simulink model "controllo_cartesiano"  (R2020b)
(part 3 of 5)

dxc5*((l*cos(2*atan((2*l^2*sin(q2) + (3*l^4 + 4*cos(q2)*l^3*xc1 - 4*sin(q2)*l^3*xc5 - 2*cos(2*q2)*l^2*xc1^2 + 4*sin(2*q2)*l^2*xc1*xc5 + 2*cos(2*q2)*l^2*xc5^2 - 4*cos(q2)*l*xc1^3 + 4*sin(q2)*l*xc1^2*xc5 - 4*cos(q2)*l*xc1*xc5^2 + 4*sin(q2)*l*xc5^3 - xc1^4 - 2*xc1^2*xc5^2 - xc5^4)^(1/2) - 2*l*xc5)/(l^2 - 2*l*xc1 + xc1^2 + xc5^2 - 2*l^2*cos(q2) + 2*l*xc1*cos(q2) - 2*l*xc5*sin(q2))))*(((cos(q2) + 1)^2*(2*xc1 - 4*l*tan(q2/2)^2 + 2*xc1*tan(q2/2)^2)*(2*l + 2*l*tan(q2/2)^2 - ((2*xc5 - 2*l*sin(q2))*(l^2 + 2*cos(q2)*l*xc1 - 2*sin(q2)*l*xc5 + xc1^2 + xc5^2) + (2*xc5 - 2*l*sin(q2))*(- 3*l^2 + 2*cos(q2)*l*xc1 - 2*sin(q2)*l*xc5 + xc1^2 + xc5^2))/((cos(q2) + 1)*(-(l^2 + 2*cos(q2)*l*xc1 - 2*sin(q2)*l*xc5 + xc1^2 + xc5^2)*(- 3*l^2 + 2*cos(q2)*l*xc1 - 2*sin(q2)*l*xc5 + xc1^2 + xc5^2))^(1/2))))/(4*(l^2 - 2*l*xc1 + xc1^2 + xc5^2 - 2*l^2*cos(q2) + 2*l*xc1*cos(q2) - 2*l*xc5*sin(q2))^2) + (2*(xc1 + l*cos(q2))*(2*xc5 - 2*l*sin(q2)))/((-(l^2 + 2*cos(q2)*l*xc1 - 2*sin(q2)*l*xc5 + xc1^2 + xc5^2)*(- 3*l^2 + 2*cos(q2)*l*xc1 - 2*sin(q2)*l*xc5 + xc1^2 + xc5^2))^(1/2)*(l^2 - 2*l*xc1 + xc1^2 + xc5^2 - 2*l^2*cos(q2) + 2*l*xc1*cos(q2) - 2*l*xc5*sin(q2))) - (l*(tan(q2/2)^2 + 1)*(cos(q2) + 1)^2*(2*xc1 - 4*l*tan(q2/2)^2 + 2*xc1*tan(q2/2)^2))/(l^2 - 2*l*xc1 + xc1^2 + xc5^2 - 2*l^2*cos(q2) + 2*l*xc1*cos(q2) - 2*l*xc5*sin(q2))^2 - (2*(xc1 + l*cos(q2))*(2*xc5 - 2*l*sin(q2))*(- l^2 + 2*cos(q2)*l*xc1 - 2*sin(q2)*l*xc5 + xc1^2 + xc5^2))/((-(l^2 + 2*cos(q2)*l*xc1 - 2*sin(q2)*l*xc5 + xc1^2 + xc5^2)*(- 3*l^2 + 2*cos(q2)*l*xc1 - 2*sin(q2)*l*xc5 + xc1^2 + xc5^2))^(1/2)*(l^2 - 2*l*xc1 + xc1^2 + xc5^2 - 2*l^2*cos(q2) + 2*l*xc1*cos(q2) - 2*l*xc5*sin(q2))^2) + ((xc1 + l*cos(q2))*((2*xc5 - 2*l*sin(q2))*(l^2 + 2*cos(q2)*l*xc1 - 2*sin(q2)*l*xc5 + xc1^2 + xc5^2) + (2*xc5 - 2*l*sin(q2))*(- 3*l^2 + 2*cos(q2)*l*xc1 - 2*sin(q2)*l*xc5 + xc1^2 + xc5^2))*(- l^2 + 2*cos(q2)*l*xc1 - 2*sin(q2)*l*xc5 + xc1^2 + xc5^2))/((-(l^2 + 2*cos(q2)*l*xc1 - 2*sin(q2)*l*xc5 + xc1^2 + xc5^2)*(- 3*l^2 + 2*cos(q2)*l*xc1 - 2*sin(q2)*l*xc5 + xc1^2 + xc5^2))^(3/2)*(l^2 - 2*l*xc1 + xc1^2 + xc5^2 - 2*l^2*cos(q2) + 2*l*xc1*cos(q2) - 2*l*xc5*sin(q2))) - ((cos(q2) + 1)^2*(2*xc5 - 2*l*sin(q2))*(2*xc1 - 4*l*tan(q2/2)^2 + 2*xc1*tan(q2/2)^2)*(2*l*xc5 + (2*(-(l^2 + 2*cos(q2)*l*xc1 - 2*sin(q2)*l*xc5 + xc1^2 + xc5^2)*(- 3*l^2 + 2*cos(q2)*l*xc1 - 2*sin(q2)*l*xc5 + xc1^2 + xc5^2))^(1/2))/(cos(q2) + 1) - 4*l^2*tan(q2/2) + 2*l*xc5*tan(q2/2)^2))/(2*(l^2 - 2*l*xc1 + xc1^2 + xc5^2 - 2*l^2*cos(q2) + 2*l*xc1*cos(q2) - 2*l*xc5*sin(q2))^3) + (2*l*(cos(q2) + 1)^2*(2*xc5 - 2*l*sin(q2))*(2*xc1 - 4*l*tan(q2/2)^2 + 2*xc1*tan(q2/2)^2)*(xc5*tan(q2/2)^2 - 2*l*tan(q2/2) + xc5))/(l^2 - 2*l*xc1 + xc1^2 + xc5^2 - 2*l^2*cos(q2) + 2*l*xc1*cos(q2) - 2*l*xc5*sin(q2))^3))/(((cos(q2) + 1)^2*(2*l*xc5 - (2*(-(l^2 + 2*cos(q2)*l*xc1 - 2*sin(q2)*l*xc5 + xc1^2 + xc5^2)*(- 3*l^2 + 2*cos(q2)*l*xc1 - 2*sin(q2)*l*xc5 + xc1^2 + xc5^2))^(1/2))/(cos(q2) + 1) - 4*l^2*tan(q2/2) + 2*l*xc5*tan(q2/2)^2)^2)/(4*(l^2 - 2*l*xc1 + xc1^2 + xc5^2 - 2*l^2*cos(q2) + 2*l*xc1*cos(q2) - 2*l*xc5*sin(q2))^2) + 1) + (l*cos(2*atan((2*l^2*sin(q2) + (3*l^4 + 4*cos(q2)*l^3*xc1 - 4*sin(q2)*l^3*xc5 - 2*cos(2*q2)*l^2*xc1^2 + 4*sin(2*q2)*l^2*xc1*xc5 + 2*cos(2*q2)*l^2*xc5^2 - 4*cos(q2)*l*xc1^3 + 4*sin(q2)*l*xc1^2*xc5 - 4*cos(q2)*l*xc1*xc5^2 + 4*sin(q2)*l*xc5^3 - xc1^4 - 2*xc1^2*xc5^2 - xc5^4)^(1/2) - 2*l*xc5)/(l^2 - 2*l*xc1 + xc1^2 + xc5^2 - 2*l^2*cos(q2) + 2*l*xc1*cos(q2) - 2*l*xc5*sin(q2))))*(((cos(q2) + 1)^2*(2*xc5 - 2*l*sin(q2))*(2*l*xc5 - (2*(-(l^2 + 2*cos(q2)*l*xc1 - 2*sin(q2)*l*xc5 + xc1^2 + xc5^2)*(- 3*l^2 + 2*cos(q2)*l*xc1 - 2*sin(q2)*l*xc5 + xc1^2 + xc5^2))^(1/2))/(cos(q2) + 1) - 4*l^2*tan(q2/2) + 2*l*xc5*tan(q2/2)^2)^2)/(2*(l^2 - 2*l*xc1 + xc1^2 + xc5^2 - 2*l^2*cos(q2) + 2*l*xc1*cos(q2) - 2*l*xc5*sin(q2))^3) - ((cos(q2) + 1)^2*(2*l + 2*l*tan(q2/2)^2 + ((2*xc5 - 2*l*sin(q2))*(l^2 + 2*cos(q2)*l*xc1 - 2*sin(q2)*l*xc5 + xc1^2 + xc5^2) + (2*xc5 - 2*l*sin(q2))*(- 3*l^2 + 2*cos(q2)*l*xc1 - 2*sin(q2)*l*xc5 + xc1^2 + xc5^2))/((cos(q2) + 1)*(-(l^2 + 2*cos(q2)*l*xc1 - 2*sin(q2)*l*xc5 + xc1^2 + xc5^2)*(- 3*l^2 + 2*cos(q2)*l*xc1 - 2*sin(q2)*l*xc5 + xc1^2 + xc5^2))^(1/2)))*(2*l*xc5 - (2*(-(l^2 + 2*cos(q2)*l*xc1 - 2*sin(q2)*l*xc5 + xc1^2 + xc5^2)*(- 3*l^2 + 2*cos(q2)*l*xc1 - 2*sin(q2)*l*xc5 + xc1^2 + xc5^2))^(1/2))/(cos(q2) + 1) - 4*l^2*tan(q2/2) + 2*l*xc5*tan(q2/2)^2))/(2*(l^2 - 2*l*xc1 + xc1^2 + xc5^2 - 2*l^2*cos(q2) + 2*l*xc1*cos(q2) - 2*l*xc5*sin(q2))^2))*(((cos(q2) + 1)^2*(2*xc1 - 4*l*tan(q2/2)^2 + 2*xc1*tan(q2/2)^2)*(2*l*xc5 + (2*(-(l^2 + 2*cos(q2)*l*xc1 - 2*sin(q2)*l*xc5 + xc1^2 + xc5^2)*(- 3*l^2 + 2*cos(q2)*l*xc1 - 2*sin(q2)*l*xc5 + xc1^2 + xc5^2))^(1/2))/(cos(q2) + 1) - 4*l^2*tan(q2/2) + 2*l*xc5*tan(q2/2)^2))/(4*(l^2 - 2*l*xc1 + xc1^2 + xc5^2 - 2*l^2*cos(q2) + 2*l*xc1*cos(q2) - 2*l*xc5*sin(q2))^2) + (2*(xc1 + l*cos(q2))*(- l^2 + 2*cos(q2)*l*xc1 - 2*sin(q2)*l*xc5 + xc1^2 + xc5^2))/((-(l^2 + 2*cos(q2)*l*xc1 - 2*sin(q2)*l*xc5 + xc1^2 + xc5^2)*(- 3*l^2 + 2*cos(q2)*l*xc1 - 2*sin(q2)*l*xc5 + xc1^2 + xc5^2))^(1/2)*(l^2 - 2*l*xc1 + xc1^2 + xc5^2 - 2*l^2*cos(q2) + 2*l*xc1*cos(q2) - 2*l*xc5*sin(q2))) - (l*(cos(q2) + 1)^2*(2*xc1 - 4*l*tan(q2/2)^2 + 2*xc1*tan(q2/2)^2)*(xc5*tan(q2/2)^2 - 2*l*tan(q2/2) + xc5))/(l^2 - 2*l*xc1 + xc1^2 + xc5^2 - 2*l^2*cos(q2) + 2*l*xc1*cos(q2) - 2*l*xc5*sin(q2))^2))/(((cos(q2) + 1)^2*(2*l*xc5 - (2*(-(l^2 + 2*cos(q2)*l*xc1 - 2*sin(q2)*l*xc5 + xc1^2 + xc5^2)*(- 3*l^2 + 2*cos(q2)*l*xc1 - 2*sin(q2)*l*xc5 + xc1^2 + xc5^2))^(1/2))/(cos(q2) + 1) - 4*l^2*tan(q2/2) + 2*l*xc5*tan(q2/2)^2)^2)/(4*(l^2 - 2*l*xc1 + xc1^2 + xc5^2 - 2*l^2*cos(q2) + 2*l*xc1*cos(q2) - 2*l*xc5*sin(q2))^2) + 1)^2 + (2*l*sin(2*atan((2*l^2*sin(q2) + (3*l^4 + 4*cos(q2)*l^3*xc1 - 4*sin(q2)*l^3*xc5 - 2*cos(2*q2)*l^2*xc1^2 + 4*sin(2*q2)*l^2*xc1*xc5 + 2*cos(2*q2)*l^2*xc5^2 - 4*cos(q2)*l*xc1^3 + 4*sin(q2)*l*xc1^2*xc5 - 4*cos(q2)*l*xc1*xc5^2 + 4*sin(q2)*l*xc5^3 - xc1^4 - 2*xc1^2*xc5^2 - xc5^4)^(1/2) - 2*l*xc5)/(l^2 - 2*l*xc1 + xc1^2 + xc5^2 - 2*l^2*cos(q2) + 2*l*xc1*cos(q2) - 2*l*xc5*sin(q2))))*((2*l + (4*sin(q2)*l^3 - 4*sin(2*q2)*l^2*xc1 - 4*cos(2*q2)*l^2*xc5 - 4*sin(q2)*l*xc1^2 + 8*cos(q2)*l*xc1*xc5 - 12*sin(q2)*l*xc5^2 + 4*xc1^2*xc5 + 4*xc5^3)/(2*(3*l^4 + 4*cos(q2)*l^3*xc1 - 4*sin(q2)*l^3*xc5 - 2*cos(2*q2)*l^2*xc1^2 + 4*sin(2*q2)*l^2*xc1*xc5 + 2*cos(2*q2)*l^2*xc5^2 - 4*cos(q2)*l*xc1^3 + 4*sin(q2)*l*xc1^2*xc5 - 4*cos(q2)*l*xc1*xc5^2 + 4*sin(q2)*l*xc5^3 - xc1^4 - 2*xc1^2*xc5^2 - xc5^4)^(1/2)))/(l^2 - 2*l*xc1 + xc1^2 + xc5^2 - 2*l^2*cos(q2) + 2*l*xc1*cos(q2) - 2*l*xc5*sin(q2)) + ((2*xc5 - 2*l*sin(q2))*(2*l^2*sin(q2) + (3*l^4 + 4*cos(q2)*l^3*xc1 - 4*sin(q2)*l^3*xc5 - 2*cos(2*q2)*l^2*xc1^2 + 4*sin(2*q2)*l^2*xc1*xc5 + 2*cos(2*q2)*l^2*xc5^2 - 4*cos(q2)*l*xc1^3 + 4*sin(q2)*l*xc1^2*xc5 - 4*cos(q2)*l*xc1*xc5^2 + 4*sin(q2)*l*xc5^3 - xc1^4 - 2*xc1^2*xc5^2 - xc5^4)^(1/2) - 2*l*xc5))/(l^2 - 2*l*xc1 + xc1^2 + xc5^2 - 2*l^2*cos(q2) + 2*l*xc1*cos(q2) - 2*l*xc5*sin(q2))^2)*(((cos(q2) + 1)^2*(2*xc1 - 4*l*tan(q2/2)^2 + 2*xc1*tan(q2/2)^2)*(2*l*xc5 + (2*(-(l^2 + 2*cos(q2)*l*xc1 - 2*sin(q2)*l*xc5 + xc1^2 + xc5^2)*(- 3*l^2 + 2*cos(q2)*l*xc1 - 2*sin(q2)*l*xc5 + xc1^2 + xc5^2))^(1/2))/(cos(q2) + 1) - 4*l^2*tan(q2/2) + 2*l*xc5*tan(q2/2)^2))/(4*(l^2 - 2*l*xc1 + xc1^2 + xc5^2 - 2*l^2*cos(q2) + 2*l*xc1*cos(q2) - 2*l*xc5*sin(q2))^2) + (2*(xc1 + l*cos(q2))*(- l^2 + 2*cos(q2)*l*xc1 - 2*sin(q2)*l*xc5 + xc1^2 + xc5^2))/((-(l^2 + 2*cos(q2)*l*xc1 - 2*sin(q2)*l*xc5 + xc1^2 + xc5^2)*(- 3*l^2 + 2*cos(q2)*l*xc1 - 2*sin(q2)*l*xc5 + xc1^2 + xc5^2))^(1/2)*(l^2 - 2*l*xc1 + xc1^2 + xc5^2 - 2*l^2*cos(q2) + 2*l*xc1*cos(q2) - 2*l*xc5*sin(q2))) - (l*(cos(q2) + 1)^2*(2*xc1 - 4*l*tan(q2/2)^2 + 2*xc1*tan(q2/2)^2)*(xc5*tan(q2/2)^2 - 2*l*tan(q2/2) + xc5))/(l^2 - 2*l*xc1 + xc1^2 + xc5^2 - 2*l^2*cos(q2) + 2*l*xc1*cos(q2) - 2*l*xc5*sin(q2))^2))/(((2*l^2*sin(q2) + (3*l^4 + 4*cos(q2)*l^3*xc1 - 4*sin(q2)*l^3*xc5 - 2*cos(2*q2)*l^2*xc1^2 + 4*sin(2*q2)*l^2*xc1*xc5 + 2*cos(2*q2)*l^2*xc5^2 - 4*cos(q2)*l*xc1^3 + 4*sin(q2)*l*xc1^2*xc5 - 4*cos(q2)*l*xc1*xc5^2 + 4*sin(q2)*l*xc5^3 - xc1^4 - 2*xc1^2*xc5^2 - xc5^4)^(1/2) - 2*l*xc5)^2/(l^2 - 2*l*xc1 + xc1^2 + xc5^2 - 2*l^2*cos(q2) + 2*l*xc1*cos(q2) - 2*l*xc5*sin(q2))^2 + 1)*(((cos(q2) + 1)^2*(2*l*xc5 - (2*(-(l^2 + 2*cos(q2)*l*xc1 - 2*sin(q2)*l*xc5 + xc1^2 + xc5^2)*(- 3*l^2 + 2*cos(q2)*l*xc1 - 2*sin(q2)*l*xc5 + xc1^2 + xc5^2))^(1/2))/(cos(q2) + 1) - 4*l^2*tan(q2/2) + 2*l*xc5*tan(q2/2)^2)^2)/(4*(l^2 - 2*l*xc1 + xc1^2 + xc5^2 - 2*l^2*cos(q2) + 2*l*xc1*cos(q2) - 2*l*xc5*sin(q2))^2) + 1))) + dq2*((l*cos(2*atan((2*l^2*sin(q2) + (3*l^4 + 4*cos(q2)*l^3*xc1 - 4*sin(q2)*l^3*xc5 - 2*cos(2*q2)*l^2*xc1^2 + 4*sin(2*q2)*l^2*xc1*xc5 + 2*cos(2*q2)*l^2*xc5^2 - 4*cos(q2)*l*xc1^3 + 4*sin(q2)*l*xc1^2*xc5 - 4*cos(q2)*l*xc1*xc5^2 + 4*sin(q2)*l*xc5^3 - xc1^4 - 2*xc1^2*xc5^2 - xc5^4)^(1/2) - 2*l*xc5)/(l^2 - 2*l*xc1 + xc1^2 + xc5^2 - 2*l^2*cos(q2) + 2*l*xc1*cos(q2) - 2*l*xc5*sin(q2))))*(((cos(q2) + 1)^2*(2*xc1 - 4*l*tan(q2/2)^2 + 2*xc1*tan(q2/2)^2)*((2*sin(q2)*(-(l^2 + 2*cos(q2)*l*xc1 - 2*sin(q2)*l*xc5 + xc1^2 + xc5^2)*(- 3*l^2 + 2*cos(q2)*l*xc1 - 2*sin(q2)*l*xc5 + xc1^2 + xc5^2))^(1/2))/(cos(q2) + 1)^2 - 4*l^2*(tan(q2/2)^2/2 + 1/2) + ((2*l*xc5*cos(q2) + 2*l*xc1*sin(q2))*(l^2 + 2*cos(q2)*l*xc1 - 2*sin(q2)*l*xc5 + xc1^2 + xc5^2) + (2*l*xc5*cos(q2) + 2*l*xc1*sin(q2))*(- 3*l^2 + 2*cos(q2)*l*xc1 - 2*sin(q2)*l*xc5 + xc1^2 + xc5^2))/((cos(q2) + 1)*(-(l^2 + 2*cos(q2)*l*xc1 - 2*sin(q2)*l*xc5 + xc1^2 + xc5^2)*(- 3*l^2 + 2*cos(q2)*l*xc1 - 2*sin(q2)*l*xc5 + xc1^2 + xc5^2))^(1/2)) + 4*l*xc5*tan(q2/2)*(tan(q2/2)^2/2 + 1/2)))/(4*(l^2 - 2*l*xc1 + xc1^2 + xc5^2 - 2*l^2*cos(q2) + 2*l*xc1*cos(q2) - 2*l*xc5*sin(q2))^2) - ((cos(q2) + 1)^2*(8*l*tan(q2/2)*(tan(q2/2)^2/2 + 1/2) - 4*xc1*tan(q2/2)*(tan(q2/2)^2/2 + 1/2))*(2*l*xc5 + (2*(-(l^2 + 2*cos(q2)*l*xc1 - 2*sin(q2)*l*xc5 + xc1^2 + xc5^2)*(- 3*l^2 + 2*cos(q2)*l*xc1 - 2*sin(q2)*l*xc5 + xc1^2 + xc5^2))^(1/2))/(cos(q2) + 1) - 4*l^2*tan(q2/2) + 2*l*xc5*tan(q2/2)^2))/(4*(l^2 - 2*l*xc1 + xc1^2 + xc5^2 - 2*l^2*cos(q2) + 2*l*xc1*cos(q2) - 2*l*xc5*sin(q2))^2) - (2*(xc1 + l*cos(q2))*(2*l*xc5*cos(q2) + 2*l*xc1*sin(q2)))/((-(l^2 + 2*cos(q2)*l*xc1 - 2*sin(q2)*l*xc5 + xc1^2 + xc5^2)*(- 3*l^2 + 2*cos(q2)*l*xc1 - 2*sin(q2)*l*xc5 + xc1^2 + xc5^2))^(1/2)*(l^2 - 2*l*xc1 + xc1^2 + xc5^2 - 2*l^2*cos(q2) + 2*l*xc1*cos(q2) - 2*l*xc5*sin(q2))) + (2*(xc1 + l*cos(q2))*(2*l*xc5*cos(q2) - 2*l^2*sin(q2) + 2*l*xc1*sin(q2))*(- l^2 + 2*cos(q2)*l*xc1 - 2*sin(q2)*l*xc5 + xc1^2 + xc5^2))/((-(l^2 + 2*cos(q2)*l*xc1 - 2*sin(q2)*l*xc5 + xc1^2 + xc5^2)*(- 3*l^2 + 2*cos(q2)*l*xc1 - 2*sin(q2)*l*xc5 + xc1^2 + xc5^2))^(1/2)*(l^2 - 2*l*xc1 + xc1^2 + xc5^2 - 2*l^2*cos(q2) + 2*l*xc1*cos(q2) - 2*l*xc5*sin(q2))^2) - (2*l*sin(q2)*(- l^2 + 2*cos(q2)*l*xc1 - 2*sin(q2)*l*xc5 + xc1^2 + xc5^2))/((-(l^2 + 2*cos(q2)*l*xc1 - 2*sin(q2)*l*xc5 + xc1^2 + xc5^2)*(- 3*l^2 + 2*cos(q2)*l*xc1 - 2*sin(q2)*l*xc5 + xc1^2 + xc5^2))^(1/2)*(l^2 - 2*l*xc1 + xc1^2 + xc5^2 - 2*l^2*cos(q2) + 2*l*xc1*cos(q2) - 2*l*xc5*sin(q2))) + (l*(2*l*(tan(q2/2)^2/2 + 1/2) - 2*xc5*tan(q2/2)*(tan(q2/2)^2/2 + 1/2))*(cos(q2) + 1)^2*(2*xc1 - 4*l*tan(q2/2)^2 + 2*xc1*tan(q2/2)^2))/(l^2 - 2*l*xc1 + xc1^2 + xc5^2 - 2*l^2*cos(q2) + 2*l*xc1*cos(q2) - 2*l*xc5*sin(q2))^2 - ((xc1 + l*cos(q2))*((2*l*xc5*cos(q2) + 2*l*xc1*sin(q2))*(l^2 + 2*cos(q2)*l*xc1 - 2*sin(q2)*l*xc5 + xc1^2 + xc5^2) + (2*l*xc5*cos(q2) + 2*l*xc1*sin(q2))*(- 3*l^2 + 2*cos(q2)*l*xc1 - 2*sin(q2)*l*xc5 + xc1^2 + xc5^2))*(- l^2 + 2*cos(q2)*l*xc1 - 2*sin(q2)*l*xc5 + xc1^2 + xc5^2))/((-(l^2 + 2*cos(q2)*l*xc1 - 2*sin(q2)*l*xc5 + xc1^2 + xc5^2)*(- 3*l^2 + 2*cos(q2)*l*xc1 - 2*sin(q2)*l*xc5 + xc1^2 + xc5^2))^(3/2)*(l^2 - 2*l*xc1 + xc1^2 + xc5^2 - 2*l^2*cos(q2) + 2*l*xc1*cos(q2) - 2*l*xc5*sin(q2))) - (sin(q2)*(cos(q2) + 1)*(2*xc1 - 4*l*tan(q2/2)^2 + 2*xc1*tan(q2/2)^2)*(2*l*xc5 + (2*(-(l^2 + 2*cos(q2)*l*xc1 - 2*sin(q2)*l*xc5 + xc1^2 + xc5^2)*(- 3*l^2 + 2*cos(q2)*l*xc1 - 2*sin(q2)*l*xc5 + xc1^2 + xc5^2))^(1/2))/(cos(q2) + 1) - 4*l^2*tan(q2/2) + 2*l*xc5*tan(q2/2)^2))/(2*(l^2 - 2*l*xc1 + xc1^2 + xc5^2 - 2*l^2*cos(q2) + 2*l*xc1*cos(q2) - 2*l*xc5*sin(q2))^2) + ((cos(q2) + 1)^2*(2*xc1 - 4*l*tan(q2/2)^2 + 2*xc1*tan(q2/2)^2)*(2*l*xc5*cos(q2) - 2*l^2*sin(q2) + 2*l*xc1*sin(q2))*(2*l*xc5 + (2*(-(l^2 + 2*cos(q2)*l*xc1 - 2*sin(q2)*l*xc5 + xc1^2 + xc5^2)*(- 3*l^2 + 2*cos(q2)*l*xc1 - 2*sin(q2)*l*xc5 + xc1^2 + xc5^2))^(1/2))/(cos(q2) + 1) - 4*l^2*tan(q2/2) + 2*l*xc5*tan(q2/2)^2))/(2*(l^2 - 2*l*xc1 + xc1^2 + xc5^2 - 2*l^2*cos(q2) + 2*l*xc1*cos(q2) - 2*l*xc5*sin(q2))^3) + (l*(cos(q2) + 1)^2*(8*l*tan(q2/2)*(tan(q2/2)^2/2 + 1/2) - 4*xc1*tan(q2/2)*(tan(q2/2)^2/2 + 1/2))*(xc5*tan(q2/2)^2 - 2*l*tan(q2/2) + xc5))/(l^2 - 2*l*xc1 + xc1^2 + xc5^2 - 2*l^2*cos(q2) + 2*l*xc1*cos(q2) - 2*l*xc5*sin(q2))^2 + (2*l*sin(q2)*(cos(q2) + 1)*(2*xc1 - 4*l*tan(q2/2)^2 + 2*xc1*tan(q2/2)^2)*(xc5*tan(q2/2)^2 - 2*l*tan(q2/2) + xc5))/(l^2 - 2*l*xc1 + xc1^2 + xc5^2 - 2*l^2*cos(q2) + 2*l*xc1*cos(q2) - 2*l*xc5*sin(q2))^2 - (2*l*(cos(q2) + 1)^2*(2*xc1 - 4*l*tan(q2/2)^2 + 2*xc1*tan(q2/2)^2)*(xc5*tan(q2/2)^2 - 2*l*tan(q2/2) + xc5)*(2*l*xc5*cos(q2) - 2*l^2*sin(q2) + 2*l*xc1*sin(q2)))/(l^2 - 2*l*xc1 + xc1^2 + xc5^2 - 2*l^2*cos(q2) + 2*l*xc1*cos(q2) - 2*l*xc5*sin(q2))^3))/(((cos(q2) + 1)^2*(2*l*xc5 - (2*(-(l^2 + 2*cos(q2)*l*xc1 - 2*sin(q2)*l*xc5 + xc1^2 + xc5^2)*(- 3*l^2 + 2*cos(q2)*l*xc1 - 2*sin(q2)*l*xc5 + xc1^2 + xc5^2))^(1/2))/(cos(q2) + 1) - 4*l^2*tan(q2/2) + 2*l*xc5*tan(q2/2)^2)^2)/(4*(l^2 - 2*l*xc1 + xc1^2 + xc5^2 - 2*l^2*cos(q2) + 2*l*xc1*cos(q2) - 2*l*xc5*sin(q2))^2) + 1) + (l*cos(2*atan((2*l^2*sin(q2) + (3*l^4 + 4*cos(q2)*l^3*xc1 - 4*sin(q2)*l^3*xc5 - 2*cos(2*q2)*l^2*xc1^2 + 4*sin(2*q2)*l^2*xc1*xc5 + 2*cos(2*q2)*l^2*xc5^2 - 4*cos(q2)*l*xc1^3 + 4*sin(q2)*l*xc1^2*xc5 - 4*cos(q2)*l*xc1*xc5^2 + 4*sin(q2)*l*xc5^3 - xc1^4 - 2*xc1^2*xc5^2 - xc5^4)^(1/2) - 2*l*xc5)/(l^2 - 2*l*xc1 + xc1^2 + xc5^2 - 2*l^2*cos(q2) + 2*l*xc1*cos(q2) - 2*l*xc5*sin(q2))))*(((cos(q2) + 1)^2*(4*l^2*(tan(q2/2)^2/2 + 1/2) + (2*sin(q2)*(-(l^2 + 2*cos(q2)*l*xc1 - 2*sin(q2)*l*xc5 + xc1^2 + xc5^2)*(- 3*l^2 + 2*cos(q2)*l*xc1 - 2*sin(q2)*l*xc5 + xc1^2 + xc5^2))^(1/2))/(cos(q2) + 1)^2 + ((2*l*xc5*cos(q2) + 2*l*xc1*sin(q2))*(l^2 + 2*cos(q2)*l*xc1 - 2*sin(q2)*l*xc5 + xc1^2 + xc5^2) + (2*l*xc5*cos(q2) + 2*l*xc1*sin(q2))*(- 3*l^2 + 2*cos(q2)*l*xc1 - 2*sin(q2)*l*xc5 + xc1^2 + xc5^2))/((cos(q2) + 1)*(-(l^2 + 2*cos(q2)*l*xc1 - 2*sin(q2)*l*xc5 + xc1^2 + xc5^2)*(- 3*l^2 + 2*cos(q2)*l*xc1 - 2*sin(q2)*l*xc5 + xc1^2 + xc5^2))^(1/2)) - 4*l*xc5*tan(q2/2)*(tan(q2/2)^2/2 + 1/2))*(2*l*xc5 - (2*(-(l^2 + 2*cos(q2)*l*xc1 - 2*sin(q2)*l*xc5 + xc1^2 + xc5^2)*(- 3*l^2 + 2*cos(q2)*l*xc1 - 2*sin(q2)*l*xc5 + xc1^2 + xc5^2))^(1/2))/(cos(q2) + 1) - 4*l^2*tan(q2/2) + 2*l*xc5*tan(q2/2)^2))/(2*(l^2 - 2*l*xc1 + xc1^2 + xc5^2 - 2*l^2*cos(q2) + 2*l*xc1*cos(q2) - 2*l*xc5*sin(q2))^2) - ((cos(q2) + 1)^2*(2*l*xc5*cos(q2) - 2*l^2*sin(q2) + 2*l*xc1*sin(q2))*(2*l*xc5 - (2*(-(l^2 + 2*cos(q2)*l*xc1 - 2*sin(q2)*l*xc5 + xc1^2 + xc5^2)*(- 3*l^2 + 2*cos(q2)*l*xc1 - 2*sin(q2)*l*xc5 + xc1^2 + xc5^2))^(1/2))/(cos(q2) + 1) - 4*l^2*tan(q2/2) + 2*l*xc5*tan(q2/2)^2)^2)/(2*(l^2 - 2*l*xc1 + xc1^2 + xc5^2 - 2*l^2*cos(q2) + 2*l*xc1*cos(q2) - 2*l*xc5*sin(q2))^3) + (sin(q2)*(cos(q2) + 1)*(2*l*xc5 - (2*(-(l^2 + 2*cos(q2)*l*xc1 - 2*sin(q2)*l*xc5 + xc1^2 + xc5^2)*(- 3*l^2 + 2*cos(q2)*l*xc1 - 2*sin(q2)*l*xc5 + xc1^2 + xc5^2))^(1/2))/(cos(q2) + 1) - 4*l^2*tan(q2/2) + 2*l*xc5*tan(q2/2)^2)^2)/(2*(l^2 - 2*l*xc1 + xc1^2 + xc5^2 - 2*l^2*cos(q2) + 2*l*xc1*cos(q2) - 2*l*xc5*sin(q2))^2))*(((cos(q2) + 1)^2*(2*xc1 - 4*l*tan(q2/2)^2 + 2*xc1*tan(q2/2)^2)*(2*l*xc5 + (2*(-(l^2 + 2*cos(q2)*l*xc1 - 2*sin(q2)*l*xc5 + xc1^2 + xc5^2)*(- 3*l^2 + 2*cos(q2)*l*xc1 - 2*sin(q2)*l*xc5 + xc1^2 + xc5^2))^(1/2))/(cos(q2) + 1) - 4*l^2*tan(q2/2) + 2*l*xc5*tan(q2/2)^2))/(4*(l^2 - 2*l*xc1 + xc1^2 + xc5^2 - 2*l^2*cos(q2) + 2*l*xc1*cos(q2) - 2*l*xc5*sin(q2))^2) + (2*(xc1 + l*cos(q2))*(- l^2 + 2*cos(q2)*l*xc1 - 2*sin(q2)*l*xc5 + xc1^2 + xc5^2))/((-(l^2 + 2*cos(q2)*l*xc1 - 2*sin(q2)*l*xc5 + xc1^2 + xc5^2)*(- 3*l^2 + 2*cos(q2)*l*xc1 - 2*sin(q2)*l*xc5 + xc1^2 + xc5^2))^(1/2)*(l^2 - 2*l*xc1 + xc1^2 + xc5^2 - 2*l^2*cos(q2) + 2*l*xc1*cos(q2) - 2*l*xc5*sin(q2))) - (l*(cos(q2) + 1)^2*(2*xc1 - 4*l*tan(q2/2)^2 + 2*xc1*tan(q2/2)^2)*(xc5*tan(q2/2)^2 - 2*l*tan(q2/2) + xc5))/(l^2 - 2*l*xc1 + xc1^2 + xc5^2 - 2*l^2*cos(q2) + 2*l*xc1*cos(q2) - 2*l*xc5*sin(q2))^2))/(((cos(q2) + 1)^2*(2*l*xc5 - (2*(-(l^2 + 2*cos(q2)*l*xc1 - 2*sin(q2)*l*xc5 + xc1^2 + xc5^2)*(- 3*l^2 + 2*cos(q2)*l*xc1 - 2*sin(q2)*l*xc5 + xc1^2 + xc5^2))^(1/2))/(cos(q2) + 1) - 4*l^2*tan(q2/2) + 2*l*xc5*tan(q2/2)^2)^2)/(4*(l^2 - 2*l*xc1 + xc1^2 + xc5^2 - 2*l^2*cos(q2) + 2*l*xc1*cos(q2) - 2*l*xc5*sin(q2))^2) + 1)^2 - (2*l*sin(2*atan((2*l^2*sin(q2) + (3*l^4 + 4*cos(q2)*l^3*xc1 - 4*sin(q2)*l^3*xc5 - 2*cos(2*q2)*l^2*xc1^2 + 4*sin(2*q2)*l^2*xc1*xc5 + 2*cos(2*q2)*l^2*xc5^2 - 4*cos(q2)*l*xc1^3 + 4*sin(q2)*l*xc1^2*xc5 - 4*cos(q2)*l*xc1*xc5^2 + 4*sin(q2)*l*xc5^3 - xc1^4 - 2*xc1^2*xc5^2 - xc5^4)^(1/2) - 2*l*xc5)/(l^2 - 2*l*xc1 + xc1^2 + xc5^2 - 2*l^2*cos(q2) + 2*l*xc1*cos(q2) - 2*l*xc5*sin(q2))))*(((- 4*sin(q2)*l^3*xc1 - 4*cos(q2)*l^3*xc5 + 4*sin(2*q2)*l^2*xc1^2 + 8*cos(2*q2)*l^2*xc1*xc5 - 4*sin(2*q2)*l^2*xc5^2 + 4*sin(q2)*l*xc1^3 + 4*cos(q2)*l*xc1^2*xc5 + 4*sin(q2)*l*xc1*xc5^2 + 4*cos(q2)*l*xc5^3)/(2*(3*l^4 + 4*cos(q2)*l^3*xc1 - 4*sin(q2)*l^3*xc5 - 2*cos(2*q2)*l^2*xc1^2 + 4*sin(2*q2)*l^2*xc1*xc5 + 2*cos(2*q2)*l^2*xc5^2 - 4*cos(q2)*l*xc1^3 + 4*sin(q2)*l*xc1^2*xc5 - 4*cos(q2)*l*xc1*xc5^2 + 4*sin(q2)*l*xc5^3 - xc1^4 - 2*xc1^2*xc5^2 - xc5^4)^(1/2)) + 2*l^2*cos(q2))/(l^2 - 2*l*xc1 + xc1^2 + xc5^2 - 2*l^2*cos(q2) + 2*l*xc1*cos(q2) - 2*l*xc5*sin(q2)) + ((2*l*xc5*cos(q2) - 2*l^2*sin(q2) + 2*l*xc1*sin(q2))*(2*l^2*sin(q2) + (3*l^4 + 4*cos(q2)*l^3*xc1 - 4*sin(q2)*l^3*xc5 - 2*cos(2*q2)*l^2*xc1^2 + 4*sin(2*q2)*l^2*xc1*xc5 + 2*cos(2*q2)*l^2*xc5^2 - 4*cos(q2)*l*xc1^3 + 4*sin(q2)*l*xc1^2*xc5 - 4*cos(q2)*l*xc1*xc5^2 + 4*sin(q2)*l*xc5^3 - xc1^4 - 2*xc1^2*xc5^2 - xc5^4)^(1/2) - 2*l*xc5))/(l^2 - 2*l*xc1 + xc1^2 + xc5^2 - 2*l^2*cos(q2) + 2*l*xc1*cos(q2) - 2*l*xc5*sin(q2))^2)*(((cos(q2) + 1)^2*(2*xc1 - 4*l*tan(q2/2)^2 + 2*xc1*tan(q2/2)^2)*(2*l*xc5 + (2*(-(l^2 + 2*cos(q2)*l*xc1 - 2*sin(q2)*l*xc5 + xc1^2 + xc5^2)*(- 3*l^2 + 2*cos(q2)*l*xc1 - 2*sin(q2)*l*xc5 + xc1^2 + xc5^2))^(1/2))/(cos(q2) + 1) - 4*l^2*tan(q2/2) + 2*l*xc5*tan(q2/2)^2))/(4*(l^2 - 2*l*xc1 + xc1^2 + xc5^2 - 2*l^2*cos(q2) + 2*l*xc1*cos(q2) - 2*l*xc5*sin(q2))^2) + (2*(xc1 + l*cos(q2))*(- l^2 + 2*cos(q2)*l*xc1 - 2*sin(q2)*l*xc5 + xc1^2 + xc5^2))/((-(l^2 + 2*cos(q2)*l*xc1 - 2*sin(q2)*l*xc5 + xc1^2 + xc5^2)*(- 3*l^2 + 2*cos(q2)*l*xc1 - 2*sin(q2)*l*xc5 + xc1^2 + xc5^2))^(1/2)*(l^2 - 2*l*xc1 + xc1^2 + xc5^2 - 2*l^2*cos(q2) + 2*l*xc1*cos(q2) - 2*l*xc5*sin(q2))) - (l*(cos(q2) + 1)^2*(2*xc1 - 4*l*tan(q2/2)^2 + 2*xc1*tan(q2/2)^2)*(xc5*tan(q2/2)^2 - 2*l*tan(q2/2) + xc5))/(l^2 - 2*l*xc1 + xc1^2 + xc5^2 - 2*l^2*cos(q2) + 2*l*xc1*cos(q2) - 2*l*xc5*sin(q2))^2))/(((2*l^2*sin(q2) + (3*l^4 + 4*cos(q2)*l^3*xc1 - 4*sin(q2)*l^3*xc5 - 2*cos(2*q2)*l^2*xc1^2 + 4*sin(2*q2)*l^2*xc1*xc5 + 2*cos(2*q2)*l^2*xc5^2 - 4*cos(q2)*l*xc1^3 + 4*sin(q2)*l*xc1^2*xc5 - 4*cos(q2)*l*xc1*xc5^2 + 4*sin(q2)*l*xc5^3 - xc1^4 - 2*xc1^2*xc5^2 - xc5^4)^(1/2) - 2*l*xc5)^2/(l^2 - 2*l*xc1 + xc1^2 + xc5^2 - 2*l^2*cos(q2) + 2*l*xc1*cos(q2) - 2*l*xc5*sin(q2))^2 + 1)*(((cos(q2) + 1)^2*(2*l*xc5 - (2*(-(l^2 + 2*cos(q2)*l*xc1 - 2*sin(q2)*l*xc5 + xc1^2 + xc5^2)*(- 3*l^2 + 2*cos(q2)*l*xc1 - 2*sin(q2)*l*xc5 + xc1^2 + xc5^2))^(1/2))/(cos(q2) + 1) - 4*l^2*tan(q2/2) + 2*l*xc5*tan(q2/2)^2)^2)/(4*(l^2 - 2*l*xc1 + xc1^2 + xc5^2 - 2*l^2*cos(q2) + 2*l*xc1*cos(q2) - 2*l*xc5*sin(q2))^2) + 1))) + dxc1*((l*cos(2*atan((2*l^2*sin(q2) + (3*l^4 + 4*cos(q2)*l^3*xc1 - 4*sin(q2)*l^3*xc5 - 2*cos(2*q2)*l^2*xc1^2 + 4*sin(2*q2)*l^2*xc1*xc5 + 2*cos(2*q2)*l^2*xc5^2 - 4*cos(q2)*l*xc1^3 + 4*sin(q2)*l*xc1^2*xc5 - 4*cos(q2)*l*xc1*xc5^2 + 4*sin(q2)*l*xc5^3 - xc1^4 - 2*xc1^2*xc5^2 - xc5^4)^(1/2) - 2*l*xc5)/(l^2 - 2*l*xc1 + xc1^2 + xc5^2 - 2*l^2*cos(q2) + 2*l*xc1*cos(q2) - 2*l*xc5*sin(q2))))*((2*(- l^2 + 2*cos(q2)*l*xc1 - 2*sin(q2)*l*xc5 + xc1^2 + xc5^2))/((-(l^2 + 2*cos(q2)*l*xc1 - 2*sin(q2)*l*xc5 + xc1^2 + xc5^2)*(- 3*l^2 + 2*cos(q2)*l*xc1 - 2*sin(q2)*l*xc5 + xc1^2 + xc5^2))^(1/2)*(l^2 - 2*l*xc1 + xc1^2 + xc5^2 - 2*l^2*cos(q2) + 2*l*xc1*cos(q2) - 2*l*xc5*sin(q2))) + ((cos(q2) + 1)^2*(2*tan(q2/2)^2 + 2)*(2*l*xc5 + (2*(-(l^2 + 2*cos(q2)*l*xc1 - 2*sin(q2)*l*xc5 + xc1^2 + xc5^2)*(- 3*l^2 + 2*cos(q2)*l*xc1 - 2*sin(q2)*l*xc5 + xc1^2 + xc5^2))^(1/2))/(cos(q2) + 1) - 4*l^2*tan(q2/2) + 2*l*xc5*tan(q2/2)^2))/(4*(l^2 - 2*l*xc1 + xc1^2 + xc5^2 - 2*l^2*cos(q2) + 2*l*xc1*cos(q2) - 2*l*xc5*sin(q2))^2) + (2*(xc1 + l*cos(q2))*(2*xc1 + 2*l*cos(q2)))/((-(l^2 + 2*cos(q2)*l*xc1 - 2*sin(q2)*l*xc5 + xc1^2 + xc5^2)*(- 3*l^2 + 2*cos(q2)*l*xc1 - 2*sin(q2)*l*xc5 + xc1^2 + xc5^2))^(1/2)*(l^2 - 2*l*xc1 + xc1^2 + xc5^2 - 2*l^2*cos(q2) + 2*l*xc1*cos(q2) - 2*l*xc5*sin(q2))) - (2*(xc1 + l*cos(q2))*(2*xc1 - 2*l + 2*l*cos(q2))*(- l^2 + 2*cos(q2)*l*xc1 - 2*sin(q2)*l*xc5 + xc1^2 + xc5^2))/((-(l^2 + 2*cos(q2)*l*xc1 - 2*sin(q2)*l*xc5 + xc1^2 + xc5^2)*(- 3*l^2 + 2*cos(q2)*l*xc1 - 2*sin(q2)*l*xc5 + xc1^2 + xc5^2))^(1/2)*(l^2 - 2*l*xc1 + xc1^2 + xc5^2 - 2*l^2*cos(q2) + 2*l*xc1*cos(q2) - 2*l*xc5*sin(q2))^2) - ((cos(q2) + 1)*((2*xc1 + 2*l*cos(q2))*(l^2 + 2*cos(q2)*l*xc1 - 2*sin(q2)*l*xc5 + xc1^2 + xc5^2) + (2*xc1 + 2*l*cos(q2))*(- 3*l^2 + 2*cos(q2)*l*xc1 - 2*sin(q2)*l*xc5 + xc1^2 + xc5^2))*(2*xc1 - 4*l*tan(q2/2)^2 + 2*xc1*tan(q2/2)^2))/(4*(-(l^2 + 2*cos(q2)*l*xc1 - 2*sin(q2)*l*xc5 + xc1^2 + xc5^2)*(- 3*l^2 + 2*cos(q2)*l*xc1 - 2*sin(q2)*l*xc5 + xc1^2 + xc5^2))^(1/2)*(l^2 - 2*l*xc1 + xc1^2 + xc5^2 - 2*l^2*cos(q2) + 2*l*xc1*cos(q2) - 2*l*xc5*sin(q2))^2) - ((cos(q2) + 1)^2*(2*xc1 - 4*l*tan(q2/2)^2 + 2*xc1*tan(q2/2)^2)*(2*xc1 - 2*l + 2*l*cos(q2))*(2*l*xc5 + (2*(-(l^2 + 2*cos(q2)*l*xc1 - 2*sin(q2)*l*xc5 + xc1^2 + xc5^2)*(- 3*l^2 + 2*cos(q2)*l*xc1 - 2*sin(q2)*l*xc5 + xc1^2 + xc5^2))^(1/2))/(cos(q2) + 1) - 4*l^2*tan(q2/2) + 2*l*xc5*tan(q2/2)^2))/(2*(l^2 - 2*l*xc1 + xc1^2 + xc5^2 - 2*l^2*cos(q2) + 2*l*xc1*cos(q2) - 2*l*xc5*sin(q2))^3) + (((2*xc1 + 2*l*cos(q2))*(l^2 + 2*cos(q2)*l*xc1 - 2*sin(q2)*l*xc5 + xc1^2 + xc5^2) + (2*xc1 + 2*l*cos(q2))*(- 3*l^2 + 2*cos(q2)*l*xc1 - 2*sin(q2)*l*xc5 + xc1^2 + xc5^2))*(xc1 + l*cos(q2))*(- l^2 + 2*cos(q2)*l*xc1 - 2*sin(q2)*l*xc5 + xc1^2 + xc5^2))/((-(l^2 + 2*cos(q2)*l*xc1 - 2*sin(q2)*l*xc5 + xc1^2 + xc5^2)*(- 3*l^2 + 2*cos(q2)*l*xc1 - 2*sin(q2)*l*xc5 + xc1^2 + xc5^2))^(3/2)*(l^2 - 2*l*xc1 + xc1^2 + xc5^2 - 2*l^2*cos(q2) + 2*l*xc1*cos(q2) - 2*l*xc5*sin(q2))) - (l*(cos(q2) + 1)^2*(2*tan(q2/2)^2 + 2)*(xc5*tan(q2/2)^2 - 2*l*tan(q2/2) + xc5))/(l^2 - 2*l*xc1 + xc1^2 + xc5^2 - 2*l^2*cos(q2) + 2*l*xc1*cos(q2) - 2*l*xc5*sin(q2))^2 + (2*l*(cos(q2) + 1)^2*(2*xc1 - 4*l*tan(q2/2)^2 + 2*xc1*tan(q2/2)^2)*(xc5*tan(q2/2)^2 - 2*l*tan(q2/2) + xc5)*(2*xc1 - 2*l + 2*l*cos(q2)))/(l^2 - 2*l*xc1 + xc1^2 + xc5^2 - 2*l^2*cos(q2) + 2*l*xc1*cos(q2) - 2*l*xc5*sin(q2))^3))/(((cos(q2) + 1)^2*(2*l*xc5 - (2*(-(l^2 + 2*cos(q2)*l*xc1 - 2*sin(q2)*l*xc5 + xc1^2 + xc5^2)*(- 3*l^2 + 2*cos(q2)*l*xc1 - 2*sin(q2)*l*xc5 + xc1^2 + xc5^2))^(1/2))/(cos(q2) + 1) - 4*l^2*tan(q2/2) + 2*l*xc5*tan(q2/2)^2)^2)/(4*(l^2 - 2*l*xc1 + xc1^2 + xc5^2 - 2*l^2*cos(q2) + 2*l*xc1*cos(q2) - 2*l*xc5*sin(q2))^2) + 1) + (l*cos(2*atan((2*l^2*sin(q2) + (3*l^4 + 4*cos(q2)*l^3*xc1 - 4*sin(q2)*l^3*xc5 - 2*cos(2*q2)*l^2*xc1^2 + 4*sin(2*q2)*l^2*xc1*xc5 + 2*cos(2*q2)*l^2*xc5^2 - 4*cos(q2)*l*xc1^3 + 4*sin(q2)*l*xc1^2*xc5 - 4*cos(q2)*l*xc1*xc5^2 + 4*sin(q2)*l*xc5^3 - xc1^4 - 2*xc1^2*xc5^2 - xc5^4)^(1/2) - 2*l*xc5)/(l^2 - 2*l*xc1 + xc1^2 + xc5^2 - 2*l^2*cos(q2) + 2*l*xc1*cos(q2) - 2*l*xc5*sin(q2))))*(((cos(q2) + 1)^2*(2*xc1 - 2*l + 2*l*cos(q2))*(2*l*xc5 - (2*(-(l^2 + 2*cos(q2)*l*xc1 - 2*sin(q2)*l*xc5 + xc1^2 + xc5^2)*(- 3*l^2 + 2*cos(q2)*l*xc1 - 2*sin(q2)*l*xc5 + xc1^2 + xc5^2))^(1/2))/(cos(q2) + 1) - 4*l^2*tan(q2/2) + 2*l*xc5*tan(q2/2)^2)^2)/(2*(l^2 - 2*l*xc1 + xc1^2 + xc5^2 - 2*l^2*cos(q2) + 2*l*xc1*cos(q2) - 2*l*xc5*sin(q2))^3) - ((cos(q2) + 1)*((2*xc1 + 2*l*cos(q2))*(l^2 + 2*cos(q2)*l*xc1 - 2*sin(q2)*l*xc5 + xc1^2 + xc5^2) + (2*xc1 + 2*l*cos(q2))*(- 3*l^2 + 2*cos(q2)*l*xc1 - 2*sin(q2)*l*xc5 + xc1^2 + xc5^2))*(2*l*xc5 - (2*(-(l^2 + 2*cos(q2)*l*xc1 - 2*sin(q2)*l*xc5 + xc1^2 + xc5^2)*(- 3*l^2 + 2*cos(q2)*l*xc1 - 2*sin(q2)*l*xc5 + xc1^2 + xc5^2))^(1/2))/(cos(q2) + 1) - 4*l^2*tan(q2/2) + 2*l*xc5*tan(q2/2)^2))/(2*(-(l^2 + 2*cos(q2)*l*xc1 - 2*sin(q2)*l*xc5 + xc1^2 + xc5^2)*(- 3*l^2 + 2*cos(q2)*l*xc1 - 2*sin(q2)*l*xc5 + xc1^2 + xc5^2))^(1/2)*(l^2 - 2*l*xc1 + xc1^2 + xc5^2 - 2*l^2*cos(q2) + 2*l*xc1*cos(q2) - 2*l*xc5*sin(q2))^2))*(((cos(q2) + 1)^2*(2*xc1 - 4*l*tan(q2/2)^2 + 2*xc1*tan(q2/2)^2)*(2*l*xc5 + (2*(-(l^2 + 2*cos(q2)*l*xc1 - 2*sin(q2)*l*xc5 + xc1^2 + xc5^2)*(- 3*l^2 + 2*cos(q2)*l*xc1 - 2*sin(q2)*l*xc5 + xc1^2 + xc5^2))^(1/2))/(cos(q2) + 1) - 4*l^2*tan(q2/2) + 2*l*xc5*tan(q2/2)^2))/(4*(l^2 - 2*l*xc1 + xc1^2 + xc5^2 - 2*l^2*cos(q2) + 2*l*xc1*cos(q2) - 2*l*xc5*sin(q2))^2) + (2*(xc1 + l*cos(q2))*(- l^2 + 2*cos(q2)*l*xc1 - 2*sin(q2)*l*xc5 + xc1^2 + xc5^2))/((-(l^2 + 2*cos(q2)*l*xc1 - 2*sin(q2)*l*xc5 + xc1^2 + xc5^2)*(- 3*l^2 + 2*cos(q2)*l*xc1 - 2*sin(q2)*l*xc5 + xc1^2 + xc5^2))^(1/2)*(l^2 - 2*l*xc1 + xc1^2 + xc5^2 - 2*l^2*cos(q2) + 2*l*xc1*cos(q2) - 2*l*xc5*sin(q2))) - (l*(cos(q2) + 1)^2*(2*xc1 - 4*l*tan(q2/2)^2 + 2*xc1*tan(q2/2)^2)*(xc5*tan(q2/2)^2 - 2*l*tan(q2/2) + xc5))/(l^2 - 2*l*xc1 + xc1^2 + xc5^2 - 2*l^2*cos(q2) + 2*l*xc1*cos(q2) - 2*l*xc5*sin(q2))^2))/(((cos(q2) + 1)^2*(2*l*xc5 - (2*(-(l^2 + 2*cos(q2)*l*xc1 - 2*sin(q2)*l*xc5 + xc1^2 + xc5^2)*(- 3*l^2 + 2*cos(q2)*l*xc1 - 2*sin(q2)*l*xc5 + xc1^2 + xc5^2))^(1/2))/(cos(q2) + 1) - 4*l^2*tan(q2/2) + 2*l*xc5*tan(q2/2)^2)^2)/(4*(l^2 - 2*l*xc1 + xc1^2 + xc5^2 - 2*l^2*cos(q2) + 2*l*xc1*cos(q2) - 2*l*xc5*sin(q2))^2) + 1)^2 + (2*l*sin(2*atan((2*l^2*sin(q2) + (3*l^4 + 4*cos(q2)*l^3*xc1 - 4*sin(q2)*l^3*xc5 - 2*cos(2*q2)*l^2*xc1^2 + 4*sin(2*q2)*l^2*xc1*xc5 + 2*cos(2*q2)*l^2*xc5^2 - 4*cos(q2)*l*xc1^3 + 4*sin(q2)*l*xc1^2*xc5 - 4*cos(q2)*l*xc1*xc5^2 + 4*sin(q2)*l*xc5^3 - xc1^4 - 2*xc1^2*xc5^2 - xc5^4)^(1/2) - 2*l*xc5)/(l^2 - 2*l*xc1 + xc1^2 + xc5^2 - 2*l^2*cos(q2) + 2*l*xc1*cos(q2) - 2*l*xc5*sin(q2))))*(((2*xc1 - 2*l + 2*l*cos(q2))*(2*l^2*sin(q2) + (3*l^4 + 4*cos(q2)*l^3*xc1 - 4*sin(q2)*l^3*xc5 - 2*cos(2*q2)*l^2*xc1^2 + 4*sin(2*q2)*l^2*xc1*xc5 + 2*cos(2*q2)*l^2*xc5^2 - 4*cos(q2)*l*xc1^3 + 4*sin(q2)*l*xc1^2*xc5 - 4*cos(q2)*l*xc1*xc5^2 + 4*sin(q2)*l*xc5^3 - xc1^4 - 2*xc1^2*xc5^2 - xc5^4)^(1/2) - 2*l*xc5))/(l^2 - 2*l*xc1 + xc1^2 + xc5^2 - 2*l^2*cos(q2) + 2*l*xc1*cos(q2) - 2*l*xc5*sin(q2))^2 + (- 4*cos(q2)*l^3 + 4*cos(2*q2)*l^2*xc1 - 4*sin(2*q2)*l^2*xc5 + 12*cos(q2)*l*xc1^2 - 8*sin(q2)*l*xc1*xc5 + 4*cos(q2)*l*xc5^2 + 4*xc1^3 + 4*xc1*xc5^2)/(2*(l^2 - 2*l*xc1 + xc1^2 + xc5^2 - 2*l^2*cos(q2) + 2*l*xc1*cos(q2) - 2*l*xc5*sin(q2))*(3*l^4 + 4*cos(q2)*l^3*xc1 - 4*sin(q2)*l^3*xc5 - 2*cos(2*q2)*l^2*xc1^2 + 4*sin(2*q2)*l^2*xc1*xc5 + 2*cos(2*q2)*l^2*xc5^2 - 4*cos(q2)*l*xc1^3 + 4*sin(q2)*l*xc1^2*xc5 - 4*cos(q2)*l*xc1*xc5^2 + 4*sin(q2)*l*xc5^3 - xc1^4 - 2*xc1^2*xc5^2 - xc5^4)^(1/2)))*(((cos(q2) + 1)^2*(2*xc1 - 4*l*tan(q2/2)^2 + 2*xc1*tan(q2/2)^2)*(2*l*xc5 + (2*(-(l^2 + 2*cos(q2)*l*xc1 - 2*sin(q2)*l*xc5 + xc1^2 + xc5^2)*(- 3*l^2 + 2*cos(q2)*l*xc1 - 2*sin(q2)*l*xc5 + xc1^2 + xc5^2))^(1/2))/(cos(q2) + 1) - 4*l^2*tan(q2/2) + 2*l*xc5*tan(q2/2)^2))/(4*(l^2 - 2*l*xc1 + xc1^2 + xc5^2 - 2*l^2*cos(q2) + 2*l*xc1*cos(q2) - 2*l*xc5*sin(q2))^2) + (2*(xc1 + l*cos(q2))*(- l^2 + 2*cos(q2)*l*xc1 - 2*sin(q2)*l*xc5 + xc1^2 + xc5^2))/((-(l^2 + 2*cos(q2)*l*xc1 - 2*sin(q2)*l*xc5 + xc1^2 + xc5^2)*(- 3*l^2 + 2*cos(q2)*l*xc1 - 2*sin(q2)*l*xc5 + xc1^2 + xc5^2))^(1/2)*(l^2 - 2*l*xc1 + xc1^2 + xc5^2 - 2*l^2*cos(q2) + 2*l*xc1*cos(q2) - 2*l*xc5*sin(q2))) - (l*(cos(q2) + 1)^2*(2*xc1 - 4*l*tan(q2/2)^2 + 2*xc1*tan(q2/2)^2)*(xc5*tan(q2/2)^2 - 2*l*tan(q2/2) + xc5))/(l^2 - 2*l*xc1 + xc1^2 + xc5^2 - 2*l^2*cos(q2) + 2*l*xc1*cos(q2) - 2*l*xc5*sin(q2))^2))/(((2*l^2*sin(q2) + (3*l^4 + 4*cos(q2)*l^3*xc1 - 4*sin(q2)*l^3*xc5 - 2*cos(2*q2)*l^2*xc1^2 + 4*sin(2*q2)*l^2*xc1*xc5 + 2*cos(2*q2)*l^2*xc5^2 - 4*cos(q2)*l*xc1^3 + 4*sin(q2)*l*xc1^2*xc5 - 4*cos(q2)*l*xc1*xc5^2 + 4*sin(q2)*l*xc5^3 - xc1^4 - 2*xc1^2*xc5^2 - xc5^4)^(1/2) - 2*l*xc5)^2/(l^2 - 2*l*xc1 + xc1^2 + xc5^2 - 2*l^2*cos(q2) + 2*l*xc1*cos(q2) - 2*l*xc5*sin(q2))^2 + 1)*(((cos(q2) + 1)^2*(2*l*xc5 - (2*(-(l^2 + 2*cos(q2)*l*xc1 - 2*sin(q2)*l*xc5 + xc1^2 + xc5^2)*(- 3*l^2 + 2*cos(q2)*l*xc1 - 2*sin(q2)*l*xc5 + xc1^2 + xc5^2))^(1/2))/(cos(q2) + 1) - 4*l^2*tan(q2/2) + 2*l*xc5*tan(q2/2)^2)^2)/(4*(l^2 - 2*l*xc1 + xc1^2 + xc5^2 - 2*l^2*cos(q2) + 2*l*xc1*cos(q2) - 2*l*xc5*sin(q2))^2) + 1))), dxc5*((l*cos(2*atan((2*l^2*sin(q2) + (3*l^4 + 4*cos(q2)*l^3*xc1 - 4*sin(q2)*l^3*xc5 - 2*cos(2*q2)*l^2*xc1^2 + 4*sin(2*q2)*l^2*xc1*xc5 + 2*cos(2*q2)*l^2*xc5^2 - 4*cos(q2)*l*xc1^3 + 4*sin(q2)*l*xc1^2*xc5 - 4*cos(q2)*l*xc1*xc5^2 + 4*sin(q2)*l*xc5^3 - xc1^4 - 2*xc1^2*xc5^2 - xc5^4)^(1/2) - 2*l*xc5)/(l^2 - 2*l*xc1 + xc1^2 + xc5^2 - 2*l^2*cos(q2) + 2*l*xc1*cos(q2) - 2*l*xc5*sin(q2))))*(((cos(q2) + 1)*((4*((1 - 2*cos(q2)^2)*l^2 + 2*cos(q2)*l*xc1 - 6*sin(q2)*l*xc5 + xc1^2 + 3*xc5^2))/((cos(q2) + 1)*(-(l^2 + 2*cos(q2)*l*xc1 - 2*sin(q2)*l*xc5 + xc1^2 + xc5^2)*(- 3*l^2 + 2*cos(q2)*l*xc1 - 2*sin(q2)*l*xc5 + xc1^2 + xc5^2))^(1/2)) + (2*((2*xc5 - 2*l*sin(q2))*(l^2 + 2*cos(q2)*l*xc1 - 2*sin(q2)*l*xc5 + xc1^2 + xc5^2) + (2*xc5 - 2*l*sin(q2))*(- 3*l^2 + 2*cos(q2)*l*xc1 - 2*sin(q2)*l*xc5 + xc1^2 + xc5^2))*(sin(q2)*l^3 - 2*cos(q2)*sin(q2)*l^2*xc1 + (1 - 2*cos(q2)^2)*l^2*xc5 - sin(q2)*l*xc1^2 + 2*cos(q2)*l*xc1*xc5 - 3*sin(q2)*l*xc5^2 + xc1^2*xc5 + xc5^3))/((cos(q2) + 1)*(-(l^2 + 2*cos(q2)*l*xc1 - 2*sin(q2)*l*xc5 + xc1^2 + xc5^2)*(- 3*l^2 + 2*cos(q2)*l*xc1 - 2*sin(q2)*l*xc5 + xc1^2 + xc5^2))^(3/2))))/(2*(l^2 - 2*l*xc1 + xc1^2 + xc5^2 - 2*l^2*cos(q2) + 2*l*xc1*cos(q2) - 2*l*xc5*sin(q2))) - (4*l*(2*xc5 - 2*l*sin(q2)))/(l^2 - 2*l*xc1 + xc1^2 + xc5^2 - 2*l^2*cos(q2) + 2*l*xc1*cos(q2) - 2*l*xc5*sin(q2))^2 + ((cos(q2) + 1)^2*(2*tan(q2/2)^2 + 2)*(2*l*xc5 + (2*(-(l^2 + 2*cos(q2)*l*xc1 - 2*sin(q2)*l*xc5 + xc1^2 + xc5^2)*(- 3*l^2 + 2*cos(q2)*l*xc1 - 2*sin(q2)*l*xc5 + xc1^2 + xc5^2))^(1/2))/(cos(q2) + 1) - 4*l^2*tan(q2/2) + 2*l*xc5*tan(q2/2)^2))/(4*(l^2 - 2*l*xc1 + xc1^2 + xc5^2 - 2*l^2*cos(q2) + 2*l*xc1*cos(q2) - 2*l*xc5*sin(q2))^2) + ((cos(q2) + 1)*(2*xc5 - 2*l*sin(q2))*(2*l + 2*l*tan(q2/2)^2 - (4*(sin(q2)*l^3 - 2*cos(q2)*sin(q2)*l^2*xc1 + (1 - 2*cos(q2)^2)*l^2*xc5 - sin(q2)*l*xc1^2 + 2*cos(q2)*l*xc1*xc5 - 3*sin(q2)*l*xc5^2 + xc1^2*xc5 + xc5^3))/((cos(q2) + 1)*(-(l^2 + 2*cos(q2)*l*xc1 - 2*sin(q2)*l*xc5 + xc1^2 + xc5^2)*(- 3*l^2 + 2*cos(q2)*l*xc1 - 2*sin(q2)*l*xc5 + xc1^2 + xc5^2))^(1/2))))/(2*(l^2 - 2*l*xc1 + xc1^2 + xc5^2 - 2*l^2*cos(q2) + 2*l*xc1*cos(q2) - 2*l*xc5*sin(q2))^2) + ((cos(q2) + 1)^2*(2*l + 2*l*tan(q2/2)^2 - ((2*xc5 - 2*l*sin(q2))*(l^2 + 2*cos(q2)*l*xc1 - 2*sin(q2)*l*xc5 + xc1^2 + xc5^2) + (2*xc5 - 2*l*sin(q2))*(- 3*l^2 + 2*cos(q2)*l*xc1 - 2*sin(q2)*l*xc5 + xc1^2 + xc5^2))/((cos(q2) + 1)*(-(l^2 + 2*cos(q2)*l*xc1 - 2*sin(q2)*l*xc5 + xc1^2 + xc5^2)*(- 3*l^2 + 2*cos(q2)*l*xc1 - 2*sin(q2)*l*xc5 + xc1^2 + xc5^2))^(1/2)))*(2*xc5*tan(q2/2)^2 - 4*l*tan(q2/2) + 2*xc5))/(4*(l^2 - 2*l*xc1 + xc1^2 + xc5^2 - 2*l^2*cos(q2) + 2*l*xc1*cos(q2) - 2*l*xc5*sin(q2))^2) - ((cos(q2) + 1)^2*(2*xc5 - 2*l*sin(q2))*(2*xc5*tan(q2/2)^2 - 4*l*tan(q2/2) + 2*xc5)*(2*l*xc5 + (2*(-(l^2 + 2*cos(q2)*l*xc1 - 2*sin(q2)*l*xc5 + xc1^2 + xc5^2)*(- 3*l^2 + 2*cos(q2)*l*xc1 - 2*sin(q2)*l*xc5 + xc1^2 + xc5^2))^(1/2))/(cos(q2) + 1) - 4*l^2*tan(q2/2) + 2*l*xc5*tan(q2/2)^2))/(2*(l^2 - 2*l*xc1 + xc1^2 + xc5^2 - 2*l^2*cos(q2) + 2*l*xc1*cos(q2) - 2*l*xc5*sin(q2))^3) - (l*(cos(q2) + 1)^2*(2*tan(q2/2)^2 + 2)*(xc5*tan(q2/2)^2 - 2*l*tan(q2/2) + xc5))/(l^2 - 2*l*xc1 + xc1^2 + xc5^2 - 2*l^2*cos(q2) + 2*l*xc1*cos(q2) - 2*l*xc5*sin(q2))^2 - (l*(tan(q2/2)^2 + 1)*(cos(q2) + 1)^2*(2*xc5*tan(q2/2)^2 - 4*l*tan(q2/2) + 2*xc5))/(l^2 - 2*l*xc1 + xc1^2 + xc5^2 - 2*l^2*cos(q2) + 2*l*xc1*cos(q2) - 2*l*xc5*sin(q2))^2 + (2*l*(cos(q2) + 1)^2*(2*xc5 - 2*l*sin(q2))*(xc5*tan(q2/2)^2 - 2*l*tan(q2/2) + xc5)*(2*xc5*tan(q2/2)^2 - 4*l*tan(q2/2) + 2*xc5))/(l^2 - 2*l*xc1 + xc1^2 + xc5^2 - 2*l^2*cos(q2) + 2*l*xc1*cos(q2) - 2*l*xc5*sin(q2))^3))/(((cos(q2) + 1)^2*(2*l*xc5 - (2*(-(l^2 + 2*cos(q2)*l*xc1 - 2*sin(q2)*l*xc5 + xc1^2 + xc5^2)*(- 3*l^2 + 2*cos(q2)*l*xc1 - 2*sin(q2)*l*xc5 + xc1^2 + xc5^2))^(1/2))/(cos(q2) + 1) - 4*l^2*tan(q2/2) + 2*l*xc5*tan(q2/2)^2)^2)/(4*(l^2 - 2*l*xc1 + xc1^2 + xc5^2 - 2*l^2*cos(q2) + 2*l*xc1*cos(q2) - 2*l*xc5*sin(q2))^2) + 1) + (l*cos(2*atan((2*l^2*sin(q2) + (3*l^4 + 4*cos(q2)*l^3*xc1 - 4*sin(q2)*l^3*xc5 - 2*cos(2*q2)*l^2*xc1^2 + 4*sin(2*q2)*l^2*xc1*xc5 + 2*cos(2*q2)*l^2*xc5^2 - 4*cos(q2)*l*xc1^3 + 4*sin(q2)*l*xc1^2*xc5 - 4*cos(q2)*l*xc1*xc5^2 + 4*sin(q2)*l*xc5^3 - xc1^4 - 2*xc1^2*xc5^2 - xc5^4)^(1/2) - 2*l*xc5)/(l^2 - 2*l*xc1 + xc1^2 + xc5^2 - 2*l^2*cos(q2) + 2*l*xc1*cos(q2) - 2*l*xc5*sin(q2))))*(((cos(q2) + 1)^2*(2*xc5 - 2*l*sin(q2))*(2*l*xc5 - (2*(-(l^2 + 2*cos(q2)*l*xc1 - 2*sin(q2)*l*xc5 + xc1^2 + xc5^2)*(- 3*l^2 + 2*cos(q2)*l*xc1 - 2*sin(q2)*l*xc5 + xc1^2 + xc5^2))^(1/2))/(cos(q2) + 1) - 4*l^2*tan(q2/2) + 2*l*xc5*tan(q2/2)^2)^2)/(2*(l^2 - 2*l*xc1 + xc1^2 + xc5^2 - 2*l^2*cos(q2) + 2*l*xc1*cos(q2) - 2*l*xc5*sin(q2))^3) - ((cos(q2) + 1)^2*(2*l + 2*l*tan(q2/2)^2 + ((2*xc5 - 2*l*sin(q2))*(l^2 + 2*cos(q2)*l*xc1 - 2*sin(q2)*l*xc5 + xc1^2 + xc5^2) + (2*xc5 - 2*l*sin(q2))*(- 3*l^2 + 2*cos(q2)*l*xc1 - 2*sin(q2)*l*xc5 + xc1^2 + xc5^2))/((cos(q2) + 1)*(-(l^2 + 2*cos(q2)*l*xc1 - 2*sin(q2)*l*xc5 + xc1^2 + xc5^2)*(- 3*l^2 + 2*cos(q2)*l*xc1 - 2*sin(q2)*l*xc5 + xc1^2 + xc5^2))^(1/2)))*(2*l*xc5 - (2*(-(l^2 + 2*cos(q2)*l*xc1 - 2*sin(q2)*l*xc5 + xc1^2 + xc5^2)*(- 3*l^2 + 2*cos(q2)*l*xc1 - 2*sin(q2)*l*xc5 + xc1^2 + xc5^2))^(1/2))/(cos(q2) + 1) - 4*l^2*tan(q2/2) + 2*l*xc5*tan(q2/2)^2))/(2*(l^2 - 2*l*xc1 + xc1^2 + xc5^2 - 2*l^2*cos(q2) + 2*l*xc1*cos(q2) - 2*l*xc5*sin(q2))^2))*((4*l)/(l^2 - 2*l*xc1 + xc1^2 + xc5^2 - 2*l^2*cos(q2) + 2*l*xc1*cos(q2) - 2*l*xc5*sin(q2)) - ((cos(q2) + 1)*(2*l + 2*l*tan(q2/2)^2 - (4*(sin(q2)*l^3 - 2*cos(q2)*sin(q2)*l^2*xc1 + (1 - 2*cos(q2)^2)*l^2*xc5 - sin(q2)*l*xc1^2 + 2*cos(q2)*l*xc1*xc5 - 3*sin(q2)*l*xc5^2 + xc1^2*xc5 + xc5^3))/((cos(q2) + 1)*(-(l^2 + 2*cos(q2)*l*xc1 - 2*sin(q2)*l*xc5 + xc1^2 + xc5^2)*(- 3*l^2 + 2*cos(q2)*l*xc1 - 2*sin(q2)*l*xc5 + xc1^2 + xc5^2))^(1/2))))/(2*(l^2 - 2*l*xc1 + xc1^2 + xc5^2 - 2*l^2*cos(q2) + 2*l*xc1*cos(q2) - 2*l*xc5*sin(q2))) + ((cos(q2) + 1)^2*(2*xc5*tan(q2/2)^2 - 4*l*tan(q2/2) + 2*xc5)*(2*l*xc5 + (2*(-(l^2 + 2*cos(q2)*l*xc1 - 2*sin(q2)*l*xc5 + xc1^2 + xc5^2)*(- 3*l^2 + 2*cos(q2)*l*xc1 - 2*sin(q2)*l*xc5 + xc1^2 + xc5^2))^(1/2))/(cos(q2) + 1) - 4*l^2*tan(q2/2) + 2*l*xc5*tan(q2/2)^2))/(4*(l^2 - 2*l*xc1 + xc1^2 + xc5^2 - 2*l^2*cos(q2) + 2*l*xc1*cos(q2) - 2*l*xc5*sin(q2))^2) - (l*(cos(q2) + 1)^2*(xc5*tan(q2/2)^2 - 2*l*tan(q2/2) + xc5)*(2*xc5*tan(q2/2)^2 - 4*l*tan(q2/2) + 2*xc5))/(l^2 - 2*l*xc1 + xc1^2 + xc5^2 - 2*l^2*cos(q2) + 2*l*xc1*cos(q2) - 2*l*xc5*sin(q2))^2))/(((cos(q2) + 1)^2*(2*l*xc5 - (2*(-(l^2 + 2*cos(q2)*l*xc1 - 2*sin(q2)*l*xc5 + xc1^2 + xc5^2)*(- 3*l^2 + 2*cos(q2)*l*xc1 - 2*sin(q2)*l*xc5 + xc1^2 + xc5^2))^(1/2))/(cos(q2) + 1) - 4*l^2*tan(q2/2) + 2*l*xc5*tan(q2/2)^2)^2)/(4*(l^2 - 2*l*xc1 + xc1^2 + xc5^2 - 2*l^2*cos(q2) + 2*l*xc1*cos(q2) - 2*l*xc5*sin(q2))^2) + 1)^2 + (2*l*sin(2*atan((2*l^2*sin(q2) + (3*l^4 + 4*cos(q2)*l^3*xc1 - 4*sin(q2)*l^3*xc5 - 2*cos(2*q2)*l^2*xc1^2 + 4*sin(2*q2)*l^2*xc1*xc5 + 2*cos(2*q2)*l^2*xc5^2 - 4*cos(q2)*l*xc1^3 + 4*sin(q2)*l*xc1^2*xc5 - 4*cos(q2)*l*xc1*xc5^2 + 4*sin(q2)*l*xc5^3 - xc1^4 - 2*xc1^2*xc5^2 - xc5^4)^(1/2) - 2*l*xc5)/(l^2 - 2*l*xc1 + xc1^2 + xc5^2 - 2*l^2*cos(q2) + 2*l*xc1*cos(q2) - 2*l*xc5*sin(q2))))*((2*l + (4*sin(q2)*l^3 - 4*sin(2*q2)*l^2*xc1 - 4*cos(2*q2)*l^2*xc5 - 4*sin(q2)*l*xc1^2 + 8*cos(q2)*l*xc1*xc5 - 12*sin(q2)*l*xc5^2 + 4*xc1^2*xc5 + 4*xc5^3)/(2*(3*l^4 + 4*cos(q2)*l^3*xc1 - 4*sin(q2)*l^3*xc5 - 2*cos(2*q2)*l^2*xc1^2 + 4*sin(2*q2)*l^2*xc1*xc5 + 2*cos(2*q2)*l^2*xc5^2 - 4*cos(q2)*l*xc1^3 + 4*sin(q2)*l*xc1^2*xc5 - 4*cos(q2)*l*xc1*xc5^2 + 4*sin(q2)*l*xc5^3 - xc1^4 - 2*xc1^2*xc5^2 - xc5^4)^(1/2)))/(l^2 - 2*l*xc1 + xc1^2 + xc5^2 - 2*l^2*cos(q2) + 2*l*xc1*cos(q2) - 2*l*xc5*sin(q2)) + ((2*xc5 - 2*l*sin(q2))*(2*l^2*sin(q2) + (3*l^4 + 4*cos(q2)*l^3*xc1 - 4*sin(q2)*l^3*xc5 - 2*cos(2*q2)*l^2*xc1^2 + 4*sin(2*q2)*l^2*xc1*xc5 + 2*cos(2*q2)*l^2*xc5^2 - 4*cos(q2)*l*xc1^3 + 4*sin(q2)*l*xc1^2*xc5 - 4*cos(q2)*l*xc1*xc5^2 + 4*sin(q2)*l*xc5^3 - xc1^4 - 2*xc1^2*xc5^2 - xc5^4)^(1/2) - 2*l*xc5))/(l^2 - 2*l*xc1 + xc1^2 + xc5^2 - 2*l^2*cos(q2) + 2*l*xc1*cos(q2) - 2*l*xc5*sin(q2))^2)*((4*l)/(l^2 - 2*l*xc1 + xc1^2 + xc5^2 - 2*l^2*cos(q2) + 2*l*xc1*cos(q2) - 2*l*xc5*sin(q2)) - ((cos(q2) + 1)*(2*l + 2*l*tan(q2/2)^2 - (4*(sin(q2)*l^3 - 2*cos(q2)*sin(q2)*l^2*xc1 + (1 - 2*cos(q2)^2)*l^2*xc5 - sin(q2)*l*xc1^2 + 2*cos(q2)*l*xc1*xc5 - 3*sin(q2)*l*xc5^2 + xc1^2*xc5 + xc5^3))/((cos(q2) + 1)*(-(l^2 + 2*cos(q2)*l*xc1 - 2*sin(q2)*l*xc5 + xc1^2 + xc5^2)*(- 3*l^2 + 2*cos(q2)*l*xc1 - 2*sin(q2)*l*xc5 + xc1^2 + xc5^2))^(1/2))))/(2*(l^2 - 2*l*xc1 + xc1^2 + xc5^2 - 2*l^2*cos(q2) + 2*l*xc1*cos(q2) - 2*l*xc5*sin(q2))) + ((cos(q2) + 1)^2*(2*xc5*tan(q2/2)^2 - 4*l*tan(q2/2) + 2*xc5)*(2*l*xc5 + (2*(-(l^2 + 2*cos(q2)*l*xc1 - 2*sin(q2)*l*xc5 + xc1^2 + xc5^2)*(- 3*l^2 + 2*cos(q2)*l*xc1 - 2*sin(q2)*l*xc5 + xc1^2 + xc5^2))^(1/2))/(cos(q2) + 1) - 4*l^2*tan(q2/2) + 2*l*xc5*tan(q2/2)^2))/(4*(l^2 - 2*l*xc1 + xc1^2 + xc5^2 - 2*l^2*cos(q2) + 2*l*xc1*cos(q2) - 2*l*xc5*sin(q2))^2) - (l*(cos(q2) + 1)^2*(xc5*tan(q2/2)^2 - 2*l*tan(q2/2) + xc5)*(2*xc5*tan(q2/2)^2 - 4*l*tan(q2/2) + 2*xc5))/(l^2 - 2*l*xc1 + xc1^2 + xc5^2 - 2*l^2*cos(q2) + 2*l*xc1*cos(q2) - 2*l*xc5*sin(q2))^2))/(((2*l^2*sin(q2) + (3*l^4 + 4*cos(q2)*l^3*xc1 - 4*sin(q2)*l^3*xc5 - 2*cos(2*q2)*l^2*xc1^2 + 4*sin(2*q2)*l^2*xc1*xc5 + 2*cos(2*q2)*l^2*xc5^2 - 4*cos(q2)*l*xc1^3 + 4*sin(q2)*l*xc1^2*xc5 - 4*cos(q2)*l*xc1*xc5^2 + 4*sin(q2)*l*xc5^3 - xc1^4 - 2*xc1^2*xc5^2 - xc5^4)^(1/2) - 2*l*xc5)^2/(l^2 - 2*l*xc1 + xc1^2 + xc5^2 - 2*l^2*cos(q2) + 2*l*xc1*cos(q2) - 2*l*xc5*sin(q2))^2 + 1)*(((cos(q2) + 1)^2*(2*l*xc5 - (2*(-(l^2 + 2*cos(q2)*l*xc1 - 2*sin(q2)*l*xc5 + xc1^2 + xc5^2)*(- 3*l^2 + 2*cos(q2)*l*xc1 - 2*sin(q2)*l*xc5 + xc1^2 + xc5^2))^(1/2))/(cos(q2) + 1) - 4*l^2*tan(q2/2) + 2*l*xc5*tan(q2/2)^2)^2)/(4*(l^2 - 2*l*xc1 + xc1^2 + xc5^2 - 2*l^2*cos(q2) + 2*l*xc1*cos(q2) - 2*l*xc5*sin(q2))^2) + 1))) + dxc1*((l*cos(2*atan((2*l^2*sin(q2) + (3*l^4 + 4*cos(q2)*l^3*xc1 - 4*sin(q2)*l^3*xc5 - 2*cos(2*q2)*l^2*xc1^2 + 4*sin(2*q2)*l^2*xc1*xc5 + 2*cos(2*q2)*l^2*xc5^2 - 4*cos(q2)*l*xc1^3 + 4*sin(q2)*l*xc1^2*xc5 - 4*cos(q2)*l*xc1*xc5^2 + 4*sin(q2)*l*xc5^3 - xc1^4 - 2*xc1^2*xc5^2 - xc5^4)^(1/2) - 2*l*xc5)/(l^2 - 2*l*xc1 + xc1^2 + xc5^2 - 2*l^2*cos(q2) + 2*l*xc1*cos(q2) - 2*l*xc5*sin(q2))))*(((cos(q2) + 1)^2*(2*xc1 - 2*l + 2*l*cos(q2))*(2*l*xc5 - (2*(-(l^2 + 2*cos(q2)*l*xc1 - 2*sin(q2)*l*xc5 + xc1^2 + xc5^2)*(- 3*l^2 + 2*cos(q2)*l*xc1 - 2*sin(q2)*l*xc5 + xc1^2 + xc5^2))^(1/2))/(cos(q2) + 1) - 4*l^2*tan(q2/2) + 2*l*xc5*tan(q2/2)^2)^2)/(2*(l^2 - 2*l*xc1 + xc1^2 + xc5^2 - 2*l^2*cos(q2) + 2*l*xc1*cos(q2) - 2*l*xc5*sin(q2))^3) - ((cos(q2) + 1)*((2*xc1 + 2*l*cos(q2))*(l^2 + 2*cos(q2)*l*xc1 - 2*sin(q2)*l*xc5 + xc1^2 + xc5^2) + (2*xc1 + 2*l*cos(q2))*(- 3*l^2 + 2*cos(q2)*l*xc1 - 2*sin(q2)*l*xc5 + xc1^2 + xc5^2))*(2*l*xc5 - (2*(-(l^2 + 2*cos(q2)*l*xc1 - 2*sin(q2)*l*xc5 + xc1^2 + xc5^2)*(- 3*l^2 + 2*cos(q2)*l*xc1 - 2*sin(q2)*l*xc5 + xc1^2 + xc5^2))^(1/2))/(cos(q2) + 1) - 4*l^2*tan(q2/2) + 2*l*xc5*tan(q2/2)^2))/(2*(-(l^2 + 2*cos(q2)*l*xc1 - 2*sin(q2)*l*xc5 + xc1^2 + xc5^2)*(- 3*l^2 + 2*cos(q2)*l*xc1 - 2*sin(q2)*l*xc5 + xc1^2 + xc5^2))^(1/2)*(l^2 - 2*l*xc1 + xc1^2 + xc5^2 - 2*l^2*cos(q2) + 2*l*xc1*cos(q2) - 2*l*xc5*sin(q2))^2))*((4*l)/(l^2 - 2*l*xc1 + xc1^2 + xc5^2 - 2*l^2*cos(q2) + 2*l*xc1*cos(q2) - 2*l*xc5*sin(q2)) - ((cos(q2) + 1)*(2*l + 2*l*tan(q2/2)^2 - (4*(sin(q2)*l^3 - 2*cos(q2)*sin(q2)*l^2*xc1 + (1 - 2*cos(q2)^2)*l^2*xc5 - sin(q2)*l*xc1^2 + 2*cos(q2)*l*xc1*xc5 - 3*sin(q2)*l*xc5^2 + xc1^2*xc5 + xc5^3))/((cos(q2) + 1)*(-(l^2 + 2*cos(q2)*l*xc1 - 2*sin(q2)*l*xc5 + xc1^2 + xc5^2)*(- 3*l^2 + 2*cos(q2)*l*xc1 - 2*sin(q2)*l*xc5 + xc1^2 + xc5^2))^(1/2))))/(2*(l^2 - 2*l*xc1 + xc1^2 + xc5^2 - 2*l^2*cos(q2) + 2*l*xc1*cos(q2) - 2*l*xc5*sin(q2))) + ((cos(q2) + 1)^2*(2*xc5*tan(q2/2)^2 - 4*l*tan(q2/2) + 2*xc5)*(2*l*xc5 + (2*(-(l^2 + 2*cos(q2)*l*xc1 - 2*sin(q2)*l*xc5 + xc1^2 + xc5^2)*(- 3*l^2 + 2*cos(q2)*l*xc1 - 2*sin(q2)*l*xc5 + xc1^2 + xc5^2))^(1/2))/(cos(q2) + 1) - 4*l^2*tan(q2/2) + 2*l*xc5*tan(q2/2)^2))/(4*(l^2 - 2*l*xc1 + xc1^2 + xc5^2 - 2*l^2*cos(q2) + 2*l*xc1*cos(q2) - 2*l*xc5*sin(q2))^2) - (l*(cos(q2) + 1)^2*(xc5*tan(q2/2)^2 - 2*l*tan(q2/2) + xc5)*(2*xc5*tan(q2/2)^2 - 4*l*tan(q2/2) + 2*xc5))/(l^2 - 2*l*xc1 + xc1^2 + xc5^2 - 2*l^2*cos(q2) + 2*l*xc1*cos(q2) - 2*l*xc5*sin(q2))^2))/(((cos(q2) + 1)^2*(2*l*xc5 - (2*(-(l^2 + 2*cos(q2)*l*xc1 - 2*sin(q2)*l*xc5 + xc1^2 + xc5^2)*(- 3*l^2 + 2*cos(q2)*l*xc1 - 2*sin(q2)*l*xc5 + xc1^2 + xc5^2))^(1/2))/(cos(q2) + 1) - 4*l^2*tan(q2/2) + 2*l*xc5*tan(q2/2)^2)^2)/(4*(l^2 - 2*l*xc1 + xc1^2 + xc5^2 - 2*l^2*cos(q2) + 2*l*xc1*cos(q2) - 2*l*xc5*sin(q2))^2) + 1)^2 - (l*cos(2*atan((2*l^2*sin(q2) + (3*l^4 + 4*cos(q2)*l^3*xc1 - 4*sin(q2)*l^3*xc5 - 2*cos(2*q2)*l^2*xc1^2 + 4*sin(2*q2)*l^2*xc1*xc5 + 2*cos(2*q2)*l^2*xc5^2 - 4*cos(q2)*l*xc1^3 + 4*sin(q2)*l*xc1^2*xc5 - 4*cos(q2)*l*xc1*xc5^2 + 4*sin(q2)*l*xc5^3 - xc1^4 - 2*xc1^2*xc5^2 - xc5^4)^(1/2) - 2*l*xc5)/(l^2 - 2*l*xc1 + xc1^2 + xc5^2 - 2*l^2*cos(q2) + 2*l*xc1*cos(q2) - 2*l*xc5*sin(q2))))*((4*l*(2*xc1 - 2*l + 2*l*cos(q2)))/(l^2 - 2*l*xc1 + xc1^2 + xc5^2 - 2*l^2*cos(q2) + 2*l*xc1*cos(q2) - 2*l*xc5*sin(q2))^2 - ((cos(q2) + 1)*((4*(2*xc1*xc5 + 2*l*xc5*cos(q2) - 2*l*xc1*sin(q2) - 2*l^2*cos(q2)*sin(q2)))/((cos(q2) + 1)*(-(l^2 + 2*cos(q2)*l*xc1 - 2*sin(q2)*l*xc5 + xc1^2 + xc5^2)*(- 3*l^2 + 2*cos(q2)*l*xc1 - 2*sin(q2)*l*xc5 + xc1^2 + xc5^2))^(1/2)) + (2*((2*xc1 + 2*l*cos(q2))*(l^2 + 2*cos(q2)*l*xc1 - 2*sin(q2)*l*xc5 + xc1^2 + xc5^2) + (2*xc1 + 2*l*cos(q2))*(- 3*l^2 + 2*cos(q2)*l*xc1 - 2*sin(q2)*l*xc5 + xc1^2 + xc5^2))*(sin(q2)*l^3 - 2*cos(q2)*sin(q2)*l^2*xc1 + (1 - 2*cos(q2)^2)*l^2*xc5 - sin(q2)*l*xc1^2 + 2*cos(q2)*l*xc1*xc5 - 3*sin(q2)*l*xc5^2 + xc1^2*xc5 + xc5^3))/((cos(q2) + 1)*(-(l^2 + 2*cos(q2)*l*xc1 - 2*sin(q2)*l*xc5 + xc1^2 + xc5^2)*(- 3*l^2 + 2*cos(q2)*l*xc1 - 2*sin(q2)*l*xc5 + xc1^2 + xc5^2))^(3/2))))/(2*(l^2 - 2*l*xc1 + xc1^2 + xc5^2 - 2*l^2*cos(q2) + 2*l*xc1*cos(q2) - 2*l*xc5*sin(q2))) - ((cos(q2) + 1)*(2*l + 2*l*tan(q2/2)^2 - (4*(sin(q2)*l^3 - 2*cos(q2)*sin(q2)*l^2*xc1 + (1 - 2*cos(q2)^2)*l^2*xc5 - sin(q2)*l*xc1^2 + 2*cos(q2)*l*xc1*xc5 - 3*sin(q2)*l*xc5^2 + xc1^2*xc5 + xc5^3))/((cos(q2) + 1)*(-(l^2 + 2*cos(q2)*l*xc1 - 2*sin(q2)*l*xc5 + xc1^2 + xc5^2)*(- 3*l^2 + 2*cos(q2)*l*xc1 - 2*sin(q2)*l*xc5 + xc1^2 + xc5^2))^(1/2)))*(2*xc1 - 2*l + 2*l*cos(q2)))/(2*(l^2 - 2*l*xc1 + xc1^2 + xc5^2 - 2*l^2*cos(q2) + 2*l*xc1*cos(q2) - 2*l*xc5*sin(q2))^2) + ((cos(q2) + 1)^2*(2*xc1 - 2*l + 2*l*cos(q2))*(2*xc5*tan(q2/2)^2 - 4*l*tan(q2/2) + 2*xc5)*(2*l*xc5 + (2*(-(l^2 + 2*cos(q2)*l*xc1 - 2*sin(q2)*l*xc5 + xc1^2 + xc5^2)*(- 3*l^2 + 2*cos(q2)*l*xc1 - 2*sin(q2)*l*xc5 + xc1^2 + xc5^2))^(1/2))/(cos(q2) + 1) - 4*l^2*tan(q2/2) + 2*l*xc5*tan(q2/2)^2))/(2*(l^2 - 2*l*xc1 + xc1^2 + xc5^2 - 2*l^2*cos(q2) + 2*l*xc1*cos(q2) - 2*l*xc5*sin(q2))^3) + ((cos(q2) + 1)*((2*xc1 + 2*l*cos(q2))*(l^2 + 2*cos(q2)*l*xc1 - 2*sin(q2)*l*xc5 + xc1^2 + xc5^2) + (2*xc1 + 2*l*cos(q2))*(- 3*l^2 + 2*cos(q2)*l*xc1 - 2*sin(q2)*l*xc5 + xc1^2 + xc5^2))*(2*xc5*tan(q2/2)^2 - 4*l*tan(q2/2) + 2*xc5))/(4*(-(l^2 + 2*cos(q2)*l*xc1 - 2*sin(q2)*l*xc5 + xc1^2 + xc5^2)*(- 3*l^2 + 2*cos(q2)*l*xc1 - 2*sin(q2)*l*xc5 + xc1^2 + xc5^2))^(1/2)*(l^2 - 2*l*xc1 + xc1^2 + xc5^2 - 2*l^2*cos(q2) + 2*l*xc1*cos(q2) - 2*l*xc5*sin(q2))^2) - (2*l*(cos(q2) + 1)^2*(xc5*tan(q2/2)^2 - 2*l*tan(q2/2) + xc5)*(2*xc1 - 2*l + 2*l*cos(q2))*(2*xc5*tan(q2/2)^2 - 4*l*tan(q2/2) + 2*xc5))/(l^2 - 2*l*xc1 + xc1^2 + xc5^2 - 2*l^2*cos(q2) + 2*l*xc1*cos(q2) - 2*l*xc5*sin(q2))^3))/(((cos(q2) + 1)^2*(2*l*xc5 - (2*(-(l^2 + 2*cos(q2)*l*xc1 - 2*sin(q2)*l*xc5 + xc1^2 + xc5^2)*(- 3*l^2 + 2*cos(q2)*l*xc1 - 2*sin(q2)*l*xc5 + xc1^2 + xc5^2))^(1/2))/(cos(q2) + 1) - 4*l^2*tan(q2/2) + 2*l*xc5*tan(q2/2)^2)^2)/(4*(l^2 - 2*l*xc1 + xc1^2 + xc5^2 - 2*l^2*cos(q2) + 2*l*xc1*cos(q2) - 2*l*xc5*sin(q2))^2) + 1) + (2*l*sin(2*atan((2*l^2*sin(q2) + (3*l^4 + 4*cos(q2)*l^3*xc1 - 4*sin(q2)*l^3*xc5 - 2*cos(2*q2)*l^2*xc1^2 + 4*sin(2*q2)*l^2*xc1*xc5 + 2*cos(2*q2)*l^2*xc5^2 - 4*cos(q2)*l*xc1^3 + 4*sin(q2)*l*xc1^2*xc5 - 4*cos(q2)*l*xc1*xc5^2 + 4*sin(q2)*l*xc5^3 - xc1^4 - 2*xc1^2*xc5^2 - xc5^4)^(1/2) - 2*l*xc5)/(l^2 - 2*l*xc1 + xc1^2 + xc5^2 - 2*l^2*cos(q2) + 2*l*xc1*cos(q2) - 2*l*xc5*sin(q2))))*(((2*xc1 - 2*l + 2*l*cos(q2))*(2*l^2*sin(q2) + (3*l^4 + 4*cos(q2)*l^3*xc1 - 4*sin(q2)*l^3*xc5 - 2*cos(2*q2)*l^2*xc1^2 + 4*sin(2*q2)*l^2*xc1*xc5 + 2*cos(2*q2)*l^2*xc5^2 - 4*cos(q2)*l*xc1^3 + 4*sin(q2)*l*xc1^2*xc5 - 4*cos(q2)*l*xc1*xc5^2 + 4*sin(q2)*l*xc5^3 - xc1^4 - 2*xc1^2*xc5^2 - xc5^4)^(1/2) - 2*l*xc5))/(l^2 - 2*l*xc1 + xc1^2 + xc5^2 - 2*l^2*cos(q2) + 2*l*xc1*cos(q2) - 2*l*xc5*sin(q2))^2 + (- 4*cos(q2)*l^3 + 4*cos(2*q2)*l^2*xc1 - 4*sin(2*q2)*l^2*xc5 + 12*cos(q2)*l*xc1^2 - 8*sin(q2)*l*xc1*xc5 + 4*cos(q2)*l*xc5^2 + 4*xc1^3 + 4*xc1*xc5^2)/(2*(l^2 - 2*l*xc1 + xc1^2 + xc5^2 - 2*l^2*cos(q2) + 2*l*xc1*cos(q2) - 2*l*xc5*sin(q2))*(3*l^4 + 4*cos(q2)*l^3*xc1 - 4*sin(q2)*l^3*xc5 - 2*cos(2*q2)*l^2*xc1^2 + 4*sin(2*q2)*l^2*xc1*xc5 + 2*cos(2*q2)*l^2*xc5^2 - 4*cos(q2)*l*xc1^3 + 4*sin(q2)*l*xc1^2*xc5 - 4*cos(q2)*l*xc1*xc5^2 + 4*sin(q2)*l*xc5^3 - xc1^4 - 2*xc1^2*xc5^2 - xc5^4)^(1/2)))*((4*l)/(l^2 - 2*l*xc1 + xc1^2 + xc5^2 - 2*l^2*cos(q2) + 2*l*xc1*cos(q2) - 2*l*xc5*sin(q2)) - ((cos(q2) + 1)*(2*l + 2*l*tan(q2/2)^2 - (4*(sin(q2)*l^3 - 2*cos(q2)*sin(q2)*l^2*xc1 + (1 - 2*cos(q2)^2)*l^2*xc5 - sin(q2)*l*xc1^2 + 2*cos(q2)*l*xc1*xc5 - 3*sin(q2)*l*xc5^2 + xc1^2*xc5 + xc5^3))/((cos(q2) + 1)*(-(l^2 + 2*cos(q2)*l*xc1 - 2*sin(q2)*l*xc5 + xc1^2 + xc5^2)*(- 3*l^2 + 2*cos(q2)*l*xc1 - 2*sin(q2)*l*xc5 + xc1^2 + xc5^2))^(1/2))))/(2*(l^2 - 2*l*xc1 + xc1^2 + xc5^2 - 2*l^2*cos(q2) + 2*l*xc1*cos(q2) - 2*l*xc5*sin(q2))) + ((cos(q2) + 1)^2*(2*xc5*tan(q2/2)^2 - 4*l*tan(q2/2) + 2*xc5)*(2*l*xc5 + (2*(-(l^2 + 2*cos(q2)*l*xc1 - 2*sin(q2)*l*xc5 + xc1^2 + xc5^2)*(- 3*l^2 + 2*cos(q2)*l*xc1 - 2*sin(q2)*l*xc5 + xc1^2 + xc5^2))^(1/2))/(cos(q2) + 1) - 4*l^2*tan(q2/2) + 2*l*xc5*tan(q2/2)^2))/(4*(l^2 - 2*l*xc1 + xc1^2 + xc5^2 - 2*l^2*cos(q2) + 2*l*xc1*cos(q2) - 2*l*xc5*sin(q2))^2) - (l*(cos(q2) + 1)^2*(xc5*tan(q2/2)^2 - 2*l*tan(q2/2) + xc5)*(2*xc5*tan(q2/2)^2 - 4*l*tan(q2/2) + 2*xc5))/(l^2 - 2*l*xc1 + xc1^2 + xc5^2 - 2*l^2*cos(q2) + 2*l*xc1*cos(q2) - 2*l*xc5*sin(q2))^2))/(((2*l^2*sin(q2) + (3*l^4 + 4*cos(q2)*l^3*xc1 - 4*sin(q2)*l^3*xc5 - 2*cos(2*q2)*l^2*xc1^2 + 4*sin(2*q2)*l^2*xc1*xc5 + 2*cos(2*q2)*l^2*xc5^2 - 4*cos(q2)*l*xc1^3 + 4*sin(q2)*l*xc1^2*xc5 - 4*cos(q2)*l*xc1*xc5^2 + 4*sin(q2)*l*xc5^3 - xc1^4 - 2*xc1^2*xc5^2 - xc5^4)^(1/2) - 2*l*xc5)^2/(l^2 - 2*l*xc1 + xc1^2 + xc5^2 - 2*l^2*cos(q2) + 2*l*xc1*cos(q2) - 2*l*xc5*sin(q2))^2 + 1)*(((cos(q2) + 1)^2*(2*l*xc5 - (2*(-(l^2 + 2*cos(q2)*l*xc1 - 2*sin(q2)*l*xc5 + xc1^2 + xc5^2)*(- 3*l^2 + 2*cos(q2)*l*xc1 - 2*sin(q2)*l*xc5 + xc1^2 + xc5^2))^(1/2))/(cos(q2) + 1) - 4*l^2*tan(q2/2) + 2*l*xc5*tan(q2/2)^2)^2)/(4*(l^2 - 2*l*xc1 + xc1^2 + xc5^2 - 2*l^2*cos(q2) + 2*l*xc1*cos(q2) - 2*l*xc5*sin(q2))^2) + 1))) + dq2*((l*cos(2*atan((2*l^2*sin(q2) + (3*l^4 + 4*cos(q2)*l^3*xc1 - 4*sin(q2)*l^3*xc5 - 2*cos(2*q2)*l^2*xc1^2 + 4*sin(2*q2)*l^2*xc1*xc5 + 2*cos(2*q2)*l^2*xc5^2 - 4*cos(q2)*l*xc1^3 + 4*sin(q2)*l*xc1^2*xc5 - 4*cos(q2)*l*xc1*xc5^2 + 4*sin(q2)*l*xc5^3 - xc1^4 - 2*xc1^2*xc5^2 - xc5^4)^(1/2) - 2*l*xc5)/(l^2 - 2*l*xc1 + xc1^2 + xc5^2 - 2*l^2*cos(q2) + 2*l*xc1*cos(q2) - 2*l*xc5*sin(q2))))*((4*l*(2*l*xc5*cos(q2) - 2*l^2*sin(q2) + 2*l*xc1*sin(q2)))/(l^2 - 2*l*xc1 + xc1^2 + xc5^2 - 2*l^2*cos(q2) + 2*l*xc1*cos(q2) - 2*l*xc5*sin(q2))^2 + (sin(q2)*(2*l + 2*l*tan(q2/2)^2 - (4*(sin(q2)*l^3 - 2*cos(q2)*sin(q2)*l^2*xc1 + (1 - 2*cos(q2)^2)*l^2*xc5 - sin(q2)*l*xc1^2 + 2*cos(q2)*l*xc1*xc5 - 3*sin(q2)*l*xc5^2 + xc1^2*xc5 + xc5^3))/((cos(q2) + 1)*(-(l^2 + 2*cos(q2)*l*xc1 - 2*sin(q2)*l*xc5 + xc1^2 + xc5^2)*(- 3*l^2 + 2*cos(q2)*l*xc1 - 2*sin(q2)*l*xc5 + xc1^2 + xc5^2))^(1/2))))/(2*(l^2 - 2*l*xc1 + xc1^2 + xc5^2 - 2*l^2*cos(q2) + 2*l*xc1*cos(q2) - 2*l*xc5*sin(q2))) - ((cos(q2) + 1)*((4*(- l^3*cos(q2) + 2*l^2*xc1*cos(q2)^2 - 2*l^2*xc1*sin(q2)^2 - 4*l^2*xc5*cos(q2)*sin(q2) + l*xc1^2*cos(q2) + 2*l*xc1*xc5*sin(q2) + 3*l*xc5^2*cos(q2)))/((cos(q2) + 1)*(-(l^2 + 2*cos(q2)*l*xc1 - 2*sin(q2)*l*xc5 + xc1^2 + xc5^2)*(- 3*l^2 + 2*cos(q2)*l*xc1 - 2*sin(q2)*l*xc5 + xc1^2 + xc5^2))^(1/2)) + 4*l*tan(q2/2)*(tan(q2/2)^2/2 + 1/2) - (4*sin(q2)*(sin(q2)*l^3 - 2*cos(q2)*sin(q2)*l^2*xc1 + (1 - 2*cos(q2)^2)*l^2*xc5 - sin(q2)*l*xc1^2 + 2*cos(q2)*l*xc1*xc5 - 3*sin(q2)*l*xc5^2 + xc1^2*xc5 + xc5^3))/((cos(q2) + 1)^2*(-(l^2 + 2*cos(q2)*l*xc1 - 2*sin(q2)*l*xc5 + xc1^2 + xc5^2)*(- 3*l^2 + 2*cos(q2)*l*xc1 - 2*sin(q2)*l*xc5 + xc1^2 + xc5^2))^(1/2)) + (2*((2*l*xc5*cos(q2) + 2*l*xc1*sin(q2))*(l^2 + 2*cos(q2)*l*xc1 - 2*sin(q2)*l*xc5 + xc1^2 + xc5^2) + (2*l*xc5*cos(q2) + 2*l*xc1*sin(q2))*(- 3*l^2 + 2*cos(q2)*l*xc1 - 2*sin(q2)*l*xc5 + xc1^2 + xc5^2))*(sin(q2)*l^3 - 2*cos(q2)*sin(q2)*l^2*xc1 + (1 - 2*cos(q2)^2)*l^2*xc5 - sin(q2)*l*xc1^2 + 2*cos(q2)*l*xc1*xc5 - 3*sin(q2)*l*xc5^2 + xc1^2*xc5 + xc5^3))/((cos(q2) + 1)*(-(l^2 + 2*cos(q2)*l*xc1 - 2*sin(q2)*l*xc5 + xc1^2 + xc5^2)*(- 3*l^2 + 2*cos(q2)*l*xc1 - 2*sin(q2)*l*xc5 + xc1^2 + xc5^2))^(3/2))))/(2*(l^2 - 2*l*xc1 + xc1^2 + xc5^2 - 2*l^2*cos(q2) + 2*l*xc1*cos(q2) - 2*l*xc5*sin(q2))) - ((4*l*(tan(q2/2)^2/2 + 1/2) - 4*xc5*tan(q2/2)*(tan(q2/2)^2/2 + 1/2))*(cos(q2) + 1)^2*(2*l*xc5 + (2*(-(l^2 + 2*cos(q2)*l*xc1 - 2*sin(q2)*l*xc5 + xc1^2 + xc5^2)*(- 3*l^2 + 2*cos(q2)*l*xc1 - 2*sin(q2)*l*xc5 + xc1^2 + xc5^2))^(1/2))/(cos(q2) + 1) - 4*l^2*tan(q2/2) + 2*l*xc5*tan(q2/2)^2))/(4*(l^2 - 2*l*xc1 + xc1^2 + xc5^2 - 2*l^2*cos(q2) + 2*l*xc1*cos(q2) - 2*l*xc5*sin(q2))^2) - ((cos(q2) + 1)*(2*l + 2*l*tan(q2/2)^2 - (4*(sin(q2)*l^3 - 2*cos(q2)*sin(q2)*l^2*xc1 + (1 - 2*cos(q2)^2)*l^2*xc5 - sin(q2)*l*xc1^2 + 2*cos(q2)*l*xc1*xc5 - 3*sin(q2)*l*xc5^2 + xc1^2*xc5 + xc5^3))/((cos(q2) + 1)*(-(l^2 + 2*cos(q2)*l*xc1 - 2*sin(q2)*l*xc5 + xc1^2 + xc5^2)*(- 3*l^2 + 2*cos(q2)*l*xc1 - 2*sin(q2)*l*xc5 + xc1^2 + xc5^2))^(1/2)))*(2*l*xc5*cos(q2) - 2*l^2*sin(q2) + 2*l*xc1*sin(q2)))/(2*(l^2 - 2*l*xc1 + xc1^2 + xc5^2 - 2*l^2*cos(q2) + 2*l*xc1*cos(q2) - 2*l*xc5*sin(q2))^2) + ((cos(q2) + 1)^2*(2*xc5*tan(q2/2)^2 - 4*l*tan(q2/2) + 2*xc5)*((2*sin(q2)*(-(l^2 + 2*cos(q2)*l*xc1 - 2*sin(q2)*l*xc5 + xc1^2 + xc5^2)*(- 3*l^2 + 2*cos(q2)*l*xc1 - 2*sin(q2)*l*xc5 + xc1^2 + xc5^2))^(1/2))/(cos(q2) + 1)^2 - 4*l^2*(tan(q2/2)^2/2 + 1/2) + ((2*l*xc5*cos(q2) + 2*l*xc1*sin(q2))*(l^2 + 2*cos(q2)*l*xc1 - 2*sin(q2)*l*xc5 + xc1^2 + xc5^2) + (2*l*xc5*cos(q2) + 2*l*xc1*sin(q2))*(- 3*l^2 + 2*cos(q2)*l*xc1 - 2*sin(q2)*l*xc5 + xc1^2 + xc5^2))/((cos(q2) + 1)*(-(l^2 + 2*cos(q2)*l*xc1 - 2*sin(q2)*l*xc5 + xc1^2 + xc5^2)*(- 3*l^2 + 2*cos(q2)*l*xc1 - 2*sin(q2)*l*xc5 + xc1^2 + xc5^2))^(1/2)) + 4*l*xc5*tan(q2/2)*(tan(q2/2)^2/2 + 1/2)))/(4*(l^2 - 2*l*xc1 + xc1^2 + xc5^2 - 2*l^2*cos(q2) + 2*l*xc1*cos(q2) - 2*l*xc5*sin(q2))^2) - (sin(q2)*(cos(q2) + 1)*(2*xc5*tan(q2/2)^2 - 4*l*tan(q2/2) + 2*xc5)*(2*l*xc5 + (2*(-(l^2 + 2*cos(q2)*l*xc1 - 2*sin(q2)*l*xc5 + xc1^2 + xc5^2)*(- 3*l^2 + 2*cos(q2)*l*xc1 - 2*sin(q2)*l*xc5 + xc1^2 + xc5^2))^(1/2))/(cos(q2) + 1) - 4*l^2*tan(q2/2) + 2*l*xc5*tan(q2/2)^2))/(2*(l^2 - 2*l*xc1 + xc1^2 + xc5^2 - 2*l^2*cos(q2) + 2*l*xc1*cos(q2) - 2*l*xc5*sin(q2))^2) + ((cos(q2) + 1)^2*(2*l*xc5*cos(q2) - 2*l^2*sin(q2) + 2*l*xc1*sin(q2))*(2*xc5*tan(q2/2)^2 - 4*l*tan(q2/2) + 2*xc5)*(2*l*xc5 + (2*(-(l^2 + 2*cos(q2)*l*xc1 - 2*sin(q2)*l*xc5 + xc1^2 + xc5^2)*(- 3*l^2 + 2*cos(q2)*l*xc1 - 2*sin(q2)*l*xc5 + xc1^2 + xc5^2))^(1/2))/(cos(q2) + 1) - 4*l^2*tan(q2/2) + 2*l*xc5*tan(q2/2)^2))/(2*(l^2 - 2*l*xc1 + xc1^2 + xc5^2 - 2*l^2*cos(q2) + 2*l*xc1*cos(q2) - 2*l*xc5*sin(q2))^3) + (l*(4*l*(tan(q2/2)^2/2 + 1/2) - 4*xc5*tan(q2/2)*(tan(q2/2)^2/2 + 1/2))*(cos(q2) + 1)^2*(xc5*tan(q2/2)^2 - 2*l*tan(q2/2) + xc5))/(l^2 - 2*l*xc1 + xc1^2 + xc5^2 - 2*l^2*cos(q2) + 2*l*xc1*cos(q2) - 2*l*xc5*sin(q2))^2 + (l*(2*l*(tan(q2/2)^2/2 + 1/2) - 2*xc5*tan(q2/2)*(tan(q2/2)^2/2 + 1/2))*(cos(q2) + 1)^2*(2*xc5*tan(q2/2)^2 - 4*l*tan(q2/2) + 2*xc5))/(l^2 - 2*l*xc1 + xc1^2 + xc5^2 - 2*l^2*cos(q2) + 2*l*xc1*cos(q2) - 2*l*xc5*sin(q2))^2 + (2*l*sin(q2)*(cos(q2) + 1)*(xc5*tan(q2/2)^2 - 2*l*tan(q2/2) + xc5)*(2*xc5*tan(q2/2)^2 - 4*l*tan(q2/2) + 2*xc5))/(l^2 - 2*l*xc1 + xc1^2 + xc5^2 - 2*l^2*cos(q2) + 2*l*xc1*cos(q2) - 2*l*xc5*sin(q2))^2 - (2*l*(cos(q2) + 1)^2*(xc5*tan(q2/2)^2 - 2*l*tan(q2/2) + xc5)*(2*l*xc5*cos(q2) - 2*l^2*sin(q2) + 2*l*xc1*sin(q2))*(2*xc5*tan(q2/2)^2 - 4*l*tan(q2/2) + 2*xc5))/(l^2 - 2*l*xc1 + xc1^2 + xc5^2 - 2*l^2*cos(q2) + 2*l*xc1*cos(q2) - 2*l*xc5*sin(q2))^3))/(((cos(q2) + 1)^2*(2*l*xc5 - (2*(-(l^2 + 2*cos(q2)*l*xc1 - 2*sin(q2)*l*xc5 + xc1^2 + xc5^2)*(- 3*l^2 + 2*cos(q2)*l*xc1 - 2*sin(q2)*l*xc5 + xc1^2 + xc5^2))^(1/2))/(cos(q2) + 1) - 4*l^2*tan(q2/2) + 2*l*xc5*tan(q2/2)^2)^2)/(4*(l^2 - 2*l*xc1 + xc1^2 + xc5^2 - 2*l^2*cos(q2) + 2*l*xc1*cos(q2) - 2*l*xc5*sin(q2))^2) + 1) + (l*cos(2*atan((2*l^2*sin(q2) + (3*l^4 + 4*cos(q2)*l^3*xc1 - 4*sin(q2)*l^3*xc5 - 2*cos(2*q2)*l^2*xc1^2 + 4*sin(2*q2)*l^2*xc1*xc5 + 2*cos(2*q2)*l^2*xc5^2 - 4*cos(q2)*l*xc1^3 + 4*sin(q2)*l*xc1^2*xc5 - 4*cos(q2)*l*xc1*xc5^2 + 4*sin(q2)*l*xc5^3 - xc1^4 - 2*xc1^2*xc5^2 - xc5^4)^(1/2) - 2*l*xc5)/(l^2 - 2*l*xc1 + xc1^2 + xc5^2 - 2*l^2*cos(q2) + 2*l*xc1*cos(q2) - 2*l*xc5*sin(q2))))*(((cos(q2) + 1)^2*(4*l^2*(tan(q2/2)^2/2 + 1/2) + (2*sin(q2)*(-(l^2 + 2*cos(q2)*l*xc1 - 2*sin(q2)*l*xc5 + xc1^2 + xc5^2)*(- 3*l^2 + 2*cos(q2)*l*xc1 - 2*sin(q2)*l*xc5 + xc1^2 + xc5^2))^(1/2))/(cos(q2) + 1)^2 + ((2*l*xc5*cos(q2) + 2*l*xc1*sin(q2))*(l^2 + 2*cos(q2)*l*xc1 - 2*sin(q2)*l*xc5 + xc1^2 + xc5^2) + (2*l*xc5*cos(q2) + 2*l*xc1*sin(q2))*(- 3*l^2 + 2*cos(q2)*l*xc1 - 2*sin(q2)*l*xc5 + xc1^2 + xc5^2))/((cos(q2) + 1)*(-(l^2 + 2*cos(q2)*l*xc1 - 2*sin(q2)*l*xc5 + xc1^2 + xc5^2)*(- 3*l^2 + 2*cos(q2)*l*xc1 - 2*sin(q2)*l*xc5 + xc1^2 + xc5^2))^(1/2)) - 4*l*xc5*tan(q2/2)*(tan(q2/2)^2/2 + 1/2))*(2*l*xc5 - (2*(-(l^2 + 2*cos(q2)*l*xc1 - 2*sin(q2)*l*xc5 + xc1^2 + xc5^2)*(- 3*l^2 + 2*cos(q2)*l*xc1 - 2*sin(q2)*l*xc5 + xc1^2 + xc5^2))^(1/2))/(cos(q2) + 1) - 4*l^2*tan(q2/2) + 2*l*xc5*tan(q2/2)^2))/(2*(l^2 - 2*l*xc1 + xc1^2 + xc5^2 - 2*l^2*cos(q2) + 2*l*xc1*cos(q2) - 2*l*xc5*sin(q2))^2) - ((cos(q2) + 1)^2*(2*l*xc5*cos(q2) - 2*l^2*sin(q2) + 2*l*xc1*sin(q2))*(2*l*xc5 - (2*(-(l^2 + 2*cos(q2)*l*xc1 - 2*sin(q2)*l*xc5 + xc1^2 + xc5^2)*(- 3*l^2 + 2*cos(q2)*l*xc1 - 2*sin(q2)*l*xc5 + xc1^2 + xc5^2))^(1/2))/(cos(q2) + 1) - 4*l^2*tan(q2/2) + 2*l*xc5*tan(q2/2)^2)^2)/(2*(l^2 - 2*l*xc1 + xc1^2 + xc5^2 - 2*l^2*cos(q2) + 2*l*xc1*cos(q2) - 2*l*xc5*sin(q2))^3) + (sin(q2)*(cos(q2) + 1)*(2*l*xc5 - (2*(-(l^2 + 2*cos(q2)*l*xc1 - 2*sin(q2)*l*xc5 + xc1^2 + xc5^2)*(- 3*l^2 + 2*cos(q2)*l*xc1 - 2*sin(q2)*l*xc5 + xc1^2 + xc5^2))^(1/2))/(cos(q2) + 1) - 4*l^2*tan(q2/2) + 2*l*xc5*tan(q2/2)^2)^2)/(2*(l^2 - 2*l*xc1 + xc1^2 + xc5^2 - 2*l^2*cos(q2) + 2*l*xc1*cos(q2) - 2*l*xc5*sin(q2))^2))*((4*l)/(l^2 - 2*l*xc1 + xc1^2 + xc5^2 - 2*l^2*cos(q2) + 2*l*xc1*cos(q2) - 2*l*xc5*sin(q2)) - ((cos(q2) + 1)*(2*l + 2*l*tan(q2/2)^2 - (4*(sin(q2)*l^3 - 2*cos(q2)*sin(q2)*l^2*xc1 + (1 - 2*cos(q2)^2)*l^2*xc5 - sin(q2)*l*xc1^2 + 2*cos(q2)*l*xc1*xc5 - 3*sin(q2)*l*xc5^2 + xc1^2*xc5 + xc5^3))/((cos(q2) + 1)*(-(l^2 + 2*cos(q2)*l*xc1 - 2*sin(q2)*l*xc5 + xc1^2 + xc5^2)*(- 3*l^2 + 2*cos(q2)*l*xc1 - 2*sin(q2)*l*xc5 + xc1^2 + xc5^2))^(1/2))))/(2*(l^2 - 2*l*xc1 + xc1^2 + xc5^2 - 2*l^2*cos(q2) + 2*l*xc1*cos(q2) - 2*l*xc5*sin(q2))) + ((cos(q2) + 1)^2*(2*xc5*tan(q2/2)^2 - 4*l*tan(q2/2) + 2*xc5)*(2*l*xc5 + (2*(-(l^2 + 2*cos(q2)*l*xc1 - 2*sin(q2)*l*xc5 + xc1^2 + xc5^2)*(- 3*l^2 + 2*cos(q2)*l*xc1 - 2*sin(q2)*l*xc5 + xc1^2 + xc5^2))^(1/2))/(cos(q2) + 1) - 4*l^2*tan(q2/2) + 2*l*xc5*tan(q2/2)^2))/(4*(l^2 - 2*l*xc1 + xc1^2 + xc5^2 - 2*l^2*cos(q2) + 2*l*xc1*cos(q2) - 2*l*xc5*sin(q2))^2) - (l*(cos(q2) + 1)^2*(xc5*tan(q2/2)^2 - 2*l*tan(q2/2) + xc5)*(2*xc5*tan(q2/2)^2 - 4*l*tan(q2/2) + 2*xc5))/(l^2 - 2*l*xc1 + xc1^2 + xc5^2 - 2*l^2*cos(q2) + 2*l*xc1*cos(q2) - 2*l*xc5*sin(q2))^2))/(((cos(q2) + 1)^2*(2*l*xc5 - (2*(-(l^2 + 2*cos(q2)*l*xc1 - 2*sin(q2)*l*xc5 + xc1^2 + xc5^2)*(- 3*l^2 + 2*cos(q2)*l*xc1 - 2*sin(q2)*l*xc5 + xc1^2 + xc5^2))^(1/2))/(cos(q2) + 1) - 4*l^2*tan(q2/2) + 2*l*xc5*tan(q2/2)^2)^2)/(4*(l^2 - 2*l*xc1 + xc1^2 + xc5^2 - 2*l^2*cos(q2) + 2*l*xc1*cos(q2) - 2*l*xc5*sin(q2))^2) + 1)^2 - (2*l*sin(2*atan((2*l^2*sin(q2) + (3*l^4 + 4*cos(q2)*l^3*xc1 - 4*sin(q2)*l^3*xc5 - 2*cos(2*q2)*l^2*xc1^2 + 4*sin(2*q2)*l^2*xc1*xc5 + 2*cos(2*q2)*l^2*xc5^2 - 4*cos(q2)*l*xc1^3 + 4*sin(q2)*l*xc1^2*xc5 - 4*cos(q2)*l*xc1*xc5^2 + 4*sin(q2)*l*xc5^3 - xc1^4 - 2*xc1^2*xc5^2 - xc5^4)^(1/2) - 2*l*xc5)/(l^2 - 2*l*xc1 + xc1^2 + xc5^2 - 2*l^2*cos(q2) + 2*l*xc1*cos(q2) - 2*l*xc5*sin(q2))))*(((- 4*sin(q2)*l^3*xc1 - 4*cos(q2)*l^3*xc5 + 4*sin(2*q2)*l^2*xc1^2 + 8*cos(2*q2)*l^2*xc1*xc5 - 4*sin(2*q2)*l^2*xc5^2 + 4*sin(q2)*l*xc1^3 + 4*cos(q2)*l*xc1^2*xc5 + 4*sin(q2)*l*xc1*xc5^2 + 4*cos(q2)*l*xc5^3)/(2*(3*l^4 + 4*cos(q2)*l^3*xc1 - 4*sin(q2)*l^3*xc5 - 2*cos(2*q2)*l^2*xc1^2 + 4*sin(2*q2)*l^2*xc1*xc5 + 2*cos(2*q2)*l^2*xc5^2 - 4*cos(q2)*l*xc1^3 + 4*sin(q2)*l*xc1^2*xc5 - 4*cos(q2)*l*xc1*xc5^2 + 4*sin(q2)*l*xc5^3 - xc1^4 - 2*xc1^2*xc5^2 - xc5^4)^(1/2)) + 2*l^2*cos(q2))/(l^2 - 2*l*xc1 + xc1^2 + xc5^2 - 2*l^2*cos(q2) + 2*l*xc1*cos(q2) - 2*l*xc5*sin(q2)) + ((2*l*xc5*cos(q2) - 2*l^2*sin(q2) + 2*l*xc1*sin(q2))*(2*l^2*sin(q2) + (3*l^4 + 4*cos(q2)*l^3*xc1 - 4*sin(q2)*l^3*xc5 - 2*cos(2*q2)*l^2*xc1^2 + 4*sin(2*q2)*l^2*xc1*xc5 + 2*cos(2*q2)*l^2*xc5^2 - 4*cos(q2)*l*xc1^3 + 4*sin(q2)*l*xc1^2*xc5 - 4*cos(q2)*l*xc1*xc5^2 + 4*sin(q2)*l*xc5^3 - xc1^4 - 2*xc1^2*xc5^2 - xc5^4)^(1/2) - 2*l*xc5))/(l^2 - 2*l*xc1 + xc1^2 + xc5^2 - 2*l^2*cos(q2) + 2*l*xc1*cos(q2) - 2*l*xc5*sin(q2))^2)*((4*l)/(l^2 - 2*l*xc1 + xc1^2 + xc5^2 - 2*l^2*cos(q2) + 2*l*xc1*cos(q2) - 2*l*xc5*sin(q2)) - ((cos(q2) + 1)*(2*l + 2*l*tan(q2/2)^2 - (4*(sin(q2)*l^3 - 2*cos(q2)*sin(q2)*l^2*xc1 + (1 - 2*cos(q2)^2)*l^2*xc5 - sin(q2)*l*xc1^2 + 2*cos(q2)*l*xc1*xc5 - 3*sin(q2)*l*xc5^2 + xc1^2*xc5 + xc5^3))/((cos(q2) + 1)*(-(l^2 + 2*cos(q2)*l*xc1 - 2*sin(q2)*l*xc5 + xc1^2 + xc5^2)*(- 3*l^2 + 2*cos(q2)*l*xc1 - 2*sin(q2)*l*xc5 + xc1^2 + xc5^2))^(1/2))))/(2*(l^2 - 2*l*xc1 + xc1^2 + xc5^2 - 2*l^2*cos(q2) + 2*l*xc1*cos(q2) - 2*l*xc5*sin(q2))) + ((cos(q2) + 1)^2*(2*xc5*tan(q2/2)^2 - 4*l*tan(q2/2) + 2*xc5)*(2*l*xc5 + (2*(-(l^2 + 2*cos(q2)*l*xc1 - 2*sin(q2)*l*xc5 + xc1^2 + xc5^2)*(- 3*l^2 + 2*cos(q2)*l*xc1 - 2*sin(q2)*l*xc5 + xc1^2 + xc5^2))^(1/2))/(cos(q2) + 1) - 4*l^2*tan(q2/2) + 2*l*xc5*tan(q2/2)^2))/(4*(l^2 - 2*l*xc1 + xc1^2 + xc5^2 - 2*l^2*cos(q2) + 2*l*xc1*cos(q2) - 2*l*xc5*sin(q2))^2) - (l*(cos(q2) + 1)^2*(xc5*tan(q2/2)^2 - 2*l*tan(q2/2) + xc5)*(2*xc5*tan(q2/2)^2 - 4*l*tan(q2/2) + 2*xc5))/(l^2 - 2*l*xc1 + xc1^2 + xc5^2 - 2*l^2*cos(q2) + 2*l*xc1*cos(q2) - 2*l*xc5*sin(q2))^2))/(((2*l^2*sin(q2) + (3*l^4 + 4*cos(q2)*l^3*xc1 - 4*sin(q2)*l^3*xc5 - 2*cos(2*q2)*l^2*xc1^2 + 4*sin(2*q2)*l^2*xc1*xc5 + 2*cos(2*q2)*l^2*xc5^2 - 4*cos(q2)*l*xc1^3 + 4*sin(q2)*l*xc1^2*xc5 - 4*cos(q2)*l*xc1*xc5^2 + 4*sin(q2)*l*xc5^3 - xc1^4 - 2*xc1^2*xc5^2 - xc5^4)^(1/2) - 2*l*xc5)^2/(l^2 - 2*l*xc1 + xc1^2 + xc5^2 - 2*l^2*cos(q2) + 2*l*xc1*cos(q2) - 2*l*xc5*sin(q2))^2 + 1)*(((cos(q2) + 1)^2*(2*l*xc5 - (2*(-(l^2 + 2*cos(q2)*l*xc1 - 2*sin(q2)*l*xc5 + xc1^2 + xc5^2)*(- 3*l^2 + 2*cos(q2)*l*xc1 - 2*sin(q2)*l*xc5 + xc1^2 + xc5^2))^(1/2))/(cos(q2) + 1) - 4*l^2*tan(q2/2) + 2*l*xc5*tan(q2/2)^2)^2)/(4*(l^2 - 2*l*xc1 + xc1^2 + xc5^2 - 2*l^2*cos(q2) + 2*l*xc1*cos(q2) - 2*l*xc5*sin(q2))^2) + 1))), dxc5*((l*cos(2*atan((2*l^2*sin(q2) + (3*l^4 + 4*cos(q2)*l^3*xc1 - 4*sin(q2)*l^3*xc5 - 2*cos(2*q2)*l^2*xc1^2 + 4*sin(2*q2)*l^2*xc1*xc5 + 2*cos(2*q2)*l^2*xc5^2 - 4*cos(q2)*l*xc1^3 + 4*sin(q2)*l*xc1^2*xc5 - 4*cos(q2)*l*xc1*xc5^2 + 4*sin(q2)*l*xc5^3 - xc1^4 - 2*xc1^2*xc5^2 - xc5^4)^(1/2) - 2*l*xc5)/(l^2 - 2*l*xc1 + xc1^2 + xc5^2 - 2*l^2*cos(q2) + 2*l*xc1*cos(q2) - 2*l*xc5*sin(q2))))*(((cos(q2) + 1)*(((cos(q2) + 1)*(((2*xc5*sin(q2/2) - 2*l*cos(q2/2))*(l^2 + 2*cos(q2)*l*xc1 - 2*sin(q2)*l*xc5 + xc1^2 + xc5^2))/cos(q2/2)^5 + ((2*xc5 - 2*l*sin(q2))*(sin(q2/2)*l^2 - 2*sin(q2/2)*l*xc1 - 2*cos(q2/2)*l*xc5 + sin(q2/2)*xc1^2 + sin(q2/2)*xc5^2))/cos(q2/2)^5 - ((2*xc5 - 2*l*sin(q2))*(3*sin(q2/2)*l^2 + 2*sin(q2/2)*l*xc1 + 2*cos(q2/2)*l*xc5 - sin(q2/2)*xc1^2 - sin(q2/2)*xc5^2))/cos(q2/2)^5 + ((2*xc5*sin(q2/2) - 2*l*cos(q2/2))*(- 3*l^2 + 2*cos(q2)*l*xc1 - 2*sin(q2)*l*xc5 + xc1^2 + xc5^2))/cos(q2/2)^5))/(4*(-(l^2 + 2*cos(q2)*l*xc1 - 2*sin(q2)*l*xc5 + xc1^2 + xc5^2)*(- 3*l^2 + 2*cos(q2)*l*xc1 - 2*sin(q2)*l*xc5 + xc1^2 + xc5^2))^(1/2)) - 2*l*tan(q2/2)*(tan(q2/2)^2 + 1) + ((cos(q2) + 1)*(((- 3*l^2 + 2*cos(q2)*l*xc1 - 2*sin(q2)*l*xc5 + xc1^2 + xc5^2)*(sin(q2/2)*l^2 - 2*sin(q2/2)*l*xc1 - 2*cos(q2/2)*l*xc5 + sin(q2/2)*xc1^2 + sin(q2/2)*xc5^2))/cos(q2/2)^5 - ((l^2 + 2*cos(q2)*l*xc1 - 2*sin(q2)*l*xc5 + xc1^2 + xc5^2)*(3*sin(q2/2)*l^2 + 2*sin(q2/2)*l*xc1 + 2*cos(q2/2)*l*xc5 - sin(q2/2)*xc1^2 - sin(q2/2)*xc5^2))/cos(q2/2)^5)*((2*xc5 - 2*l*sin(q2))*(l^2 + 2*cos(q2)*l*xc1 - 2*sin(q2)*l*xc5 + xc1^2 + xc5^2) + (2*xc5 - 2*l*sin(q2))*(- 3*l^2 + 2*cos(q2)*l*xc1 - 2*sin(q2)*l*xc5 + xc1^2 + xc5^2)))/(8*(-(l^2 + 2*cos(q2)*l*xc1 - 2*sin(q2)*l*xc5 + xc1^2 + xc5^2)*(- 3*l^2 + 2*cos(q2)*l*xc1 - 2*sin(q2)*l*xc5 + xc1^2 + xc5^2))^(3/2))))/(2*(l^2 - 2*l*xc1 + xc1^2 + xc5^2 - 2*l^2*cos(q2) + 2*l*xc1*cos(q2) - 2*l*xc5*sin(q2))) - ((cos(q2) + 1)*(2*xc5 - 2*l*sin(q2))*(2*l^2*(tan(q2/2)^2 + 1) + ((cos(q2) + 1)*(((- 3*l^2 + 2*cos(q2)*l*xc1 - 2*sin(q2)*l*xc5 + xc1^2 + xc5^2)*(sin(q2/2)*l^2 - 2*sin(q2/2)*l*xc1 - 2*cos(q2/2)*l*xc5 + sin(q2/2)*xc1^2 + sin(q2/2)*xc5^2))/cos(q2/2)^5 - ((l^2 + 2*cos(q2)*l*xc1 - 2*sin(q2)*l*xc5 + xc1^2 + xc5^2)*(3*sin(q2/2)*l^2 + 2*sin(q2/2)*l*xc1 + 2*cos(q2/2)*l*xc5 - sin(q2/2)*xc1^2 - sin(q2/2)*xc5^2))/cos(q2/2)^5))/(4*(-(l^2 + 2*cos(q2)*l*xc1 - 2*sin(q2)*l*xc5 + xc1^2 + xc5^2)*(- 3*l^2 + 2*cos(q2)*l*xc1 - 2*sin(q2)*l*xc5 + xc1^2 + xc5^2))^(1/2)) - 2*l*xc5*tan(q2/2)*(tan(q2/2)^2 + 1)))/(2*(l^2 - 2*l*xc1 + xc1^2 + xc5^2 - 2*l^2*cos(q2) + 2*l*xc1*cos(q2) - 2*l*xc5*sin(q2))^2) + ((cos(q2) + 1)^2*(2*xc5*sin(q2/2) - 2*l*cos(q2/2))*(2*l*xc5 + (2*(-(l^2 + 2*cos(q2)*l*xc1 - 2*sin(q2)*l*xc5 + xc1^2 + xc5^2)*(- 3*l^2 + 2*cos(q2)*l*xc1 - 2*sin(q2)*l*xc5 + xc1^2 + xc5^2))^(1/2))/(cos(q2) + 1) - 4*l^2*tan(q2/2) + 2*l*xc5*tan(q2/2)^2))/(4*cos(q2/2)^3*(l^2 - 2*l*xc1 + xc1^2 + xc5^2 - 2*l^2*cos(q2) + 2*l*xc1*cos(q2) - 2*l*xc5*sin(q2))^2) + (2*l*tan(q2/2)*(tan(q2/2)^2 + 1)*(cos(q2) + 1))/(l^2 - 2*l*xc1 + xc1^2 + xc5^2 - 2*l^2*cos(q2) + 2*l*xc1*cos(q2) - 2*l*xc5*sin(q2)) + ((cos(q2) + 1)^2*(2*l + 2*l*tan(q2/2)^2 - ((2*xc5 - 2*l*sin(q2))*(l^2 + 2*cos(q2)*l*xc1 - 2*sin(q2)*l*xc5 + xc1^2 + xc5^2) + (2*xc5 - 2*l*sin(q2))*(- 3*l^2 + 2*cos(q2)*l*xc1 - 2*sin(q2)*l*xc5 + xc1^2 + xc5^2))/((cos(q2) + 1)*(-(l^2 + 2*cos(q2)*l*xc1 - 2*sin(q2)*l*xc5 + xc1^2 + xc5^2)*(- 3*l^2 + 2*cos(q2)*l*xc1 - 2*sin(q2)*l*xc5 + xc1^2 + xc5^2))^(1/2)))*(3*sin(q2/2)*l^2 - 4*sin(q2/2)*l*xc1 - 2*cos(q2/2)*l*xc5 + sin(q2/2)*xc1^2 + sin(q2/2)*xc5^2))/(4*cos(q2/2)^3*(l^2 - 2*l*xc1 + xc1^2 + xc5^2 - 2*l^2*cos(q2) + 2*l*xc1*cos(q2) - 2*l*xc5*sin(q2))^2) - ((cos(q2) + 1)^2*(2*xc5 - 2*l*sin(q2))*(2*l*xc5 + (2*(-(l^2 + 2*cos(q2)*l*xc1 - 2*sin(q2)*l*xc5 + xc1^2 + xc5^2)*(- 3*l^2 + 2*cos(q2)*l*xc1 - 2*sin(q2)*l*xc5 + xc1^2 + xc5^2))^(1/2))/(cos(q2) + 1) - 4*l^2*tan(q2/2) + 2*l*xc5*tan(q2/2)^2)*(3*sin(q2/2)*l^2 - 4*sin(q2/2)*l*xc1 - 2*cos(q2/2)*l*xc5 + sin(q2/2)*xc1^2 + sin(q2/2)*xc5^2))/(2*cos(q2/2)^3*(l^2 - 2*l*xc1 + xc1^2 + xc5^2 - 2*l^2*cos(q2) + 2*l*xc1*cos(q2) - 2*l*xc5*sin(q2))^3) - (l*(tan(q2/2)^2 + 1)*(cos(q2) + 1)^2*(3*sin(q2/2)*l^2 - 4*sin(q2/2)*l*xc1 - 2*cos(q2/2)*l*xc5 + sin(q2/2)*xc1^2 + sin(q2/2)*xc5^2))/(cos(q2/2)^3*(l^2 - 2*l*xc1 + xc1^2 + xc5^2 - 2*l^2*cos(q2) + 2*l*xc1*cos(q2) - 2*l*xc5*sin(q2))^2) - (l*(cos(q2) + 1)^2*(2*xc5*sin(q2/2) - 2*l*cos(q2/2))*(xc5*tan(q2/2)^2 - 2*l*tan(q2/2) + xc5))/(cos(q2/2)^3*(l^2 - 2*l*xc1 + xc1^2 + xc5^2 - 2*l^2*cos(q2) + 2*l*xc1*cos(q2) - 2*l*xc5*sin(q2))^2) + (2*l*(tan(q2/2)^2 + 1)*(cos(q2) + 1)*(2*xc5 - 2*l*sin(q2))*(l - xc5*tan(q2/2)))/(l^2 - 2*l*xc1 + xc1^2 + xc5^2 - 2*l^2*cos(q2) + 2*l*xc1*cos(q2) - 2*l*xc5*sin(q2))^2 + (2*l*(cos(q2) + 1)^2*(2*xc5 - 2*l*sin(q2))*(xc5*tan(q2/2)^2 - 2*l*tan(q2/2) + xc5)*(3*sin(q2/2)*l^2 - 4*sin(q2/2)*l*xc1 - 2*cos(q2/2)*l*xc5 + sin(q2/2)*xc1^2 + sin(q2/2)*xc5^2))/(cos(q2/2)^3*(l^2 - 2*l*xc1 + xc1^2 + xc5^2 - 2*l^2*cos(q2) + 2*l*xc1*cos(q2) - 2*l*xc5*sin(q2))^3)))/(((cos(q2) + 1)^2*(2*l*xc5 - (2*(-(l^2 + 2*cos(q2)*l*xc1 - 2*sin(q2)*l*xc5 + xc1^2 + xc5^2)*(- 3*l^2 + 2*cos(q2)*l*xc1 - 2*sin(q2)*l*xc5 + xc1^2 + xc5^2))^(1/2))/(cos(q2) + 1) - 4*l^2*tan(q2/2) + 2*l*xc5*tan(q2/2)^2)^2)/(4*(l^2 - 2*l*xc1 + xc1^2 + xc5^2 - 2*l^2*cos(q2) + 2*l*xc1*cos(q2) - 2*l*xc5*sin(q2))^2) + 1) + (l*cos(2*atan((2*l^2*sin(q2) + (3*l^4 + 4*cos(q2)*l^3*xc1 - 4*sin(q2)*l^3*xc5 - 2*cos(2*q2)*l^2*xc1^2 + 4*sin(2*q2)*l^2*xc1*xc5 + 2*cos(2*q2)*l^2*xc5^2 - 4*cos(q2)*l*xc1^3 + 4*sin(q2)*l*xc1^2*xc5 - 4*cos(q2)*l*xc1*xc5^2 + 4*sin(q2)*l*xc5^3 - xc1^4 - 2*xc1^2*xc5^2 - xc5^4)^(1/2) - 2*l*xc5)/(l^2 - 2*l*xc1 + xc1^2 + xc5^2 - 2*l^2*cos(q2) + 2*l*xc1*cos(q2) - 2*l*xc5*sin(q2))))*(((cos(q2) + 1)^2*(2*xc5 - 2*l*sin(q2))*(2*l*xc5 - (2*(-(l^2 + 2*cos(q2)*l*xc1 - 2*sin(q2)*l*xc5 + xc1^2 + xc5^2)*(- 3*l^2 + 2*cos(q2)*l*xc1 - 2*sin(q2)*l*xc5 + xc1^2 + xc5^2))^(1/2))/(cos(q2) + 1) - 4*l^2*tan(q2/2) + 2*l*xc5*tan(q2/2)^2)^2)/(2*(l^2 - 2*l*xc1 + xc1^2 + xc5^2 - 2*l^2*cos(q2) + 2*l*xc1*cos(q2) - 2*l*xc5*sin(q2))^3) - ((cos(q2) + 1)^2*(2*l + 2*l*tan(q2/2)^2 + ((2*xc5 - 2*l*sin(q2))*(l^2 + 2*cos(q2)*l*xc1 - 2*sin(q2)*l*xc5 + xc1^2 + xc5^2) + (2*xc5 - 2*l*sin(q2))*(- 3*l^2 + 2*cos(q2)*l*xc1 - 2*sin(q2)*l*xc5 + xc1^2 + xc5^2))/((cos(q2) + 1)*(-(l^2 + 2*cos(q2)*l*xc1 - 2*sin(q2)*l*xc5 + xc1^2 + xc5^2)*(- 3*l^2 + 2*cos(q2)*l*xc1 - 2*sin(q2)*l*xc5 + xc1^2 + xc5^2))^(1/2)))*(2*l*xc5 - (2*(-(l^2 + 2*cos(q2)*l*xc1 - 2*sin(q2)*l*xc5 + xc1^2 + xc5^2)*(- 3*l^2 + 2*cos(q2)*l*xc1 - 2*sin(q2)*l*xc5 + xc1^2 + xc5^2))^(1/2))/(cos(q2) + 1) - 4*l^2*tan(q2/2) + 2*l*xc5*tan(q2/2)^2))/(2*(l^2 - 2*l*xc1 + xc1^2 + xc5^2 - 2*l^2*cos(q2) + 2*l*xc1*cos(q2) - 2*l*xc5*sin(q2))^2))*(((cos(q2) + 1)*(2*l^2*(tan(q2/2)^2 + 1) + ((cos(q2) + 1)*(((- 3*l^2 + 2*cos(q2)*l*xc1 - 2*sin(q2)*l*xc5 + xc1^2 + xc5^2)*(sin(q2/2)*l^2 - 2*sin(q2/2)*l*xc1 - 2*cos(q2/2)*l*xc5 + sin(q2/2)*xc1^2 + sin(q2/2)*xc5^2))/cos(q2/2)^5 - ((l^2 + 2*cos(q2)*l*xc1 - 2*sin(q2)*l*xc5 + xc1^2 + xc5^2)*(3*sin(q2/2)*l^2 + 2*sin(q2/2)*l*xc1 + 2*cos(q2/2)*l*xc5 - sin(q2/2)*xc1^2 - sin(q2/2)*xc5^2))/cos(q2/2)^5))/(4*(-(l^2 + 2*cos(q2)*l*xc1 - 2*sin(q2)*l*xc5 + xc1^2 + xc5^2)*(- 3*l^2 + 2*cos(q2)*l*xc1 - 2*sin(q2)*l*xc5 + xc1^2 + xc5^2))^(1/2)) - 2*l*xc5*tan(q2/2)*(tan(q2/2)^2 + 1)))/(2*(l^2 - 2*l*xc1 + xc1^2 + xc5^2 - 2*l^2*cos(q2) + 2*l*xc1*cos(q2) - 2*l*xc5*sin(q2))) + ((cos(q2) + 1)^2*(2*l*xc5 + (2*(-(l^2 + 2*cos(q2)*l*xc1 - 2*sin(q2)*l*xc5 + xc1^2 + xc5^2)*(- 3*l^2 + 2*cos(q2)*l*xc1 - 2*sin(q2)*l*xc5 + xc1^2 + xc5^2))^(1/2))/(cos(q2) + 1) - 4*l^2*tan(q2/2) + 2*l*xc5*tan(q2/2)^2)*(3*sin(q2/2)*l^2 - 4*sin(q2/2)*l*xc1 - 2*cos(q2/2)*l*xc5 + sin(q2/2)*xc1^2 + sin(q2/2)*xc5^2))/(4*cos(q2/2)^3*(l^2 - 2*l*xc1 + xc1^2 + xc5^2 - 2*l^2*cos(q2) + 2*l*xc1*cos(q2) - 2*l*xc5*sin(q2))^2) - (2*l*(tan(q2/2)^2 + 1)*(cos(q2) + 1)*(l - xc5*tan(q2/2)))/(l^2 - 2*l*xc1 + xc1^2 + xc5^2 - 2*l^2*cos(q2) + 2*l*xc1*cos(q2) - 2*l*xc5*sin(q2)) - (l*(cos(q2) + 1)^2*(xc5*tan(q2/2)^2 - 2*l*tan(q2/2) + xc5)*(3*sin(q2/2)*l^2 - 4*sin(q2/2)*l*xc1 - 2*cos(q2/2)*l*xc5 + sin(q2/2)*xc1^2 + sin(q2/2)*xc5^2))/(cos(q2/2)^3*(l^2 - 2*l*xc1 + xc1^2 + xc5^2 - 2*l^2*cos(q2) + 2*l*xc1*cos(q2) - 2*l*xc5*sin(q2))^2)))/(((cos(q2) + 1)^2*(2*l*xc5 - (2*(-(l^2 + 2*cos(q2)*l*xc1 - 2*sin(q2)*l*xc5 + xc1^2 + xc5^2)*(- 3*l^2 + 2*cos(q2)*l*xc1 - 2*sin(q2)*l*xc5 + xc1^2 + xc5^2))^(1/2))/(cos(q2) + 1) - 4*l^2*tan(q2/2) + 2*l*xc5*tan(q2/2)^2)^2)/(4*(l^2 - 2*l*xc1 + xc1^2 + xc5^2 - 2*l^2*cos(q2) + 2*l*xc1*cos(q2) - 2*l*xc5*sin(q2))^2) + 1)^2 + (2*l*sin(2*atan((2*l^2*sin(q2) + (3*l^4 + 4*cos(q2)*l^3*xc1 - 4*sin(q2)*l^3*xc5 - 2*cos(2*q2)*l^2*xc1^2 + 4*sin(2*q2)*l^2*xc1*xc5 + 2*cos(2*q2)*l^2*xc5^2 - 4*cos(q2)*l*xc1^3 + 4*sin(q2)*l*xc1^2*xc5 - 4*cos(q2)*l*xc1*xc5^2 + 4*sin(q2)*l*xc5^3 - xc1^4 - 2*xc1^2*xc5^2 - xc5^4)^(1/2) - 2*l*xc5)/(l^2 - 2*l*xc1 + xc1^2 + xc5^2 - 2*l^2*cos(q2) + 2*l*xc1*cos(q2) - 2*l*xc5*sin(q2))))*((2*l + (4*sin(q2)*l^3 - 4*sin(2*q2)*l^2*xc1 - 4*cos(2*q2)*l^2*xc5 - 4*sin(q2)*l*xc1^2 + 8*cos(q2)*l*xc1*xc5 - 12*sin(q2)*l*xc5^2 + 4*xc1^2*xc5 + 4*xc5^3)/(2*(3*l^4 + 4*cos(q2)*l^3*xc1 - 4*sin(q2)*l^3*xc5 - 2*cos(2*q2)*l^2*xc1^2 + 4*sin(2*q2)*l^2*xc1*xc5 + 2*cos(2*q2)*l^2*xc5^2 - 4*cos(q2)*l*xc1^3 + 4*sin(q2)*l*xc1^2*xc5 - 4*cos(q2)*l*xc1*xc5^2 + 4*sin(q2)*l*xc5^3 - xc1^4 - 2*xc1^2*xc5^2 - xc5^4)^(1/2)))/(l^2 - 2*l*xc1 + xc1^2 + xc5^2 - 2*l^2*cos(q2) + 2*l*xc1*cos(q2) - 2*l*xc5*sin(q2)) + ((2*xc5 - 2*l*sin(q2))*(2*l^2*sin(q2) + (3*l^4 + 4*cos(q2)*l^3*xc1 - 4*sin(q2)*l^3*xc5 - 2*cos(2*q2)*l^2*xc1^2 + 4*sin(2*q2)*l^2*xc1*xc5 + 2*cos(2*q2)*l^2*xc5^2 - 4*cos(q2)*l*xc1^3 + 4*sin(q2)*l*xc1^2*xc5 - 4*cos(q2)*l*xc1*xc5^2 + 4*sin(q2)*l*xc5^3 - xc1^4 - 2*xc1^2*xc5^2 - xc5^4)^(1/2) - 2*l*xc5))/(l^2 - 2*l*xc1 + xc1^2 + xc5^2 - 2*l^2*cos(q2) + 2*l*xc1*cos(q2) - 2*l*xc5*sin(q2))^2)*(((cos(q2) + 1)*(2*l^2*(tan(q2/2)^2 + 1) + ((cos(q2) + 1)*(((- 3*l^2 + 2*cos(q2)*l*xc1 - 2*sin(q2)*l*xc5 + xc1^2 + xc5^2)*(sin(q2/2)*l^2 - 2*sin(q2/2)*l*xc1 - 2*cos(q2/2)*l*xc5 + sin(q2/2)*xc1^2 + sin(q2/2)*xc5^2))/cos(q2/2)^5 - ((l^2 + 2*cos(q2)*l*xc1 - 2*sin(q2)*l*xc5 + xc1^2 + xc5^2)*(3*sin(q2/2)*l^2 + 2*sin(q2/2)*l*xc1 + 2*cos(q2/2)*l*xc5 - sin(q2/2)*xc1^2 - sin(q2/2)*xc5^2))/cos(q2/2)^5))/(4*(-(l^2 + 2*cos(q2)*l*xc1 - 2*sin(q2)*l*xc5 + xc1^2 + xc5^2)*(- 3*l^2 + 2*cos(q2)*l*xc1 - 2*sin(q2)*l*xc5 + xc1^2 + xc5^2))^(1/2)) - 2*l*xc5*tan(q2/2)*(tan(q2/2)^2 + 1)))/(2*(l^2 - 2*l*xc1 + xc1^2 + xc5^2 - 2*l^2*cos(q2) + 2*l*xc1*cos(q2) - 2*l*xc5*sin(q2))) + ((cos(q2) + 1)^2*(2*l*xc5 + (2*(-(l^2 + 2*cos(q2)*l*xc1 - 2*sin(q2)*l*xc5 + xc1^2 + xc5^2)*(- 3*l^2 + 2*cos(q2)*l*xc1 - 2*sin(q2)*l*xc5 + xc1^2 + xc5^2))^(1/2))/(cos(q2) + 1) - 4*l^2*tan(q2/2) + 2*l*xc5*tan(q2/2)^2)*(3*sin(q2/2)*l^2 - 4*sin(q2/2)*l*xc1 - 2*cos(q2/2)*l*xc5 + sin(q2/2)*xc1^2 + sin(q2/2)*xc5^2))/(4*cos(q2/2)^3*(l^2 - 2*l*xc1 + xc1^2 + xc5^2 - 2*l^2*cos(q2) + 2*l*xc1*cos(q2) - 2*l*xc5*sin(q2))^2) - (2*l*(tan(q2/2)^2 + 1)*(cos(q2) + 1)*(l - xc5*tan(q2/2)))/(l^2 - 2*l*xc1 + xc1^2 + xc5^2 - 2*l^2*cos(q2) + 2*l*xc1*cos(q2) - 2*l*xc5*sin(q2)) - (l*(cos(q2) + 1)^2*(xc5*tan(q2/2)^2 - 2*l*tan(q2/2) + xc5)*(3*sin(q2/2)*l^2 - 4*sin(q2/2)*l*xc1 - 2*cos(q2/2)*l*xc5 + sin(q2/2)*xc1^2 + sin(q2/2)*xc5^2))/(cos(q2/2)^3*(l^2 - 2*l*xc1 + xc1^2 + xc5^2 - 2*l^2*cos(q2) + 2*l*xc1*cos(q2) - 2*l*xc5*sin(q2))^2)))/(((2*l^2*sin(q2) + (3*l^4 + 4*cos(q2)*l^3*xc1 - 4*sin(q2)*l^3*xc5 - 2*cos(2*q2)*l^2*xc1^2 + 4*sin(2*q2)*l^2*xc1*xc5 + 2*cos(2*q2)*l^2*xc5^2 - 4*cos(q2)*l*xc1^3 + 4*sin(q2)*l*xc1^2*xc5 - 4*cos(q2)*l*xc1*xc5^2 + 4*sin(q2)*l*xc5^3 - xc1^4 - 2*xc1^2*xc5^2 - xc5^4)^(1/2) - 2*l*xc5)^2/(l^2 - 2*l*xc1 + xc1^2 + xc5^2 - 2*l^2*cos(q2) + 2*l*xc1*cos(q2) - 2*l*xc5*sin(q2))^2 + 1)*(((cos(q2) + 1)^2*(2*l*xc5 - (2*(-(l^2 + 2*cos(q2)*l*xc1 - 2*sin(q2)*l*xc5 + xc1^2 + xc5^2)*(- 3*l^2 + 2*cos(q2)*l*xc1 - 2*sin(q2)*l*xc5 + xc1^2 + xc5^2))^(1/2))/(cos(q2) + 1) - 4*l^2*tan(q2/2) + 2*l*xc5*tan(q2/2)^2)^2)/(4*(l^2 - 2*l*xc1 + xc1^2 + xc5^2 - 2*l^2*cos(q2) + 2*l*xc1*cos(q2) - 2*l*xc5*sin(q2))^2) + 1))) - dq2*(l*sin(q2) - (l*cos(2*atan((2*l^2*sin(q2) + (3*l^4 + 4*cos(q2)*l^3*xc1 - 4*sin(q2)*l^3*xc5 - 2*cos(2*q2)*l^2*xc1^2 + 4*sin(2*q2)*l^2*xc1*xc5 + 2*cos(2*q2)*l^2*xc5^2 - 4*cos(q2)*l*xc1^3 + 4*sin(q2)*l*xc1^2*xc5 - 4*cos(q2)*l*xc1*xc5^2 + 4*sin(q2)*l*xc5^3 - xc1^4 - 2*xc1^2*xc5^2 - xc5^4)^(1/2) - 2*l*xc5)/(l^2 - 2*l*xc1 + xc1^2 + xc5^2 - 2*l^2*cos(q2) + 2*l*xc1*cos(q2) - 2*l*xc5*sin(q2))))*(((cos(q2) + 1)*(2*l^2*(tan(q2/2)^2 + 1) + ((cos(q2) + 1)*(((- 3*l^2 + 2*cos(q2)*l*xc1 - 2*sin(q2)*l*xc5 + xc1^2 + xc5^2)*(sin(q2/2)*l^2 - 2*sin(q2/2)*l*xc1 - 2*cos(q2/2)*l*xc5 + sin(q2/2)*xc1^2 + sin(q2/2)*xc5^2))/cos(q2/2)^5 - ((l^2 + 2*cos(q2)*l*xc1 - 2*sin(q2)*l*xc5 + xc1^2 + xc5^2)*(3*sin(q2/2)*l^2 + 2*sin(q2/2)*l*xc1 + 2*cos(q2/2)*l*xc5 - sin(q2/2)*xc1^2 - sin(q2/2)*xc5^2))/cos(q2/2)^5))/(4*(-(l^2 + 2*cos(q2)*l*xc1 - 2*sin(q2)*l*xc5 + xc1^2 + xc5^2)*(- 3*l^2 + 2*cos(q2)*l*xc1 - 2*sin(q2)*l*xc5 + xc1^2 + xc5^2))^(1/2)) - 2*l*xc5*tan(q2/2)*(tan(q2/2)^2 + 1))*(2*l*xc5*cos(q2) - 2*l^2*sin(q2) + 2*l*xc1*sin(q2)))/(2*(l^2 - 2*l*xc1 + xc1^2 + xc5^2 - 2*l^2*cos(q2) + 2*l*xc1*cos(q2) - 2*l*xc5*sin(q2))^2) - ((cos(q2) + 1)*((sin(q2)*(((- 3*l^2 + 2*cos(q2)*l*xc1 - 2*sin(q2)*l*xc5 + xc1^2 + xc5^2)*(sin(q2/2)*l^2 - 2*sin(q2/2)*l*xc1 - 2*cos(q2/2)*l*xc5 + sin(q2/2)*xc1^2 + sin(q2/2)*xc5^2))/cos(q2/2)^5 - ((l^2 + 2*cos(q2)*l*xc1 - 2*sin(q2)*l*xc5 + xc1^2 + xc5^2)*(3*sin(q2/2)*l^2 + 2*sin(q2/2)*l*xc1 + 2*cos(q2/2)*l*xc5 - sin(q2/2)*xc1^2 - sin(q2/2)*xc5^2))/cos(q2/2)^5))/(4*(-(l^2 + 2*cos(q2)*l*xc1 - 2*sin(q2)*l*xc5 + xc1^2 + xc5^2)*(- 3*l^2 + 2*cos(q2)*l*xc1 - 2*sin(q2)*l*xc5 + xc1^2 + xc5^2))^(1/2)) - 4*l^2*tan(q2/2)*(tan(q2/2)^2/2 + 1/2) - ((cos(q2) + 1)*(((- 3*l^2 + 2*cos(q2)*l*xc1 - 2*sin(q2)*l*xc5 + xc1^2 + xc5^2)*((cos(q2/2)*l^2)/2 - cos(q2/2)*l*xc1 + sin(q2/2)*l*xc5 + (cos(q2/2)*xc1^2)/2 + (cos(q2/2)*xc5^2)/2))/cos(q2/2)^5 - ((2*l*xc5*cos(q2) + 2*l*xc1*sin(q2))*(sin(q2/2)*l^2 - 2*sin(q2/2)*l*xc1 - 2*cos(q2/2)*l*xc5 + sin(q2/2)*xc1^2 + sin(q2/2)*xc5^2))/cos(q2/2)^5 + ((2*l*xc5*cos(q2) + 2*l*xc1*sin(q2))*(3*sin(q2/2)*l^2 + 2*sin(q2/2)*l*xc1 + 2*cos(q2/2)*l*xc5 - sin(q2/2)*xc1^2 - sin(q2/2)*xc5^2))/cos(q2/2)^5 + ((l^2 + 2*cos(q2)*l*xc1 - 2*sin(q2)*l*xc5 + xc1^2 + xc5^2)*(- (3*cos(q2/2)*l^2)/2 - cos(q2/2)*l*xc1 + sin(q2/2)*l*xc5 + (cos(q2/2)*xc1^2)/2 + (cos(q2/2)*xc5^2)/2))/cos(q2/2)^5 - (5*sin(q2/2)*(l^2 + 2*cos(q2)*l*xc1 - 2*sin(q2)*l*xc5 + xc1^2 + xc5^2)*(3*sin(q2/2)*l^2 + 2*sin(q2/2)*l*xc1 + 2*cos(q2/2)*l*xc5 - sin(q2/2)*xc1^2 - sin(q2/2)*xc5^2))/(2*cos(q2/2)^6) + (5*sin(q2/2)*(- 3*l^2 + 2*cos(q2)*l*xc1 - 2*sin(q2)*l*xc5 + xc1^2 + xc5^2)*(sin(q2/2)*l^2 - 2*sin(q2/2)*l*xc1 - 2*cos(q2/2)*l*xc5 + sin(q2/2)*xc1^2 + sin(q2/2)*xc5^2))/(2*cos(q2/2)^6)))/(4*(-(l^2 + 2*cos(q2)*l*xc1 - 2*sin(q2)*l*xc5 + xc1^2 + xc5^2)*(- 3*l^2 + 2*cos(q2)*l*xc1 - 2*sin(q2)*l*xc5 + xc1^2 + xc5^2))^(1/2)) + ((cos(q2) + 1)*(((- 3*l^2 + 2*cos(q2)*l*xc1 - 2*sin(q2)*l*xc5 + xc1^2 + xc5^2)*(sin(q2/2)*l^2 - 2*sin(q2/2)*l*xc1 - 2*cos(q2/2)*l*xc5 + sin(q2/2)*xc1^2 + sin(q2/2)*xc5^2))/cos(q2/2)^5 - ((l^2 + 2*cos(q2)*l*xc1 - 2*sin(q2)*l*xc5 + xc1^2 + xc5^2)*(3*sin(q2/2)*l^2 + 2*sin(q2/2)*l*xc1 + 2*cos(q2/2)*l*xc5 - sin(q2/2)*xc1^2 - sin(q2/2)*xc5^2))/cos(q2/2)^5)*((2*l*xc5*cos(q2) + 2*l*xc1*sin(q2))*(l^2 + 2*cos(q2)*l*xc1 - 2*sin(q2)*l*xc5 + xc1^2 + xc5^2) + (2*l*xc5*cos(q2) + 2*l*xc1*sin(q2))*(- 3*l^2 + 2*cos(q2)*l*xc1 - 2*sin(q2)*l*xc5 + xc1^2 + xc5^2)))/(8*(-(l^2 + 2*cos(q2)*l*xc1 - 2*sin(q2)*l*xc5 + xc1^2 + xc5^2)*(- 3*l^2 + 2*cos(q2)*l*xc1 - 2*sin(q2)*l*xc5 + xc1^2 + xc5^2))^(3/2)) + 4*l*xc5*tan(q2/2)^2*(tan(q2/2)^2/2 + 1/2) + 2*l*xc5*(tan(q2/2)^2 + 1)*(tan(q2/2)^2/2 + 1/2)))/(2*(l^2 - 2*l*xc1 + xc1^2 + xc5^2 - 2*l^2*cos(q2) + 2*l*xc1*cos(q2) - 2*l*xc5*sin(q2))) - (sin(q2)*(2*l^2*(tan(q2/2)^2 + 1) + ((cos(q2) + 1)*(((- 3*l^2 + 2*cos(q2)*l*xc1 - 2*sin(q2)*l*xc5 + xc1^2 + xc5^2)*(sin(q2/2)*l^2 - 2*sin(q2/2)*l*xc1 - 2*cos(q2/2)*l*xc5 + sin(q2/2)*xc1^2 + sin(q2/2)*xc5^2))/cos(q2/2)^5 - ((l^2 + 2*cos(q2)*l*xc1 - 2*sin(q2)*l*xc5 + xc1^2 + xc5^2)*(3*sin(q2/2)*l^2 + 2*sin(q2/2)*l*xc1 + 2*cos(q2/2)*l*xc5 - sin(q2/2)*xc1^2 - sin(q2/2)*xc5^2))/cos(q2/2)^5))/(4*(-(l^2 + 2*cos(q2)*l*xc1 - 2*sin(q2)*l*xc5 + xc1^2 + xc5^2)*(- 3*l^2 + 2*cos(q2)*l*xc1 - 2*sin(q2)*l*xc5 + xc1^2 + xc5^2))^(1/2)) - 2*l*xc5*tan(q2/2)*(tan(q2/2)^2 + 1)))/(2*(l^2 - 2*l*xc1 + xc1^2 + xc5^2 - 2*l^2*cos(q2) + 2*l*xc1*cos(q2) - 2*l*xc5*sin(q2))) + ((cos(q2) + 1)^2*(2*l*xc5 + (2*(-(l^2 + 2*cos(q2)*l*xc1 - 2*sin(q2)*l*xc5 + xc1^2 + xc5^2)*(- 3*l^2 + 2*cos(q2)*l*xc1 - 2*sin(q2)*l*xc5 + xc1^2 + xc5^2))^(1/2))/(cos(q2) + 1) - 4*l^2*tan(q2/2) + 2*l*xc5*tan(q2/2)^2)*((3*cos(q2/2)*l^2)/2 - 2*cos(q2/2)*l*xc1 + sin(q2/2)*l*xc5 + (cos(q2/2)*xc1^2)/2 + (cos(q2/2)*xc5^2)/2))/(4*cos(q2/2)^3*(l^2 - 2*l*xc1 + xc1^2 + xc5^2 - 2*l^2*cos(q2) + 2*l*xc1*cos(q2) - 2*l*xc5*sin(q2))^2) + ((cos(q2) + 1)^2*((2*sin(q2)*(-(l^2 + 2*cos(q2)*l*xc1 - 2*sin(q2)*l*xc5 + xc1^2 + xc5^2)*(- 3*l^2 + 2*cos(q2)*l*xc1 - 2*sin(q2)*l*xc5 + xc1^2 + xc5^2))^(1/2))/(cos(q2) + 1)^2 - 4*l^2*(tan(q2/2)^2/2 + 1/2) + ((2*l*xc5*cos(q2) + 2*l*xc1*sin(q2))*(l^2 + 2*cos(q2)*l*xc1 - 2*sin(q2)*l*xc5 + xc1^2 + xc5^2) + (2*l*xc5*cos(q2) + 2*l*xc1*sin(q2))*(- 3*l^2 + 2*cos(q2)*l*xc1 - 2*sin(q2)*l*xc5 + xc1^2 + xc5^2))/((cos(q2) + 1)*(-(l^2 + 2*cos(q2)*l*xc1 - 2*sin(q2)*l*xc5 + xc1^2 + xc5^2)*(- 3*l^2 + 2*cos(q2)*l*xc1 - 2*sin(q2)*l*xc5 + xc1^2 + xc5^2))^(1/2)) + 4*l*xc5*tan(q2/2)*(tan(q2/2)^2/2 + 1/2))*(3*sin(q2/2)*l^2 - 4*sin(q2/2)*l*xc1 - 2*cos(q2/2)*l*xc5 + sin(q2/2)*xc1^2 + sin(q2/2)*xc5^2))/(4*cos(q2/2)^3*(l^2 - 2*l*xc1 + xc1^2 + xc5^2 - 2*l^2*cos(q2) + 2*l*xc1*cos(q2) - 2*l*xc5*sin(q2))^2) + (2*l*sin(q2)*(tan(q2/2)^2 + 1)*(l - xc5*tan(q2/2)))/(l^2 - 2*l*xc1 + xc1^2 + xc5^2 - 2*l^2*cos(q2) + 2*l*xc1*cos(q2) - 2*l*xc5*sin(q2)) - (4*l*tan(q2/2)*(cos(q2) + 1)*(tan(q2/2)^2/2 + 1/2)*(l - xc5*tan(q2/2)))/(l^2 - 2*l*xc1 + xc1^2 + xc5^2 - 2*l^2*cos(q2) + 2*l*xc1*cos(q2) - 2*l*xc5*sin(q2)) - (2*l*(tan(q2/2)^2 + 1)*(cos(q2) + 1)*(l - xc5*tan(q2/2))*(2*l*xc5*cos(q2) - 2*l^2*sin(q2) + 2*l*xc1*sin(q2)))/(l^2 - 2*l*xc1 + xc1^2 + xc5^2 - 2*l^2*cos(q2) + 2*l*xc1*cos(q2) - 2*l*xc5*sin(q2))^2 + (l*(2*l*(tan(q2/2)^2/2 + 1/2) - 2*xc5*tan(q2/2)*(tan(q2/2)^2/2 + 1/2))*(cos(q2) + 1)^2*(3*sin(q2/2)*l^2 - 4*sin(q2/2)*l*xc1 - 2*cos(q2/2)*l*xc5 + sin(q2/2)*xc1^2 + sin(q2/2)*xc5^2))/(cos(q2/2)^3*(l^2 - 2*l*xc1 + xc1^2 + xc5^2 - 2*l^2*cos(q2) + 2*l*xc1*cos(q2) - 2*l*xc5*sin(q2))^2) + (3*sin(q2/2)*(cos(q2) + 1)^2*(2*l*xc5 + (2*(-(l^2 + 2*cos(q2)*l*xc1 - 2*sin(q2)*l*xc5 + xc1^2 + xc5^2)*(- 3*l^2 + 2*cos(q2)*l*xc1 - 2*sin(q2)*l*xc5 + xc1^2 + xc5^2))^(1/2))/(cos(q2) + 1) - 4*l^2*tan(q2/2) + 2*l*xc5*tan(q2/2)^2)*(3*sin(q2/2)*l^2 - 4*sin(q2/2)*l*xc1 - 2*cos(q2/2)*l*xc5 + sin(q2/2)*xc1^2 + sin(q2/2)*xc5^2))/(8*cos(q2/2)^4*(l^2 - 2*l*xc1 + xc1^2 + xc5^2 - 2*l^2*cos(q2) + 2*l*xc1*cos(q2) - 2*l*xc5*sin(q2))^2) + (2*l*xc5*(tan(q2/2)^2 + 1)*(cos(q2) + 1)*(tan(q2/2)^2/2 + 1/2))/(l^2 - 2*l*xc1 + xc1^2 + xc5^2 - 2*l^2*cos(q2) + 2*l*xc1*cos(q2) - 2*l*xc5*sin(q2)) - (l*(cos(q2) + 1)^2*(xc5*tan(q2/2)^2 - 2*l*tan(q2/2) + xc5)*((3*cos(q2/2)*l^2)/2 - 2*cos(q2/2)*l*xc1 + sin(q2/2)*l*xc5 + (cos(q2/2)*xc1^2)/2 + (cos(q2/2)*xc5^2)/2))/(cos(q2/2)^3*(l^2 - 2*l*xc1 + xc1^2 + xc5^2 - 2*l^2*cos(q2) + 2*l*xc1*cos(q2) - 2*l*xc5*sin(q2))^2) - (sin(q2)*(cos(q2) + 1)*(2*l*xc5 + (2*(-(l^2 + 2*cos(q2)*l*xc1 - 2*sin(q2)*l*xc5 + xc1^2 + xc5^2)*(- 3*l^2 + 2*cos(q2)*l*xc1 - 2*sin(q2)*l*xc5 + xc1^2 + xc5^2))^(1/2))/(cos(q2) + 1) - 4*l^2*tan(q2/2) + 2*l*xc5*tan(q2/2)^2)*(3*sin(q2/2)*l^2 - 4*sin(q2/2)*l*xc1 - 2*cos(q2/2)*l*xc5 + sin(q2/2)*xc1^2 + sin(q2/2)*xc5^2))/(2*cos(q2/2)^3*(l^2 - 2*l*xc1 + xc1^2 + xc5^2 - 2*l^2*cos(q2) + 2*l*xc1*cos(q2) - 2*l*xc5*sin(q2))^2) + ((cos(q2) + 1)^2*(2*l*xc5*cos(q2) - 2*l^2*sin(q2) + 2*l*xc1*sin(q2))*(2*l*xc5 + (2*(-(l^2 + 2*cos(q2)*l*xc1 - 2*sin(q2)*l*xc5 + xc1^2 + xc5^2)*(- 3*l^2 + 2*cos(q2)*l*xc1 - 2*sin(q2)*l*xc5 + xc1^2 + xc5^2))^(1/2))/(cos(q2) + 1) - 4*l^2*tan(q2/2) + 2*l*xc5*tan(q2/2)^2)*(3*sin(q2/2)*l^2 - 4*sin(q2/2)*l*xc1 - 2*cos(q2/2)*l*xc5 + sin(q2/2)*xc1^2 + sin(q2/2)*xc5^2))/(2*cos(q2/2)^3*(l^2 - 2*l*xc1 + xc1^2 + xc5^2 - 2*l^2*cos(q2) + 2*l*xc1*cos(q2) - 2*l*xc5*sin(q2))^3) - (3*l*sin(q2/2)*(cos(q2) + 1)^2*(xc5*tan(q2/2)^2 - 2*l*tan(q2/2) + xc5)*(3*sin(q2/2)*l^2 - 4*sin(q2/2)*l*xc1 - 2*cos(q2/2)*l*xc5 + sin(q2/2)*xc1^2 + sin(q2/2)*xc5^2))/(2*cos(q2/2)^4*(l^2 - 2*l*xc1 + xc1^2 + xc5^2 - 2*l^2*cos(q2) + 2*l*xc1*cos(q2) - 2*l*xc5*sin(q2))^2) + (2*l*sin(q2)*(cos(q2) + 1)*(xc5*tan(q2/2)^2 - 2*l*tan(q2/2) + xc5)*(3*sin(q2/2)*l^2 - 4*sin(q2/2)*l*xc1 - 2*cos(q2/2)*l*xc5 + sin(q2/2)*xc1^2 + sin(q2/2)*xc5^2))/(cos(q2/2)^3*(l^2 - 2*l*xc1 + xc1^2 + xc5^2 - 2*l^2*cos(q2) + 2*l*xc1*cos(q2) - 2*l*xc5*sin(q2))^2) - (2*l*(cos(q2) + 1)^2*(xc5*tan(q2/2)^2 - 2*l*tan(q2/2) + xc5)*(2*l*xc5*cos(q2) - 2*l^2*sin(q2) + 2*l*xc1*sin(q2))*(3*sin(q2/2)*l^2 - 4*sin(q2/2)*l*xc1 - 2*cos(q2/2)*l*xc5 + sin(q2/2)*xc1^2 + sin(q2/2)*xc5^2))/(cos(q2/2)^3*(l^2 - 2*l*xc1 + xc1^2 + xc5^2 - 2*l^2*cos(q2) + 2*l*xc1*cos(q2) - 2*l*xc5*sin(q2))^3)))/(((cos(q2) + 1)^2*(2*l*xc5 - (2*(-(l^2 + 2*cos(q2)*l*xc1 - 2*sin(q2)*l*xc5 + xc1^2 + xc5^2)*(- 3*l^2 + 2*cos(q2)*l*xc1 - 2*sin(q2)*l*xc5 + xc1^2 + xc5^2))^(1/2))/(cos(q2) + 1) - 4*l^2*tan(q2/2) + 2*l*xc5*tan(q2/2)^2)^2)/(4*(l^2 - 2*l*xc1 + xc1^2 + xc5^2 - 2*l^2*cos(q2) + 2*l*xc1*cos(q2) - 2*l*xc5*sin(q2))^2) + 1) - (l*cos(2*atan((2*l^2*sin(q2) + (3*l^4 + 4*cos(q2)*l^3*xc1 - 4*sin(q2)*l^3*xc5 - 2*cos(2*q2)*l^2*xc1^2 + 4*sin(2*q2)*l^2*xc1*xc5 + 2*cos(2*q2)*l^2*xc5^2 - 4*cos(q2)*l*xc1^3 + 4*sin(q2)*l*xc1^2*xc5 - 4*cos(q2)*l*xc1*xc5^2 + 4*sin(q2)*l*xc5^3 - xc1^4 - 2*xc1^2*xc5^2 - xc5^4)^(1/2) - 2*l*xc5)/(l^2 - 2*l*xc1 + xc1^2 + xc5^2 - 2*l^2*cos(q2) + 2*l*xc1*cos(q2) - 2*l*xc5*sin(q2))))*(((cos(q2) + 1)^2*(4*l^2*(tan(q2/2)^2/2 + 1/2) + (2*sin(q2)*(-(l^2 + 2*cos(q2)*l*xc1 - 2*sin(q2)*l*xc5 + xc1^2 + xc5^2)*(- 3*l^2 + 2*cos(q2)*l*xc1 - 2*sin(q2)*l*xc5 + xc1^2 + xc5^2))^(1/2))/(cos(q2) + 1)^2 + ((2*l*xc5*cos(q2) + 2*l*xc1*sin(q2))*(l^2 + 2*cos(q2)*l*xc1 - 2*sin(q2)*l*xc5 + xc1^2 + xc5^2) + (2*l*xc5*cos(q2) + 2*l*xc1*sin(q2))*(- 3*l^2 + 2*cos(q2)*l*xc1 - 2*sin(q2)*l*xc5 + xc1^2 + xc5^2))/((cos(q2) + 1)*(-(l^2 + 2*cos(q2)*l*xc1 - 2*sin(q2)*l*xc5 + xc1^2 + xc5^2)*(- 3*l^2 + 2*cos(q2)*l*xc1 - 2*sin(q2)*l*xc5 + xc1^2 + xc5^2))^(1/2)) - 4*l*xc5*tan(q2/2)*(tan(q2/2)^2/2 + 1/2))*(2*l*xc5 - (2*(-(l^2 + 2*cos(q2)*l*xc1 - 2*sin(q2)*l*xc5 + xc1^2 + xc5^2)*(- 3*l^2 + 2*cos(q2)*l*xc1 - 2*sin(q2)*l*xc5 + xc1^2 + xc5^2))^(1/2))/(cos(q2) + 1) - 4*l^2*tan(q2/2) + 2*l*xc5*tan(q2/2)^2))/(2*(l^2 - 2*l*xc1 + xc1^2 + xc5^2 - 2*l^2*cos(q2) + 2*l*xc1*cos(q2) - 2*l*xc5*sin(q2))^2) - ((cos(q2) + 1)^2*(2*l*xc5*cos(q2) - 2*l^2*sin(q2) + 2*l*xc1*sin(q2))*(2*l*xc5 - (2*(-(l^2 + 2*cos(q2)*l*xc1 - 2*sin(q2)*l*xc5 + xc1^2 + xc5^2)*(- 3*l^2 + 2*cos(q2)*l*xc1 - 2*sin(q2)*l*xc5 + xc1^2 + xc5^2))^(1/2))/(cos(q2) + 1) - 4*l^2*tan(q2/2) + 2*l*xc5*tan(q2/2)^2)^2)/(2*(l^2 - 2*l*xc1 + xc1^2 + xc5^2 - 2*l^2*cos(q2) + 2*l*xc1*cos(q2) - 2*l*xc5*sin(q2))^3) + (sin(q2)*(cos(q2) + 1)*(2*l*xc5 - (2*(-(l^2 + 2*cos(q2)*l*xc1 - 2*sin(q2)*l*xc5 + xc1^2 + xc5^2)*(- 3*l^2 + 2*cos(q2)*l*xc1 - 2*sin(q2)*l*xc5 + xc1^2 + xc5^2))^(1/2))/(cos(q2) + 1) - 4*l^2*tan(q2/2) + 2*l*xc5*tan(q2/2)^2)^2)/(2*(l^2 - 2*l*xc1 + xc1^2 + xc5^2 - 2*l^2*cos(q2) + 2*l*xc1*cos(q2) - 2*l*xc5*sin(q2))^2))*(((cos(q2) + 1)*(2*l^2*(tan(q2/2)^2 + 1) + ((cos(q2) + 1)*(((- 3*l^2 + 2*cos(q2)*l*xc1 - 2*sin(q2)*l*xc5 + xc1^2 + xc5^2)*(sin(q2/2)*l^2 - 2*sin(q2/2)*l*xc1 - 2*cos(q2/2)*l*xc5 + sin(q2/2)*xc1^2 + sin(q2/2)*xc5^2))/cos(q2/2)^5 - ((l^2 + 2*cos(q2)*l*xc1 - 2*sin(q2)*l*xc5 + xc1^2 + xc5^2)*(3*sin(q2/2)*l^2 + 2*sin(q2/2)*l*xc1 + 2*cos(q2/2)*l*xc5 - sin(q2/2)*xc1^2 - sin(q2/2)*xc5^2))/cos(q2/2)^5))/(4*(-(l^2 + 2*cos(q2)*l*xc1 - 2*sin(q2)*l*xc5 + xc1^2 + xc5^2)*(- 3*l^2 + 2*cos(q2)*l*xc1 - 2*sin(q2)*l*xc5 + xc1^2 + xc5^2))^(1/2)) - 2*l*xc5*tan(q2/2)*(tan(q2/2)^2 + 1)))/(2*(l^2 - 2*l*xc1 + xc1^2 + xc5^2 - 2*l^2*cos(q2) + 2*l*xc1*cos(q2) - 2*l*xc5*sin(q2))) + ((cos(q2) + 1)^2*(2*l*xc5 + (2*(-(l^2 + 2*cos(q2)*l*xc1 - 2*sin(q2)*l*xc5 + xc1^2 + xc5^2)*(- 3*l^2 + 2*cos(q2)*l*xc1 - 2*sin(q2)*l*xc5 + xc1^2 + xc5^2))^(1/2))/(cos(q2) + 1) - 4*l^2*tan(q2/2) + 2*l*xc5*tan(q2/2)^2)*(3*sin(q2/2)*l^2 - 4*sin(q2/2)*l*xc1 - 2*cos(q2/2)*l*xc5 + sin(q2/2)*xc1^2 + sin(q2/2)*xc5^2))/(4*cos(q2/2)^3*(l^2 - 2*l*xc1 + xc1^2 + xc5^2 - 2*l^2*cos(q2) + 2*l*xc1*cos(q2) - 2*l*xc5*sin(q2))^2) - (2*l*(tan(q2/2)^2 + 1)*(cos(q2) + 1)*(l - xc5*tan(q2/2)))/(l^2 - 2*l*xc1 + xc1^2 + xc5^2 - 2*l^2*cos(q2) + 2*l*xc1*cos(q2) - 2*l*xc5*sin(q2)) - (l*(cos(q2) + 1)^2*(xc5*tan(q2/2)^2 - 2*l*tan(q2/2) + xc5)*(3*sin(q2/2)*l^2 - 4*sin(q2/2)*l*xc1 - 2*cos(q2/2)*l*xc5 + sin(q2/2)*xc1^2 + sin(q2/2)*xc5^2))/(cos(q2/2)^3*(l^2 - 2*l*xc1 + xc1^2 + xc5^2 - 2*l^2*cos(q2) + 2*l*xc1*cos(q2) - 2*l*xc5*sin(q2))^2)))/(((cos(q2) + 1)^2*(2*l*xc5 - (2*(-(l^2 + 2*cos(q2)*l*xc1 - 2*sin(q2)*l*xc5 + xc1^2 + xc5^2)*(- 3*l^2 + 2*cos(q2)*l*xc1 - 2*sin(q2)*l*xc5 + xc1^2 + xc5^2))^(1/2))/(cos(q2) + 1) - 4*l^2*tan(q2/2) + 2*l*xc5*tan(q2/2)^2)^2)/(4*(l^2 - 2*l*xc1 + xc1^2 + xc5^2 - 2*l^2*cos(q2) + 2*l*xc1*cos(q2) - 2*l*xc5*sin(q2))^2) + 1)^2 + (2*l*sin(2*atan((2*l^2*sin(q2) + (3*l^4 + 4*cos(q2)*l^3*xc1 - 4*sin(q2)*l^3*xc5 - 2*cos(2*q2)*l^2*xc1^2 + 4*sin(2*q2)*l^2*xc1*xc5 + 2*cos(2*q2)*l^2*xc5^2 - 4*cos(q2)*l*xc1^3 + 4*sin(q2)*l*xc1^2*xc5 - 4*cos(q2)*l*xc1*xc5^2 + 4*sin(q2)*l*xc5^3 - xc1^4 - 2*xc1^2*xc5^2 - xc5^4)^(1/2) - 2*l*xc5)/(l^2 - 2*l*xc1 + xc1^2 + xc5^2 - 2*l^2*cos(q2) + 2*l*xc1*cos(q2) - 2*l*xc5*sin(q2))))*(((- 4*sin(q2)*l^3*xc1 - 4*cos(q2)*l^3*xc5 + 4*sin(2*q2)*l^2*xc1^2 + 8*cos(2*q2)*l^2*xc1*xc5 - 4*sin(2*q2)*l^2*xc5^2 + 4*sin(q2)*l*xc1^3 + 4*cos(q2)*l*xc1^2*xc5 + 4*sin(q2)*l*xc1*xc5^2 + 4*cos(q2)*l*xc5^3)/(2*(3*l^4 + 4*cos(q2)*l^3*xc1 - 4*sin(q2)*l^3*xc5 - 2*cos(2*q2)*l^2*xc1^2 + 4*sin(2*q2)*l^2*xc1*xc5 + 2*cos(2*q2)*l^2*xc5^2 - 4*cos(q2)*l*xc1^3 + 4*sin(q2)*l*xc1^2*xc5 - 4*cos(q2)*l*xc1*xc5^2 + 4*sin(q2)*l*xc5^3 - xc1^4 - 2*xc1^2*xc5^2 - xc5^4)^(1/2)) + 2*l^2*cos(q2))/(l^2 - 2*l*xc1 + xc1^2 + xc5^2 - 2*l^2*cos(q2) + 2*l*xc1*cos(q2) - 2*l*xc5*sin(q2)) + ((2*l*xc5*cos(q2) - 2*l^2*sin(q2) + 2*l*xc1*sin(q2))*(2*l^2*sin(q2) + (3*l^4 + 4*cos(q2)*l^3*xc1 - 4*sin(q2)*l^3*xc5 - 2*cos(2*q2)*l^2*xc1^2 + 4*sin(2*q2)*l^2*xc1*xc5 + 2*cos(2*q2)*l^2*xc5^2 - 4*cos(q2)*l*xc1^3 + 4*sin(q2)*l*xc1^2*xc5 - 4*cos(q2)*l*xc1*xc5^2 + 4*sin(q2)*l*xc5^3 - xc1^4 - 2*xc1^2*xc5^2 - xc5^4)^(1/2) - 2*l*xc5))/(l^2 - 2*l*xc1 + xc1^2 + xc5^2 - 2*l^2*cos(q2) + 2*l*xc1*cos(q2) - 2*l*xc5*sin(q2))^2)*(((cos(q2) + 1)*(2*l^2*(tan(q2/2)^2 + 1) + ((cos(q2) + 1)*(((- 3*l^2 + 2*cos(q2)*l*xc1 - 2*sin(q2)*l*xc5 + xc1^2 + xc5^2)*(sin(q2/2)*l^2 - 2*sin(q2/2)*l*xc1 - 2*cos(q2/2)*l*xc5 + sin(q2/2)*xc1^2 + sin(q2/2)*xc5^2))/cos(q2/2)^5 - ((l^2 + 2*cos(q2)*l*xc1 - 2*sin(q2)*l*xc5 + xc1^2 + xc5^2)*(3*sin(q2/2)*l^2 + 2*sin(q2/2)*l*xc1 + 2*cos(q2/2)*l*xc5 - sin(q2/2)*xc1^2 - sin(q2/2)*xc5^2))/cos(q2/2)^5))/(4*(-(l^2 + 2*cos(q2)*l*xc1 - 2*sin(q2)*l*xc5 + xc1^2 + xc5^2)*(- 3*l^2 + 2*cos(q2)*l*xc1 - 2*sin(q2)*l*xc5 + xc1^2 + xc5^2))^(1/2)) - 2*l*xc5*tan(q2/2)*(tan(q2/2)^2 + 1)))/(2*(l^2 - 2*l*xc1 + xc1^2 + xc5^2 - 2*l^2*cos(q2) + 2*l*xc1*cos(q2) - 2*l*xc5*sin(q2))) + ((cos(q2) + 1)^2*(2*l*xc5 + (2*(-(l^2 + 2*cos(q2)*l*xc1 - 2*sin(q2)*l*xc5 + xc1^2 + xc5^2)*(- 3*l^2 + 2*cos(q2)*l*xc1 - 2*sin(q2)*l*xc5 + xc1^2 + xc5^2))^(1/2))/(cos(q2) + 1) - 4*l^2*tan(q2/2) + 2*l*xc5*tan(q2/2)^2)*(3*sin(q2/2)*l^2 - 4*sin(q2/2)*l*xc1 - 2*cos(q2/2)*l*xc5 + sin(q2/2)*xc1^2 + sin(q2/2)*xc5^2))/(4*cos(q2/2)^3*(l^2 - 2*l*xc1 + xc1^2 + xc5^2 - 2*l^2*cos(q2) + 2*l*xc1*cos(q2) - 2*l*xc5*sin(q2))^2) - (2*l*(tan(q2/2)^2 + 1)*(cos(q2) + 1)*(l - xc5*tan(q2/2)))/(l^2 - 2*l*xc1 + xc1^2 + xc5^2 - 2*l^2*cos(q2) + 2*l*xc1*cos(q2) - 2*l*xc5*sin(q2)) - (l*(cos(q2) + 1)^2*(xc5*tan(q2/2)^2 - 2*l*tan(q2/2) + xc5)*(3*sin(q2/2)*l^2 - 4*sin(q2/2)*l*xc1 - 2*cos(q2/2)*l*xc5 + sin(q2/2)*xc1^2 + sin(q2/2)*xc5^2))/(cos(q2/2)^3*(l^2 - 2*l*xc1 + xc1^2 + xc5^2 - 2*l^2*cos(q2) + 2*l*xc1*cos(q2) - 2*l*xc5*sin(q2))^2)))/(((2*l^2*sin(q2) + (3*l^4 + 4*cos(q2)*l^3*xc1 - 4*sin(q2)*l^3*xc5 - 2*cos(2*q2)*l^2*xc1^2 + 4*sin(2*q2)*l^2*xc1*xc5 + 2*cos(2*q2)*l^2*xc5^2 - 4*cos(q2)*l*xc1^3 + 4*sin(q2)*l*xc1^2*xc5 - 4*cos(q2)*l*xc1*xc5^2 + 4*sin(q2)*l*xc5^3 - xc1^4 - 2*xc1^2*xc5^2 - xc5^4)^(1/2) - 2*l*xc5)^2/(l^2 - 2*l*xc1 + xc1^2 + xc5^2 - 2*l^2*cos(q2) + 2*l*xc1*cos(q2) - 2*l*xc5*sin(q2))^2 + 1)*(((cos(q2) + 1)^2*(2*l*xc5 - (2*(-(l^2 + 2*cos(q2)*l*xc1 - 2*sin(q2)*l*xc5 + xc1^2 + xc5^2)*(- 3*l^2 + 2*cos(q2)*l*xc1 - 2*sin(q2)*l*xc5 + xc1^2 + xc5^2))^(1/2))/(cos(q2) + 1) - 4*l^2*tan(q2/2) + 2*l*xc5*tan(q2/2)^2)^2)/(4*(l^2 - 2*l*xc1 + xc1^2 + xc5^2 - 2*l^2*cos(q2) + 2*l*xc1*cos(q2) - 2*l*xc5*sin(q2))^2) + 1))) + dxc1*((l*cos(2*atan((2*l^2*sin(q2) + (3*l^4 + 4*cos(q2)*l^3*xc1 - 4*sin(q2)*l^3*xc5 - 2*cos(2*q2)*l^2*xc1^2 + 4*sin(2*q2)*l^2*xc1*xc5 + 2*cos(2*q2)*l^2*xc5^2 - 4*cos(q2)*l*xc1^3 + 4*sin(q2)*l*xc1^2*xc5 - 4*cos(q2)*l*xc1*xc5^2 + 4*sin(q2)*l*xc5^3 - xc1^4 - 2*xc1^2*xc5^2 - xc5^4)^(1/2) - 2*l*xc5)/(l^2 - 2*l*xc1 + xc1^2 + xc5^2 - 2*l^2*cos(q2) + 2*l*xc1*cos(q2) - 2*l*xc5*sin(q2))))*(((cos(q2) + 1)^2*(2*xc1 - 2*l + 2*l*cos(q2))*(2*l*xc5 - (2*(-(l^2 + 2*cos(q2)*l*xc1 - 2*sin(q2)*l*xc5 + xc1^2 + xc5^2)*(- 3*l^2 + 2*cos(q2)*l*xc1 - 2*sin(q2)*l*xc5 + xc1^2 + xc5^2))^(1/2))/(cos(q2) + 1) - 4*l^2*tan(q2/2) + 2*l*xc5*tan(q2/2)^2)^2)/(2*(l^2 - 2*l*xc1 + xc1^2 + xc5^2 - 2*l^2*cos(q2) + 2*l*xc1*cos(q2) - 2*l*xc5*sin(q2))^3) - ((cos(q2) + 1)*((2*xc1 + 2*l*cos(q2))*(l^2 + 2*cos(q2)*l*xc1 - 2*sin(q2)*l*xc5 + xc1^2 + xc5^2) + (2*xc1 + 2*l*cos(q2))*(- 3*l^2 + 2*cos(q2)*l*xc1 - 2*sin(q2)*l*xc5 + xc1^2 + xc5^2))*(2*l*xc5 - (2*(-(l^2 + 2*cos(q2)*l*xc1 - 2*sin(q2)*l*xc5 + xc1^2 + xc5^2)*(- 3*l^2 + 2*cos(q2)*l*xc1 - 2*sin(q2)*l*xc5 + xc1^2 + xc5^2))^(1/2))/(cos(q2) + 1) - 4*l^2*tan(q2/2) + 2*l*xc5*tan(q2/2)^2))/(2*(-(l^2 + 2*cos(q2)*l*xc1 - 2*sin(q2)*l*xc5 + xc1^2 + xc5^2)*(- 3*l^2 + 2*cos(q2)*l*xc1 - 2*sin(q2)*l*xc5 + xc1^2 + xc5^2))^(1/2)*(l^2 - 2*l*xc1 + xc1^2 + xc5^2 - 2*l^2*cos(q2) + 2*l*xc1*cos(q2) - 2*l*xc5*sin(q2))^2))*(((cos(q2) + 1)*(2*l^2*(tan(q2/2)^2 + 1) + ((cos(q2) + 1)*(((- 3*l^2 + 2*cos(q2)*l*xc1 - 2*sin(q2)*l*xc5 + xc1^2 + xc5^2)*(sin(q2/2)*l^2 - 2*sin(q2/2)*l*xc1 - 2*cos(q2/2)*l*xc5 + sin(q2/2)*xc1^2 + sin(q2/2)*xc5^2))/cos(q2/2)^5 - ((l^2 + 2*cos(q2)*l*xc1 - 2*sin(q2)*l*xc5 + xc1^2 + xc5^2)*(3*sin(q2/2)*l^2 + 2*sin(q2/2)*l*xc1 + 2*cos(q2/2)*l*xc5 - sin(q2/2)*xc1^2 - sin(q2/2)*xc5^2))/cos(q2/2)^5))/(4*(-(l^2 + 2*cos(q2)*l*xc1 - 2*sin(q2)*l*xc5 + xc1^2 + xc5^2)*(- 3*l^2 + 2*cos(q2)*l*xc1 - 2*sin(q2)*l*xc5 + xc1^2 + xc5^2))^(1/2)) - 2*l*xc5*tan(q2/2)*(tan(q2/2)^2 + 1)))/(2*(l^2 - 2*l*xc1 + xc1^2 + xc5^2 - 2*l^2*cos(q2) + 2*l*xc1*cos(q2) - 2*l*xc5*sin(q2))) + ((cos(q2) + 1)^2*(2*l*xc5 + (2*(-(l^2 + 2*cos(q2)*l*xc1 - 2*sin(q2)*l*xc5 + xc1^2 + xc5^2)*(- 3*l^2 + 2*cos(q2)*l*xc1 - 2*sin(q2)*l*xc5 + xc1^2 + xc5^2))^(1/2))/(cos(q2) + 1) - 4*l^2*tan(q2/2) + 2*l*xc5*tan(q2/2)^2)*(3*sin(q2/2)*l^2 - 4*sin(q2/2)*l*xc1 - 2*cos(q2/2)*l*xc5 + sin(q2/2)*xc1^2 + sin(q2/2)*xc5^2))/(4*cos(q2/2)^3*(l^2 - 2*l*xc1 + xc1^2 + xc5^2 - 2*l^2*cos(q2) + 2*l*xc1*cos(q2) - 2*l*xc5*sin(q2))^2) - (2*l*(tan(q2/2)^2 + 1)*(cos(q2) + 1)*(l - xc5*tan(q2/2)))/(l^2 - 2*l*xc1 + xc1^2 + xc5^2 - 2*l^2*cos(q2) + 2*l*xc1*cos(q2) - 2*l*xc5*sin(q2)) - (l*(cos(q2) + 1)^2*(xc5*tan(q2/2)^2 - 2*l*tan(q2/2) + xc5)*(3*sin(q2/2)*l^2 - 4*sin(q2/2)*l*xc1 - 2*cos(q2/2)*l*xc5 + sin(q2/2)*xc1^2 + sin(q2/2)*xc5^2))/(cos(q2/2)^3*(l^2 - 2*l*xc1 + xc1^2 + xc5^2 - 2*l^2*cos(q2) + 2*l*xc1*cos(q2) - 2*l*xc5*sin(q2))^2)))/(((cos(q2) + 1)^2*(2*l*xc5 - (2*(-(l^2 + 2*cos(q2)*l*xc1 - 2*sin(q2)*l*xc5 + xc1^2 + xc5^2)*(- 3*l^2 + 2*cos(q2)*l*xc1 - 2*sin(q2)*l*xc5 + xc1^2 + xc5^2))^(1/2))/(cos(q2) + 1) - 4*l^2*tan(q2/2) + 2*l*xc5*tan(q2/2)^2)^2)/(4*(l^2 - 2*l*xc1 + xc1^2 + xc5^2 - 2*l^2*cos(q2) + 2*l*xc1*cos(q2) - 2*l*xc5*sin(q2))^2) + 1)^2 - (l*cos(2*atan((2*l^2*sin(q2) + (3*l^4 + 4*cos(q2)*l^3*xc1 - 4*sin(q2)*l^3*xc5 - 2*cos(2*q2)*l^2*xc1^2 + 4*sin(2*q2)*l^2*xc1*xc5 + 2*cos(2*q2)*l^2*xc5^2 - 4*cos(q2)*l*xc1^3 + 4*sin(q2)*l*xc1^2*xc5 - 4*cos(q2)*l*xc1*xc5^2 + 4*sin(q2)*l*xc5^3 - xc1^4 - 2*xc1^2*xc5^2 - xc5^4)^(1/2) - 2*l*xc5)/(l^2 - 2*l*xc1 + xc1^2 + xc5^2 - 2*l^2*cos(q2) + 2*l*xc1*cos(q2) - 2*l*xc5*sin(q2))))*(((cos(q2) + 1)*(((cos(q2) + 1)*(((2*xc1 + 2*l*cos(q2))*(3*sin(q2/2)*l^2 + 2*sin(q2/2)*l*xc1 + 2*cos(q2/2)*l*xc5 - sin(q2/2)*xc1^2 - sin(q2/2)*xc5^2))/cos(q2/2)^5 - ((2*xc1 + 2*l*cos(q2))*(sin(q2/2)*l^2 - 2*sin(q2/2)*l*xc1 - 2*cos(q2/2)*l*xc5 + sin(q2/2)*xc1^2 + sin(q2/2)*xc5^2))/cos(q2/2)^5 + ((2*l*sin(q2/2) - 2*xc1*sin(q2/2))*(l^2 + 2*cos(q2)*l*xc1 - 2*sin(q2)*l*xc5 + xc1^2 + xc5^2))/cos(q2/2)^5 + ((2*l*sin(q2/2) - 2*xc1*sin(q2/2))*(- 3*l^2 + 2*cos(q2)*l*xc1 - 2*sin(q2)*l*xc5 + xc1^2 + xc5^2))/cos(q2/2)^5))/(4*(-(l^2 + 2*cos(q2)*l*xc1 - 2*sin(q2)*l*xc5 + xc1^2 + xc5^2)*(- 3*l^2 + 2*cos(q2)*l*xc1 - 2*sin(q2)*l*xc5 + xc1^2 + xc5^2))^(1/2)) - ((cos(q2) + 1)*(((- 3*l^2 + 2*cos(q2)*l*xc1 - 2*sin(q2)*l*xc5 + xc1^2 + xc5^2)*(sin(q2/2)*l^2 - 2*sin(q2/2)*l*xc1 - 2*cos(q2/2)*l*xc5 + sin(q2/2)*xc1^2 + sin(q2/2)*xc5^2))/cos(q2/2)^5 - ((l^2 + 2*cos(q2)*l*xc1 - 2*sin(q2)*l*xc5 + xc1^2 + xc5^2)*(3*sin(q2/2)*l^2 + 2*sin(q2/2)*l*xc1 + 2*cos(q2/2)*l*xc5 - sin(q2/2)*xc1^2 - sin(q2/2)*xc5^2))/cos(q2/2)^5)*((2*xc1 + 2*l*cos(q2))*(l^2 + 2*cos(q2)*l*xc1 - 2*sin(q2)*l*xc5 + xc1^2 + xc5^2) + (2*xc1 + 2*l*cos(q2))*(- 3*l^2 + 2*cos(q2)*l*xc1 - 2*sin(q2)*l*xc5 + xc1^2 + xc5^2)))/(8*(-(l^2 + 2*cos(q2)*l*xc1 - 2*sin(q2)*l*xc5 + xc1^2 + xc5^2)*(- 3*l^2 + 2*cos(q2)*l*xc1 - 2*sin(q2)*l*xc5 + xc1^2 + xc5^2))^(3/2))))/(2*(l^2 - 2*l*xc1 + xc1^2 + xc5^2 - 2*l^2*cos(q2) + 2*l*xc1*cos(q2) - 2*l*xc5*sin(q2))) + ((cos(q2) + 1)*(2*l^2*(tan(q2/2)^2 + 1) + ((cos(q2) + 1)*(((- 3*l^2 + 2*cos(q2)*l*xc1 - 2*sin(q2)*l*xc5 + xc1^2 + xc5^2)*(sin(q2/2)*l^2 - 2*sin(q2/2)*l*xc1 - 2*cos(q2/2)*l*xc5 + sin(q2/2)*xc1^2 + sin(q2/2)*xc5^2))/cos(q2/2)^5 - ((l^2 + 2*cos(q2)*l*xc1 - 2*sin(q2)*l*xc5 + xc1^2 + xc5^2)*(3*sin(q2/2)*l^2 + 2*sin(q2/2)*l*xc1 + 2*cos(q2/2)*l*xc5 - sin(q2/2)*xc1^2 - sin(q2/2)*xc5^2))/cos(q2/2)^5))/(4*(-(l^2 + 2*cos(q2)*l*xc1 - 2*sin(q2)*l*xc5 + xc1^2 + xc5^2)*(- 3*l^2 + 2*cos(q2)*l*xc1 - 2*sin(q2)*l*xc5 + xc1^2 + xc5^2))^(1/2)) - 2*l*xc5*tan(q2/2)*(tan(q2/2)^2 + 1))*(2*xc1 - 2*l + 2*l*cos(q2)))/(2*(l^2 - 2*l*xc1 + xc1^2 + xc5^2 - 2*l^2*cos(q2) + 2*l*xc1*cos(q2) - 2*l*xc5*sin(q2))^2) + ((cos(q2) + 1)^2*(4*l*sin(q2/2) - 2*xc1*sin(q2/2))*(2*l*xc5 + (2*(-(l^2 + 2*cos(q2)*l*xc1 - 2*sin(q2)*l*xc5 + xc1^2 + xc5^2)*(- 3*l^2 + 2*cos(q2)*l*xc1 - 2*sin(q2)*l*xc5 + xc1^2 + xc5^2))^(1/2))/(cos(q2) + 1) - 4*l^2*tan(q2/2) + 2*l*xc5*tan(q2/2)^2))/(4*cos(q2/2)^3*(l^2 - 2*l*xc1 + xc1^2 + xc5^2 - 2*l^2*cos(q2) + 2*l*xc1*cos(q2) - 2*l*xc5*sin(q2))^2) - (2*l*(tan(q2/2)^2 + 1)*(cos(q2) + 1)*(l - xc5*tan(q2/2))*(2*xc1 - 2*l + 2*l*cos(q2)))/(l^2 - 2*l*xc1 + xc1^2 + xc5^2 - 2*l^2*cos(q2) + 2*l*xc1*cos(q2) - 2*l*xc5*sin(q2))^2 + ((cos(q2) + 1)*((2*xc1 + 2*l*cos(q2))*(l^2 + 2*cos(q2)*l*xc1 - 2*sin(q2)*l*xc5 + xc1^2 + xc5^2) + (2*xc1 + 2*l*cos(q2))*(- 3*l^2 + 2*cos(q2)*l*xc1 - 2*sin(q2)*l*xc5 + xc1^2 + xc5^2))*(3*sin(q2/2)*l^2 - 4*sin(q2/2)*l*xc1 - 2*cos(q2/2)*l*xc5 + sin(q2/2)*xc1^2 + sin(q2/2)*xc5^2))/(4*cos(q2/2)^3*(-(l^2 + 2*cos(q2)*l*xc1 - 2*sin(q2)*l*xc5 + xc1^2 + xc5^2)*(- 3*l^2 + 2*cos(q2)*l*xc1 - 2*sin(q2)*l*xc5 + xc1^2 + xc5^2))^(1/2)*(l^2 - 2*l*xc1 + xc1^2 + xc5^2 - 2*l^2*cos(q2) + 2*l*xc1*cos(q2) - 2*l*xc5*sin(q2))^2) - (l*(cos(q2) + 1)^2*(4*l*sin(q2/2) - 2*xc1*sin(q2/2))*(xc5*tan(q2/2)^2 - 2*l*tan(q2/2) + xc5))/(cos(q2/2)^3*(l^2 - 2*l*xc1 + xc1^2 + xc5^2 - 2*l^2*cos(q2) + 2*l*xc1*cos(q2) - 2*l*xc5*sin(q2))^2) + ((cos(q2) + 1)^2*(2*xc1 - 2*l + 2*l*cos(q2))*(2*l*xc5 + (2*(-(l^2 + 2*cos(q2)*l*xc1 - 2*sin(q2)*l*xc5 + xc1^2 + xc5^2)*(- 3*l^2 + 2*cos(q2)*l*xc1 - 2*sin(q2)*l*xc5 + xc1^2 + xc5^2))^(1/2))/(cos(q2) + 1) - 4*l^2*tan(q2/2) + 2*l*xc5*tan(q2/2)^2)*(3*sin(q2/2)*l^2 - 4*sin(q2/2)*l*xc1 - 2*cos(q2/2)*l*xc5 + sin(q2/2)*xc1^2 + sin(q2/2)*xc5^2))/(2*cos(q2/2)^3*(l^2 - 2*l*xc1 + xc1^2 + xc5^2 - 2*l^2*cos(q2) + 2*l*xc1*cos(q2) - 2*l*xc5*sin(q2))^3) - (2*l*(cos(q2) + 1)^2*(xc5*tan(q2/2)^2 - 2*l*tan(q2/2) + xc5)*(2*xc1 - 2*l + 2*l*cos(q2))*(3*sin(q2/2)*l^2 - 4*sin(q2/2)*l*xc1 - 2*cos(q2/2)*l*xc5 + sin(q2/2)*xc1^2 + sin(q2/2)*xc5^2))/(cos(q2/2)^3*(l^2 - 2*l*xc1 + xc1^2 + xc5^2 - 2*l^2*cos(q2) + 2*l*xc1*cos(q2) - 2*l*xc5*sin(q2))^3)))/(((cos(q2) + 1)^2*(2*l*xc5 - (2*(-(l^2 + 2*cos(q2)*l*xc1 - 2*sin(q2)*l*xc5 + xc1^2 + xc5^2)*(- 3*l^2 + 2*cos(q2)*l*xc1 - 2*sin(q2)*l*xc5 + xc1^2 + xc5^2))^(1/2))/(cos(q2) + 1) - 4*l^2*tan(q2/2) + 2*l*xc5*tan(q2/2)^2)^2)/(4*(l^2 - 2*l*xc1 + xc1^2 + xc5^2 - 2*l^2*cos(q2) + 2*l*xc1*cos(q2) - 2*l*xc5*sin(q2))^2) + 1) + (2*l*sin(2*atan((2*l^2*sin(q2) + (3*l^4 + 4*cos(q2)*l^3*xc1 - 4*sin(q2)*l^3*xc5 - 2*cos(2*q2)*l^2*xc1^2 + 4*sin(2*q2)*l^2*xc1*xc5 + 2*cos(2*q2)*l^2*xc5^2 - 4*cos(q2)*l*xc1^3 + 4*sin(q2)*l*xc1^2*xc5 - 4*cos(q2)*l*xc1*xc5^2 + 4*sin(q2)*l*xc5^3 - xc1^4 - 2*xc1^2*xc5^2 - xc5^4)^(1/2) - 2*l*xc5)/(l^2 - 2*l*xc1 + xc1^2 + xc5^2 - 2*l^2*cos(q2) + 2*l*xc1*cos(q2) - 2*l*xc5*sin(q2))))*(((2*xc1 - 2*l + 2*l*cos(q2))*(2*l^2*sin(q2) + (3*l^4 + 4*cos(q2)*l^3*xc1 - 4*sin(q2)*l^3*xc5 - 2*cos(2*q2)*l^2*xc1^2 + 4*sin(2*q2)*l^2*xc1*xc5 + 2*cos(2*q2)*l^2*xc5^2 - 4*cos(q2)*l*xc1^3 + 4*sin(q2)*l*xc1^2*xc5 - 4*cos(q2)*l*xc1*xc5^2 + 4*sin(q2)*l*xc5^3 - xc1^4 - 2*xc1^2*xc5^2 - xc5^4)^(1/2) - 2*l*xc5))/(l^2 - 2*l*xc1 + xc1^2 + xc5^2 - 2*l^2*cos(q2) + 2*l*xc1*cos(q2) - 2*l*xc5*sin(q2))^2 + (- 4*cos(q2)*l^3 + 4*cos(2*q2)*l^2*xc1 - 4*sin(2*q2)*l^2*xc5 + 12*cos(q2)*l*xc1^2 - 8*sin(q2)*l*xc1*xc5 + 4*cos(q2)*l*xc5^2 + 4*xc1^3 + 4*xc1*xc5^2)/(2*(l^2 - 2*l*xc1 + xc1^2 + xc5^2 - 2*l^2*cos(q2) + 2*l*xc1*cos(q2) - 2*l*xc5*sin(q2))*(3*l^4 + 4*cos(q2)*l^3*xc1 - 4*sin(q2)*l^3*xc5 - 2*cos(2*q2)*l^2*xc1^2 + 4*sin(2*q2)*l^2*xc1*xc5 + 2*cos(2*q2)*l^2*xc5^2 - 4*cos(q2)*l*xc1^3 + 4*sin(q2)*l*xc1^2*xc5 - 4*cos(q2)*l*xc1*xc5^2 + 4*sin(q2)*l*xc5^3 - xc1^4 - 2*xc1^2*xc5^2 - xc5^4)^(1/2)))*(((cos(q2) + 1)*(2*l^2*(tan(q2/2)^2 + 1) + ((cos(q2) + 1)*(((- 3*l^2 + 2*cos(q2)*l*xc1 - 2*sin(q2)*l*xc5 + xc1^2 + xc5^2)*(sin(q2/2)*l^2 - 2*sin(q2/2)*l*xc1 - 2*cos(q2/2)*l*xc5 + sin(q2/2)*xc1^2 + sin(q2/2)*xc5^2))/cos(q2/2)^5 - ((l^2 + 2*cos(q2)*l*xc1 - 2*sin(q2)*l*xc5 + xc1^2 + xc5^2)*(3*sin(q2/2)*l^2 + 2*sin(q2/2)*l*xc1 + 2*cos(q2/2)*l*xc5 - sin(q2/2)*xc1^2 - sin(q2/2)*xc5^2))/cos(q2/2)^5))/(4*(-(l^2 + 2*cos(q2)*l*xc1 - 2*sin(q2)*l*xc5 + xc1^2 + xc5^2)*(- 3*l^2 + 2*cos(q2)*l*xc1 - 2*sin(q2)*l*xc5 + xc1^2 + xc5^2))^(1/2)) - 2*l*xc5*tan(q2/2)*(tan(q2/2)^2 + 1)))/(2*(l^2 - 2*l*xc1 + xc1^2 + xc5^2 - 2*l^2*cos(q2) + 2*l*xc1*cos(q2) - 2*l*xc5*sin(q2))) + ((cos(q2) + 1)^2*(2*l*xc5 + (2*(-(l^2 + 2*cos(q2)*l*xc1 - 2*sin(q2)*l*xc5 + xc1^2 + xc5^2)*(- 3*l^2 + 2*cos(q2)*l*xc1 - 2*sin(q2)*l*xc5 + xc1^2 + xc5^2))^(1/2))/(cos(q2) + 1) - 4*l^2*tan(q2/2) + 2*l*xc5*tan(q2/2)^2)*(3*sin(q2/2)*l^2 - 4*sin(q2/2)*l*xc1 - 2*cos(q2/2)*l*xc5 + sin(q2/2)*xc1^2 + sin(q2/2)*xc5^2))/(4*cos(q2/2)^3*(l^2 - 2*l*xc1 + xc1^2 + xc5^2 - 2*l^2*cos(q2) + 2*l*xc1*cos(q2) - 2*l*xc5*sin(q2))^2) - (2*l*(tan(q2/2)^2 + 1)*(cos(q2) + 1)*(l - xc5*tan(q2/2)))/(l^2 - 2*l*xc1 + xc1^2 + xc5^2 - 2*l^2*cos(q2) + 2*l*xc1*cos(q2) - 2*l*xc5*sin(q2)) - (l*(cos(q2) + 1)^2*(xc5*tan(q2/2)^2 - 2*l*tan(q2/2) + xc5)*(3*sin(q2/2)*l^2 - 4*sin(q2/2)*l*xc1 - 2*cos(q2/2)*l*xc5 + sin(q2/2)*xc1^2 + sin(q2/2)*xc5^2))/(cos(q2/2)^3*(l^2 - 2*l*xc1 + xc1^2 + xc5^2 - 2*l^2*cos(q2) + 2*l*xc1*cos(q2) - 2*l*xc5*sin(q2))^2)))/(((2*l^2*sin(q2) + (3*l^4 + 4*cos(q2)*l^3*xc1 - 4*sin(q2)*l^3*xc5 - 2*cos(2*q2)*l^2*xc1^2 + 4*sin(2*q2)*l^2*xc1*xc5 + 2*cos(2*q2)*l^2*xc5^2 - 4*cos(q2)*l*xc1^3 + 4*sin(q2)*l*xc1^2*xc5 - 4*cos(q2)*l*xc1*xc5^2 + 4*sin(q2)*l*xc5^3 - xc1^4 - 2*xc1^2*xc5^2 - xc5^4)^(1/2) - 2*l*xc5)^2/(l^2 - 2*l*xc1 + xc1^2 + xc5^2 - 2*l^2*cos(q2) + 2*l*xc1*cos(q2) - 2*l*xc5*sin(q2))^2 + 1)*(((cos(q2) + 1)^2*(2*l*xc5 - (2*(-(l^2 + 2*cos(q2)*l*xc1 - 2*sin(q2)*l*xc5 + xc1^2 + xc5^2)*(- 3*l^2 + 2*cos(q2)*l*xc1 - 2*sin(q2)*l*xc5 + xc1^2 + xc5^2))^(1/2))/(cos(q2) + 1) - 4*l^2*tan(q2/2) + 2*l*xc5*tan(q2/2)^2)^2)/(4*(l^2 - 2*l*xc1 + xc1^2 + xc5^2 - 2*l^2*cos(q2) + 2*l*xc1*cos(q2) - 2*l*xc5*sin(q2))^2) + 1)));...
